simulink model "SIM_EXO_DAL_MN"  (R2021b)
(part 10 of 24)

t1657 = ct{497};
t1658 = ct{498};
t1659 = ct{499};
t166 = ct{500};
t1660 = ct{501};
t1661 = ct{502};
t1662 = ct{503};
t1663 = ct{504};
t1666 = ct{505};
t1669 = ct{506};
t1672 = ct{507};
t1676 = ct{508};
t1681 = ct{509};
t1682 = ct{510};
t1683 = ct{511};
t1687 = ct{512};
t1689 = ct{513};
t1692 = ct{514};
t1695 = ct{515};
t1696 = ct{516};
t1698 = ct{517};
t17 = ct{518};
t170 = ct{519};
t1702 = ct{520};
t1703 = ct{521};
t1704 = ct{522};
t1709 = ct{523};
t171 = ct{524};
t1711 = ct{525};
t1712 = ct{526};
t1713 = ct{527};
t1716 = ct{528};
t1720 = ct{529};
t1722 = ct{530};
t1726 = ct{531};
t1728 = ct{532};
t1729 = ct{533};
t173 = ct{534};
t1731 = ct{535};
t1733 = ct{536};
t1734 = ct{537};
t1735 = ct{538};
t1736 = ct{539};
t1737 = ct{540};
t1738 = ct{541};
t1740 = ct{542};
t1744 = ct{543};
t1745 = ct{544};
t1746 = ct{545};
t1749 = ct{546};
t175 = ct{547};
t1752 = ct{548};
t1755 = ct{549};
t1756 = ct{550};
t1757 = ct{551};
t1758 = ct{552};
t1760 = ct{553};
t1761 = ct{554};
t1764 = ct{555};
t1767 = ct{556};
t1769 = ct{557};
t177 = ct{558};
t1771 = ct{559};
t1772 = ct{560};
t1774 = ct{561};
t1776 = ct{562};
t1779 = ct{563};
t1784 = ct{564};
t1785 = ct{565};
t1786 = ct{566};
t1787 = ct{567};
t1788 = ct{568};
t1789 = ct{569};
t1793 = ct{570};
t1795 = ct{571};
t1797 = ct{572};
t1798 = ct{573};
t1799 = ct{574};
t18 = ct{575};
t1800 = ct{576};
t1801 = ct{577};
t1803 = ct{578};
t1804 = ct{579};
t1807 = ct{580};
t1808 = ct{581};
t1809 = ct{582};
t1810 = ct{583};
t1811 = ct{584};
t1812 = ct{585};
t1814 = ct{586};
t1816 = ct{587};
t1817 = ct{588};
t1820 = ct{589};
t1826 = ct{590};
t1827 = ct{591};
t1829 = ct{592};
t183 = ct{593};
t1830 = ct{594};
t1831 = ct{595};
t1832 = ct{596};
t1833 = ct{597};
t1834 = ct{598};
t1835 = ct{599};
t1836 = ct{600};
t1838 = ct{601};
t1847 = ct{602};
t1849 = ct{603};
t185 = ct{604};
t1850 = ct{605};
t1851 = ct{606};
t1855 = ct{607};
t1857 = ct{608};
t1858 = ct{609};
t1859 = ct{610};
t186 = ct{611};
t1866 = ct{612};
t1867 = ct{613};
t1871 = ct{614};
t1872 = ct{615};
t1873 = ct{616};
t1881 = ct{617};
t1882 = ct{618};
t1888 = ct{619};
t1889 = ct{620};
t1896 = ct{621};
t19 = ct{622};
t190 = ct{623};
t1903 = ct{624};
t1907 = ct{625};
t1908 = ct{626};
t191 = ct{627};
t1910 = ct{628};
t1911 = ct{629};
t1912 = ct{630};
t1913 = ct{631};
t1914 = ct{632};
t1915 = ct{633};
t1916 = ct{634};
t1920 = ct{635};
t1925 = ct{636};
t1926 = ct{637};
t193 = ct{638};
t1930 = ct{639};
t1935 = ct{640};
t1936 = ct{641};
t1937 = ct{642};
t1938 = ct{643};
t1939 = ct{644};
t194 = ct{645};
t1943 = ct{646};
t1944 = ct{647};
t1946 = ct{648};
t195 = ct{649};
t1950 = ct{650};
t1955 = ct{651};
t196 = ct{652};
t1961 = ct{653};
t1964 = ct{654};
t1965 = ct{655};
t1966 = ct{656};
t1967 = ct{657};
t1968 = ct{658};
t1969 = ct{659};
t197 = ct{660};
t1970 = ct{661};
t1972 = ct{662};
t1976 = ct{663};
t1977 = ct{664};
t1978 = ct{665};
t1979 = ct{666};
t1981 = ct{667};
t1984 = ct{668};
t1988 = ct{669};
t199 = ct{670};
t1992 = ct{671};
t1994 = ct{672};
t1995 = ct{673};
t1996 = ct{674};
t1997 = ct{675};
t1998 = ct{676};
t1999 = ct{677};
t2 = ct{678};
t20 = ct{679};
t200 = ct{680};
t2000 = ct{681};
t2001 = ct{682};
t2002 = ct{683};
t2003 = ct{684};
t2004 = ct{685};
t2005 = ct{686};
t2006 = ct{687};
t201 = ct{688};
t2014 = ct{689};
t2017 = ct{690};
t2019 = ct{691};
t202 = ct{692};
t2020 = ct{693};
t2023 = ct{694};
t2024 = ct{695};
t2028 = ct{696};
t2029 = ct{697};
t2033 = ct{698};
t2036 = ct{699};
t2037 = ct{700};
t2038 = ct{701};
t204 = ct{702};
t2042 = ct{703};
t205 = ct{704};
t2052 = ct{705};
t2053 = ct{706};
t2056 = ct{707};
t2058 = ct{708};
t2059 = ct{709};
t206 = ct{710};
t2060 = ct{711};
t2062 = ct{712};
t2065 = ct{713};
t2066 = ct{714};
t2067 = ct{715};
t2068 = ct{716};
t2069 = ct{717};
t207 = ct{718};
t2070 = ct{719};
t2072 = ct{720};
t2073 = ct{721};
t2074 = ct{722};
t2079 = ct{723};
t2081 = ct{724};
t2082 = ct{725};
t2083 = ct{726};
t2084 = ct{727};
t2085 = ct{728};
t2086 = ct{729};
t2087 = ct{730};
t2093 = ct{731};
t2094 = ct{732};
t2096 = ct{733};
t2097 = ct{734};
t2098 = ct{735};
t21 = ct{736};
t2100 = ct{737};
t2103 = ct{738};
t2104 = ct{739};
t2105 = ct{740};
t2106 = ct{741};
t2108 = ct{742};
t2109 = ct{743};
t2110 = ct{744};
t2111 = ct{745};
t2113 = ct{746};
t2114 = ct{747};
t2115 = ct{748};
t2116 = ct{749};
t2117 = ct{750};
t2118 = ct{751};
t2121 = ct{752};
t2122 = ct{753};
t2126 = ct{754};
t2128 = ct{755};
t2129 = ct{756};
t2130 = ct{757};
t2131 = ct{758};
t2132 = ct{759};
t2133 = ct{760};
t2136 = ct{761};
t2142 = ct{762};
t2144 = ct{763};
t2148 = ct{764};
t2149 = ct{765};
t215 = ct{766};
t2154 = ct{767};
t2156 = ct{768};
t2157 = ct{769};
t2158 = ct{770};
t2171 = ct{771};
t2172 = ct{772};
t2175 = ct{773};
t2176 = ct{774};
t2179 = ct{775};
t2180 = ct{776};
t2182 = ct{777};
t2189 = ct{778};
t2194 = ct{779};
t2196 = ct{780};
t22 = ct{781};
t2204 = ct{782};
t2208 = ct{783};
t2212 = ct{784};
t2214 = ct{785};
t2217 = ct{786};
t2218 = ct{787};
t2219 = ct{788};
t2220 = ct{789};
t2221 = ct{790};
t2223 = ct{791};
t2225 = ct{792};
t2227 = ct{793};
t2228 = ct{794};
t2229 = ct{795};
t2236 = ct{796};
t2239 = ct{797};
t224 = ct{798};
t2244 = ct{799};
t225 = ct{800};
t2251 = ct{801};
t2254 = ct{802};
t2256 = ct{803};
t2257 = ct{804};
t2264 = ct{805};
t2265 = ct{806};
t2266 = ct{807};
t2267 = ct{808};
t2269 = ct{809};
t227 = ct{810};
t2270 = ct{811};
t2274 = ct{812};
t2276 = ct{813};
t2277 = ct{814};
t2279 = ct{815};
t228 = ct{816};
t2280 = ct{817};
t2281 = ct{818};
t2282 = ct{819};
t2285 = ct{820};
t2291 = ct{821};
t2294 = ct{822};
t23 = ct{823};
t230 = ct{824};
t2302 = ct{825};
t2304 = ct{826};
t2305 = ct{827};
t2306 = ct{828};
t231 = ct{829};
t2316 = ct{830};
t2317 = ct{831};
t2318 = ct{832};
t2321 = ct{833};
t2322 = ct{834};
t2323 = ct{835};
t2324 = ct{836};
t233 = ct{837};
t2333 = ct{838};
t2336 = ct{839};
t2339 = ct{840};
t234 = ct{841};
t2340 = ct{842};
t2344 = ct{843};
t2348 = ct{844};
t235 = ct{845};
t2350 = ct{846};
t2357 = ct{847};
t2358 = ct{848};
t2359 = ct{849};
t236 = ct{850};
t2361 = ct{851};
t2362 = ct{852};
t2363 = ct{853};
t2364 = ct{854};
t2365 = ct{855};
t2366 = ct{856};
t2369 = ct{857};
t2371 = ct{858};
t2372 = ct{859};
t2373 = ct{860};
t2375 = ct{861};
t2376 = ct{862};
t2377 = ct{863};
t2378 = ct{864};
t2379 = ct{865};
t2384 = ct{866};
t2385 = ct{867};
t2387 = ct{868};
t2388 = ct{869};
t2389 = ct{870};
t239 = ct{871};
t2391 = ct{872};
t2394 = ct{873};
t24 = ct{874};
t240 = ct{875};
t2400 = ct{876};
t2401 = ct{877};
t2402 = ct{878};
t2403 = ct{879};
t2405 = ct{880};
t2406 = ct{881};
t2407 = ct{882};
t2410 = ct{883};
t2417 = ct{884};
t2418 = ct{885};
t2419 = ct{886};
t2421 = ct{887};
t2422 = ct{888};
t2428 = ct{889};
t2429 = ct{890};
t243 = ct{891};
t2430 = ct{892};
t2431 = ct{893};
t2434 = ct{894};
t2435 = ct{895};
t2437 = ct{896};
t2438 = ct{897};
t2439 = ct{898};
t244 = ct{899};
t2440 = ct{900};
t2441 = ct{901};
t2442 = ct{902};
t2443 = ct{903};
t2444 = ct{904};
t2447 = ct{905};
t2449 = ct{906};
t2450 = ct{907};
t2452 = ct{908};
t2453 = ct{909};
t2454 = ct{910};
t2455 = ct{911};
t2456 = ct{912};
t2457 = ct{913};
t2458 = ct{914};
t2460 = ct{915};
t2466 = ct{916};
t2467 = ct{917};
t2468 = ct{918};
t2470 = ct{919};
t2472 = ct{920};
t2474 = ct{921};
t2477 = ct{922};
t2481 = ct{923};
t2483 = ct{924};
t2484 = ct{925};
t2485 = ct{926};
t2486 = ct{927};
t2487 = ct{928};
t2489 = ct{929};
t249 = ct{930};
t2492 = ct{931};
t2495 = ct{932};
t2497 = ct{933};
t2498 = ct{934};
t2499 = ct{935};
t25 = ct{936};
t2500 = ct{937};
t2501 = ct{938};
t2502 = ct{939};
t2503 = ct{940};
t2504 = ct{941};
t2505 = ct{942};
t2506 = ct{943};
t2513 = ct{944};
t2518 = ct{945};
t2521 = ct{946};
t2527 = ct{947};
t2533 = ct{948};
t2535 = ct{949};
t2536 = ct{950};
t2537 = ct{951};
t2538 = ct{952};
t2540 = ct{953};
t2543 = ct{954};
t2544 = ct{955};
t2545 = ct{956};
t2546 = ct{957};
t2549 = ct{958};
t2551 = ct{959};
t2552 = ct{960};
t2553 = ct{961};
t2554 = ct{962};
t2555 = ct{963};
t2557 = ct{964};
t2558 = ct{965};
t2559 = ct{966};
t2560 = ct{967};
t2561 = ct{968};
t2562 = ct{969};
t2565 = ct{970};
t257 = ct{971};
t2572 = ct{972};
t2573 = ct{973};
t2574 = ct{974};
t2575 = ct{975};
t2576 = ct{976};
t2577 = ct{977};
t2578 = ct{978};
t2579 = ct{979};
t258 = ct{980};
t2583 = ct{981};
t2584 = ct{982};
t2590 = ct{983};
t2591 = ct{984};
t2592 = ct{985};
t2593 = ct{986};
t2595 = ct{987};
t2596 = ct{988};
t2597 = ct{989};
t26 = ct{990};
t2602 = ct{991};
t2603 = ct{992};
t2604 = ct{993};
t2605 = ct{994};
t2609 = ct{995};
t2610 = ct{996};
t2611 = ct{997};
t2615 = ct{998};
t2617 = ct{999};
t2627 = ct{1000};
t263 = ct{1001};
t2652 = ct{1002};
t2655 = ct{1003};
t2656 = ct{1004};
t266 = ct{1005};
t2673 = ct{1006};
t2675 = ct{1007};
t2676 = ct{1008};
t2685 = ct{1009};
t2687 = ct{1010};
t270 = ct{1011};
t2705 = ct{1012};
t2706 = ct{1013};
t2707 = ct{1014};
t2708 = ct{1015};
t2716 = ct{1016};
t2719 = ct{1017};
t273 = ct{1018};
t274 = ct{1019};
t2749 = ct{1020};
t275 = ct{1021};
t2751 = ct{1022};
t2752 = ct{1023};
t276 = ct{1024};
t2764 = ct{1025};
t277 = ct{1026};
t278 = ct{1027};
t280 = ct{1028};
t2804 = ct{1029};
t284 = ct{1030};
t2854 = ct{1031};
t287 = ct{1032};
t2886 = ct{1033};
t29 = ct{1034};
t290 = ct{1035};
t291 = ct{1036};
t292 = ct{1037};
t2939 = ct{1038};
t294 = ct{1039};
t297 = ct{1040};
t299 = ct{1041};
t2997 = ct{1042};
t3 = ct{1043};
t30 = ct{1044};
t300 = ct{1045};
t302 = ct{1046};
t303 = ct{1047};
t304 = ct{1048};
t305 = ct{1049};
t3058 = ct{1050};
t306 = ct{1051};
t309 = ct{1052};
t310 = ct{1053};
t311 = ct{1054};
t313 = ct{1055};
t314 = ct{1056};
t3142 = ct{1057};
t315 = ct{1058};
t3158 = ct{1059};
t316 = ct{1060};
t318 = ct{1061};
t319 = ct{1062};
t3191 = ct{1063};
t320 = ct{1064};
t3208 = ct{1065};
t3211 = ct{1066};
t3212 = ct{1067};
t3218 = ct{1068};
t3219 = ct{1069};
t322 = ct{1070};
t3225 = ct{1071};
t3228 = ct{1072};
t3230 = ct{1073};
t3231 = ct{1074};
t324 = ct{1075};
t3243 = ct{1076};
t3244 = ct{1077};
t325 = ct{1078};
t3251 = ct{1079};
t3252 = ct{1080};
t3255 = ct{1081};
t3257 = ct{1082};
t3258 = ct{1083};
t3259 = ct{1084};
t3261 = ct{1085};
t3273 = ct{1086};
t3274 = ct{1087};
t3275 = ct{1088};
t3279 = ct{1089};
t328 = ct{1090};
t3282 = ct{1091};
t3286 = ct{1092};
t3288 = ct{1093};
t3289 = ct{1094};
t3290 = ct{1095};
t3294 = ct{1096};
t3295 = ct{1097};
t3309 = ct{1098};
t3314 = ct{1099};
t3317 = ct{1100};
t3319 = ct{1101};
t3320 = ct{1102};
t3321 = ct{1103};
t3326 = ct{1104};
t3327 = ct{1105};
t3328 = ct{1106};
t3329 = ct{1107};
t333 = ct{1108};
t3330 = ct{1109};
t3331 = ct{1110};
t3333 = ct{1111};
t3334 = ct{1112};
t3335 = ct{1113};
t3343 = ct{1114};
t336 = ct{1115};
t3363 = ct{1116};
t3364 = ct{1117};
t3365 = ct{1118};
t3367 = ct{1119};
t3368 = ct{1120};
t3369 = ct{1121};
t337 = ct{1122};
t3370 = ct{1123};
t3371 = ct{1124};
t3372 = ct{1125};
t3373 = ct{1126};
t3374 = ct{1127};
t3375 = ct{1128};
t3376 = ct{1129};
t3378 = ct{1130};
t3379 = ct{1131};
t3380 = ct{1132};
t3381 = ct{1133};
t3382 = ct{1134};
t3389 = ct{1135};
t3390 = ct{1136};
t3391 = ct{1137};
t3392 = ct{1138};
t3393 = ct{1139};
t3394 = ct{1140};
t3395 = ct{1141};
t3397 = ct{1142};
t34 = ct{1143};
t340 = ct{1144};
t3400 = ct{1145};
t3401 = ct{1146};
t3402 = ct{1147};
t3403 = ct{1148};
t3409 = ct{1149};
t3416 = ct{1150};
t3417 = ct{1151};
t3418 = ct{1152};
t3419 = ct{1153};
t3420 = ct{1154};
t3426 = ct{1155};
t3430 = ct{1156};
t3432 = ct{1157};
t3434 = ct{1158};
t3435 = ct{1159};
t3437 = ct{1160};
t3438 = ct{1161};
t3439 = ct{1162};
t344 = ct{1163};
t3440 = ct{1164};
t3442 = ct{1165};
t3443 = ct{1166};
t3444 = ct{1167};
t3445 = ct{1168};
t3446 = ct{1169};
t3447 = ct{1170};
t3449 = ct{1171};
t3450 = ct{1172};
t3452 = ct{1173};
t3453 = ct{1174};
t3454 = ct{1175};
t3455 = ct{1176};
t3456 = ct{1177};
t3459 = ct{1178};
t346 = ct{1179};
t3462 = ct{1180};
t3463 = ct{1181};
t3466 = ct{1182};
t3468 = ct{1183};
t3469 = ct{1184};
t347 = ct{1185};
t3470 = ct{1186};
t3472 = ct{1187};
t3473 = ct{1188};
t3475 = ct{1189};
t3477 = ct{1190};
t3479 = ct{1191};
t348 = ct{1192};
t3481 = ct{1193};
t3483 = ct{1194};
t3486 = ct{1195};
t3489 = ct{1196};
t349 = ct{1197};
t3492 = ct{1198};
t350 = ct{1199};
t3500 = ct{1200};
t3501 = ct{1201};
t3506 = ct{1202};
t3507 = ct{1203};
t3509 = ct{1204};
t3514 = ct{1205};
t3515 = ct{1206};
t3516 = ct{1207};
t3517 = ct{1208};
t3519 = ct{1209};
t352 = ct{1210};
t3520 = ct{1211};
t3521 = ct{1212};
t3522 = ct{1213};
t3523 = ct{1214};
t3524 = ct{1215};
t353 = ct{1216};
t3530 = ct{1217};
t3532 = ct{1218};
t3533 = ct{1219};
t3534 = ct{1220};
t3535 = ct{1221};
t3538 = ct{1222};
t3539 = ct{1223};
t3541 = ct{1224};
t3544 = ct{1225};
t3546 = ct{1226};
t3548 = ct{1227};
t3549 = ct{1228};
t3553 = ct{1229};
t3556 = ct{1230};
t356 = ct{1231};
t3560 = ct{1232};
t3568 = ct{1233};
t3569 = ct{1234};
t357 = ct{1235};
t3572 = ct{1236};
t3573 = ct{1237};
t3574 = ct{1238};
t3575 = ct{1239};
t3576 = ct{1240};
t3578 = ct{1241};
t3579 = ct{1242};
t358 = ct{1243};
t3581 = ct{1244};
t3582 = ct{1245};
t3583 = ct{1246};
t3584 = ct{1247};
t3585 = ct{1248};
t359 = ct{1249};
t3590 = ct{1250};
t3596 = ct{1251};
t3597 = ct{1252};
t3601 = ct{1253};
t3602 = ct{1254};
t3604 = ct{1255};
t3607 = ct{1256};
t3609 = ct{1257};
t361 = ct{1258};
t3613 = ct{1259};
t3616 = ct{1260};
t3617 = ct{1261};
t3618 = ct{1262};
t362 = ct{1263};
t3622 = ct{1264};
t3629 = ct{1265};
t3630 = ct{1266};
t3637 = ct{1267};
t3638 = ct{1268};
t3639 = ct{1269};
t3641 = ct{1270};
t3643 = ct{1271};
t3646 = ct{1272};
t3647 = ct{1273};
t3649 = ct{1274};
t365 = ct{1275};
t3650 = ct{1276};
t3652 = ct{1277};
t3653 = ct{1278};
t3654 = ct{1279};
t3659 = ct{1280};
t3660 = ct{1281};
t3662 = ct{1282};
t3663 = ct{1283};
t3668 = ct{1284};
t3676 = ct{1285};
t368 = ct{1286};
t3680 = ct{1287};
t3682 = ct{1288};
t3686 = ct{1289};
t369 = ct{1290};
t3691 = ct{1291};
t3695 = ct{1292};
t3697 = ct{1293};
t3701 = ct{1294};
t3709 = ct{1295};
t371 = ct{1296};
t3714 = ct{1297};
t3716 = ct{1298};
t3717 = ct{1299};
t372 = ct{1300};
t3722 = ct{1301};
t3726 = ct{1302};
t3729 = ct{1303};
t373 = ct{1304};
t3730 = ct{1305};
t3736 = ct{1306};
t3737 = ct{1307};
t3738 = ct{1308};
t374 = ct{1309};
t3743 = ct{1310};
t3744 = ct{1311};
t3747 = ct{1312};
t3748 = ct{1313};
t3750 = ct{1314};
t3751 = ct{1315};
t3756 = ct{1316};
t377 = ct{1317};
t3774 = ct{1318};
t378 = ct{1319};
t3789 = ct{1320};
t379 = ct{1321};
t3798 = ct{1322};
t380 = ct{1323};
t3815 = ct{1324};
t382 = ct{1325};
t3822 = ct{1326};
t3824 = ct{1327};
t3825 = ct{1328};
t3834 = ct{1329};
t3835 = ct{1330};
t3839 = ct{1331};
t384 = ct{1332};
t3846 = ct{1333};
t3847 = ct{1334};
t3852 = ct{1335};
t386 = ct{1336};
t387 = ct{1337};
t388 = ct{1338};
t3889 = ct{1339};
t3892 = ct{1340};
t3898 = ct{1341};
t3899 = ct{1342};
t391 = ct{1343};
t3915 = ct{1344};
t392 = ct{1345};
t395 = ct{1346};
t3950 = ct{1347};
t3951 = ct{1348};
t3958 = ct{1349};
t3959 = ct{1350};
t396 = ct{1351};
t4 = ct{1352};
t400 = ct{1353};
t4001 = ct{1354};
t4002 = ct{1355};
t4004 = ct{1356};
t4007 = ct{1357};
t401 = ct{1358};
t402 = ct{1359};
t4028 = ct{1360};
t4029 = ct{1361};
t403 = ct{1362};
t4030 = ct{1363};
t4031 = ct{1364};
t4032 = ct{1365};
t4033 = ct{1366};
t4039 = ct{1367};
t4040 = ct{1368};
t4041 = ct{1369};
t4042 = ct{1370};
t4043 = ct{1371};
t4044 = ct{1372};
t4045 = ct{1373};
t4051 = ct{1374};
t4052 = ct{1375};
t4058 = ct{1376};
t406 = ct{1377};
t409 = ct{1378};
t410 = ct{1379};
t4105 = ct{1380};
t411 = ct{1381};
t4113 = ct{1382};
t4114 = ct{1383};
t4117 = ct{1384};
t4118 = ct{1385};
t412 = ct{1386};
t4123 = ct{1387};
t413 = ct{1388};
t414 = ct{1389};
t4143 = ct{1390};
t4144 = ct{1391};
t4145 = ct{1392};
t415 = ct{1393};
t4150 = ct{1394};
t4152 = ct{1395};
t4153 = ct{1396};
t4155 = ct{1397};
t416 = ct{1398};
t4160 = ct{1399};
t4164 = ct{1400};
t4165 = ct{1401};
t417 = ct{1402};
t4170 = ct{1403};
t4174 = ct{1404};
t4177 = ct{1405};
t4178 = ct{1406};
t4179 = ct{1407};
t418 = ct{1408};
t4180 = ct{1409};
t4181 = ct{1410};
t4182 = ct{1411};
t4183 = ct{1412};
t4184 = ct{1413};
t4185 = ct{1414};
t4186 = ct{1415};
t4187 = ct{1416};
t4188 = ct{1417};
t4189 = ct{1418};
t4190 = ct{1419};
t4191 = ct{1420};
t4192 = ct{1421};
t4193 = ct{1422};
t4194 = ct{1423};
t4196 = ct{1424};
t4197 = ct{1425};
t420 = ct{1426};
t4200 = ct{1427};
t4203 = ct{1428};
t4204 = ct{1429};
t4205 = ct{1430};
t4206 = ct{1431};
t4207 = ct{1432};
t4208 = ct{1433};
t4209 = ct{1434};
t4211 = ct{1435};
t4212 = ct{1436};
t4213 = ct{1437};
t4214 = ct{1438};
t4216 = ct{1439};
t422 = ct{1440};
t4221 = ct{1441};
t4228 = ct{1442};
t4229 = ct{1443};
t423 = ct{1444};
t4230 = ct{1445};
t4231 = ct{1446};
t4232 = ct{1447};
t4233 = ct{1448};
t4235 = ct{1449};
t4236 = ct{1450};
t4237 = ct{1451};
t4239 = ct{1452};
t424 = ct{1453};
t4240 = ct{1454};
t4242 = ct{1455};
t4243 = ct{1456};
t4246 = ct{1457};
t4249 = ct{1458};
t425 = ct{1459};
t4255 = ct{1460};
t4256 = ct{1461};
t4257 = ct{1462};
t4258 = ct{1463};
t4259 = ct{1464};
t4260 = ct{1465};
t4261 = ct{1466};
t4262 = ct{1467};
t4265 = ct{1468};
t4266 = ct{1469};
t4268 = ct{1470};
t427 = ct{1471};
t4271 = ct{1472};
t4272 = ct{1473};
t4275 = ct{1474};
t4277 = ct{1475};
t4278 = ct{1476};
t4279 = ct{1477};
t428 = ct{1478};
t4283 = ct{1479};
t4284 = ct{1480};
t4287 = ct{1481};
t4288 = ct{1482};
t4289 = ct{1483};
t429 = ct{1484};
t4290 = ct{1485};
t4292 = ct{1486};
t4293 = ct{1487};
t4294 = ct{1488};
t4295 = ct{1489};
t4296 = ct{1490};
t4297 = ct{1491};
t4298 = ct{1492};
t4299 = ct{1493};
t4300 = ct{1494};
t4301 = ct{1495};
t4304 = ct{1496};
t4308 = ct{1497};
t4309 = ct{1498};
t431 = ct{1499};
t4310 = ct{1500};
t4311 = ct{1501};
t4313 = ct{1502};
t4315 = ct{1503};
t4316 = ct{1504};
t4317 = ct{1505};
t4319 = ct{1506};
t432 = ct{1507};
t4320 = ct{1508};
t4321 = ct{1509};
t4323 = ct{1510};
t4325 = ct{1511};
t4326 = ct{1512};
t4328 = ct{1513};
t433 = ct{1514};
t4330 = ct{1515};
t4333 = ct{1516};
t4334 = ct{1517};
t4335 = ct{1518};
t4336 = ct{1519};
t4337 = ct{1520};
t4338 = ct{1521};
t4339 = ct{1522};
t434 = ct{1523};
t4341 = ct{1524};
t4342 = ct{1525};
t4343 = ct{1526};
t4344 = ct{1527};
t4345 = ct{1528};
t4346 = ct{1529};
t4347 = ct{1530};
t435 = ct{1531};
t4351 = ct{1532};
t4353 = ct{1533};
t4355 = ct{1534};
t436 = ct{1535};
t4361 = ct{1536};
t4365 = ct{1537};
t4367 = ct{1538};
t4369 = ct{1539};
t437 = ct{1540};
t4370 = ct{1541};
t4371 = ct{1542};
t4372 = ct{1543};
t4375 = ct{1544};
t4377 = ct{1545};
t4379 = ct{1546};
t438 = ct{1547};
t4382 = ct{1548};
t4385 = ct{1549};
t4387 = ct{1550};
t439 = ct{1551};
t4390 = ct{1552};
t4391 = ct{1553};
t4392 = ct{1554};
t4394 = ct{1555};
t4395 = ct{1556};
t4396 = ct{1557};
t4397 = ct{1558};
t44 = ct{1559};
t440 = ct{1560};
t4401 = ct{1561};
t4402 = ct{1562};
t4403 = ct{1563};
t4404 = ct{1564};
t4405 = ct{1565};
t4406 = ct{1566};
t4407 = ct{1567};
t4408 = ct{1568};
t441 = ct{1569};
t4410 = ct{1570};
t4411 = ct{1571};
t4412 = ct{1572};
t4413 = ct{1573};
t4417 = ct{1574};
t4419 = ct{1575};
t442 = ct{1576};
t4420 = ct{1577};
t4421 = ct{1578};
t4422 = ct{1579};
t4425 = ct{1580};
t4426 = ct{1581};
t4428 = ct{1582};
t4429 = ct{1583};
t4431 = ct{1584};
t4432 = ct{1585};
t4435 = ct{1586};
t4436 = ct{1587};
t444 = ct{1588};
t4440 = ct{1589};
t4442 = ct{1590};
t4443 = ct{1591};
t4444 = ct{1592};
t4445 = ct{1593};
t4446 = ct{1594};
t4448 = ct{1595};
t4449 = ct{1596};
t445 = ct{1597};
t4450 = ct{1598};
t4452 = ct{1599};
t4453 = ct{1600};
t4455 = ct{1601};
t4457 = ct{1602};
t4459 = ct{1603};
t4462 = ct{1604};
t4464 = ct{1605};
t4469 = ct{1606};
t4473 = ct{1607};
t4478 = ct{1608};
t4479 = ct{1609};
t448 = ct{1610};
t4480 = ct{1611};
t4481 = ct{1612};
t4483 = ct{1613};
t4484 = ct{1614};
t4485 = ct{1615};
t4486 = ct{1616};
t4488 = ct{1617};
t449 = ct{1618};
t4491 = ct{1619};
t4492 = ct{1620};
t4493 = ct{1621};
t4495 = ct{1622};
t4498 = ct{1623};
t45 = ct{1624};
t450 = ct{1625};
t4501 = ct{1626};
t4502 = ct{1627};
t4504 = ct{1628};
t4506 = ct{1629};
t4508 = ct{1630};
t4509 = ct{1631};
t4513 = ct{1632};
t4516 = ct{1633};
t4517 = ct{1634};
t4519 = ct{1635};
t452 = ct{1636};
t4520 = ct{1637};
t4522 = ct{1638};
t4524 = ct{1639};
t4525 = ct{1640};
t453 = ct{1641};
t4530 = ct{1642};
t4532 = ct{1643};
t4533 = ct{1644};
t454 = ct{1645};
t4540 = ct{1646};
t4542 = ct{1647};
t4543 = ct{1648};
t4547 = ct{1649};
t4548 = ct{1650};
t4549 = ct{1651};
t4551 = ct{1652};
t4554 = ct{1653};
t4555 = ct{1654};
t4557 = ct{1655};
t4558 = ct{1656};
t4559 = ct{1657};
t4561 = ct{1658};
t4562 = ct{1659};
t4563 = ct{1660};
t4566 = ct{1661};
t4567 = ct{1662};
t4568 = ct{1663};
t4569 = ct{1664};
t457 = ct{1665};
t4570 = ct{1666};
t4571 = ct{1667};
t4572 = ct{1668};
t4574 = ct{1669};
t4575 = ct{1670};
t4577 = ct{1671};
t4579 = ct{1672};
t458 = ct{1673};
t4581 = ct{1674};
t4582 = ct{1675};
t4583 = ct{1676};
t4584 = ct{1677};
t4588 = ct{1678};
t4589 = ct{1679};
t459 = ct{1680};
t4590 = ct{1681};
t4591 = ct{1682};
t4595 = ct{1683};
t4596 = ct{1684};
t46 = ct{1685};
t460 = ct{1686};
t4600 = ct{1687};
t4601 = ct{1688};
t4605 = ct{1689};
t4606 = ct{1690};
t4607 = ct{1691};
t461 = ct{1692};
t4611 = ct{1693};
t4614 = ct{1694};
t4616 = ct{1695};
t4617 = ct{1696};
t462 = ct{1697};
t4621 = ct{1698};
t4622 = ct{1699};
t4625 = ct{1700};
t4626 = ct{1701};
t4628 = ct{1702};
t4629 = ct{1703};
t463 = ct{1704};
t4630 = ct{1705};
t4632 = ct{1706};
t4633 = ct{1707};
t4634 = ct{1708};
t4636 = ct{1709};
t4637 = ct{1710};
t4638 = ct{1711};
t4639 = ct{1712};
t464 = ct{1713};
t4640 = ct{1714};
t4641 = ct{1715};
t4642 = ct{1716};
t4643 = ct{1717};
t4644 = ct{1718};
t4645 = ct{1719};
t4646 = ct{1720};
t4647 = ct{1721};
t4649 = ct{1722};
t465 = ct{1723};
t4650 = ct{1724};
t4651 = ct{1725};
t4652 = ct{1726};
t4653 = ct{1727};
t4656 = ct{1728};
t4657 = ct{1729};
t4658 = ct{1730};
t466 = ct{1731};
t4660 = ct{1732};
t4661 = ct{1733};
t4662 = ct{1734};
t4663 = ct{1735};
t4666 = ct{1736};
t4667 = ct{1737};
t4669 = ct{1738};
t4672 = ct{1739};
t4673 = ct{1740};
t4674 = ct{1741};
t4675 = ct{1742};
t468 = ct{1743};
t4688 = ct{1744};
t469 = ct{1745};
t4691 = ct{1746};
t4692 = ct{1747};
t4693 = ct{1748};
t4694 = ct{1749};
t4695 = ct{1750};
t4696 = ct{1751};
t4697 = ct{1752};
t47 = ct{1753};
t470 = ct{1754};
t4707 = ct{1755};
t4708 = ct{1756};
t4709 = ct{1757};
t471 = ct{1758};
t4711 = ct{1759};
t4713 = ct{1760};
t4716 = ct{1761};
t472 = ct{1762};
t4722 = ct{1763};
t4723 = ct{1764};
t4724 = ct{1765};
t4725 = ct{1766};
t4726 = ct{1767};
t4727 = ct{1768};
t4728 = ct{1769};
t4731 = ct{1770};
t4732 = ct{1771};
t4733 = ct{1772};
t4734 = ct{1773};
t4737 = ct{1774};
t4740 = ct{1775};
t4741 = ct{1776};
t4742 = ct{1777};
t4745 = ct{1778};
t4747 = ct{1779};
t4748 = ct{1780};
t4749 = ct{1781};
t475 = ct{1782};
t4752 = ct{1783};
t4753 = ct{1784};
t4754 = ct{1785};
t4755 = ct{1786};
t4756 = ct{1787};
t4758 = ct{1788};
t4759 = ct{1789};
t4760 = ct{1790};
t4761 = ct{1791};
t4763 = ct{1792};
t4766 = ct{1793};
t4769 = ct{1794};
t477 = ct{1795};
t4770 = ct{1796};
t4777 = ct{1797};
t4778 = ct{1798};
t4782 = ct{1799};
t4783 = ct{1800};
t4785 = ct{1801};
t4786 = ct{1802};
t4788 = ct{1803};
t4789 = ct{1804};
t479 = ct{1805};
t4790 = ct{1806};
t4794 = ct{1807};
t4795 = ct{1808};
t4796 = ct{1809};
t4797 = ct{1810};
t4798 = ct{1811};
t4799 = ct{1812};
t480 = ct{1813};
t4800 = ct{1814};
t4801 = ct{1815};
t4803 = ct{1816};
t4804 = ct{1817};
t4805 = ct{1818};
t4807 = ct{1819};
t4808 = ct{1820};
t481 = ct{1821};
t4811 = ct{1822};
t4813 = ct{1823};
t4814 = ct{1824};
t4815 = ct{1825};
t4818 = ct{1826};
t482 = ct{1827};
t4820 = ct{1828};
t4824 = ct{1829};
t4825 = ct{1830};
t4827 = ct{1831};
t4828 = ct{1832};
t483 = ct{1833};
t4830 = ct{1834};
t4832 = ct{1835};
t4833 = ct{1836};
t4834 = ct{1837};
t4835 = ct{1838};
t4837 = ct{1839};
t4839 = ct{1840};
t484 = ct{1841};
t4841 = ct{1842};
t4842 = ct{1843};
t4845 = ct{1844};
t4846 = ct{1845};
t4849 = ct{1846};
t485 = ct{1847};
t4852 = ct{1848};
t486 = ct{1849};
t4861 = ct{1850};
t4862 = ct{1851};
t4864 = ct{1852};
t4865 = ct{1853};
t4866 = ct{1854};
t4867 = ct{1855};
t4871 = ct{1856};
t4872 = ct{1857};
t4873 = ct{1858};
t4876 = ct{1859};
t4877 = ct{1860};
t4878 = ct{1861};
t4879 = ct{1862};
t488 = ct{1863};
t4882 = ct{1864};
t4883 = ct{1865};
t4884 = ct{1866};
t4886 = ct{1867};
t4887 = ct{1868};
t489 = ct{1869};
t4895 = ct{1870};
t4897 = ct{1871};
t4899 = ct{1872};
t4900 = ct{1873};
t4908 = ct{1874};
t4909 = ct{1875};
t491 = ct{1876};
t4910 = ct{1877};
t4911 = ct{1878};
t4913 = ct{1879};
t4915 = ct{1880};
t4916 = ct{1881};
t4919 = ct{1882};
t492 = ct{1883};
t4920 = ct{1884};
t4923 = ct{1885};
t4924 = ct{1886};
t4925 = ct{1887};
t4927 = ct{1888};
t4928 = ct{1889};
t493 = ct{1890};
t4930 = ct{1891};
t4933 = ct{1892};
t4934 = ct{1893};
t4937 = ct{1894};
t4938 = ct{1895};
t494 = ct{1896};
t4941 = ct{1897};
t4942 = ct{1898};
t4943 = ct{1899};
t4944 = ct{1900};
t4945 = ct{1901};
t4946 = ct{1902};
t4948 = ct{1903};
t4951 = ct{1904};
t4955 = ct{1905};
t4956 = ct{1906};
t4957 = ct{1907};
t496 = ct{1908};
t4962 = ct{1909};
t4964 = ct{1910};
t4969 = ct{1911};
t497 = ct{1912};
t4970 = ct{1913};
t4973 = ct{1914};
t4974 = ct{1915};
t4976 = ct{1916};
t498 = ct{1917};
t4980 = ct{1918};
t4981 = ct{1919};
t4982 = ct{1920};
t4983 = ct{1921};
t4986 = ct{1922};
t4987 = ct{1923};
t4988 = ct{1924};
t499 = ct{1925};
t4991 = ct{1926};
t4993 = ct{1927};
t4996 = ct{1928};
t4998 = ct{1929};
t4999 = ct{1930};
t5 = ct{1931};
t50 = ct{1932};
t500 = ct{1933};
t5000 = ct{1934};
t5001 = ct{1935};
t5004 = ct{1936};
t5006 = ct{1937};
t5008 = ct{1938};
t501 = ct{1939};
t5019 = ct{1940};
t502 = ct{1941};
t5021 = ct{1942};
t5022 = ct{1943};
t5023 = ct{1944};
t5026 = ct{1945};
t5027 = ct{1946};
t5029 = ct{1947};
t503 = ct{1948};
t5034 = ct{1949};
t5035 = ct{1950};
t5036 = ct{1951};
t5038 = ct{1952};
t504 = ct{1953};
t5045 = ct{1954};
t5046 = ct{1955};
t505 = ct{1956};
t5051 = ct{1957};
t5052 = ct{1958};
t5053 = ct{1959};
t506 = ct{1960};
t5060 = ct{1961};
t5062 = ct{1962};
t5063 = ct{1963};
t5064 = ct{1964};
t5065 = ct{1965};
t5066 = ct{1966};
t5069 = ct{1967};
t507 = ct{1968};
t5071 = ct{1969};
t5072 = ct{1970};
t5073 = ct{1971};
t5078 = ct{1972};
t508 = ct{1973};
t5080 = ct{1974};
t5082 = ct{1975};
t5083 = ct{1976};
t5084 = ct{1977};
t5085 = ct{1978};
t509 = ct{1979};
t5091 = ct{1980};
t5093 = ct{1981};
t5095 = ct{1982};
t5096 = ct{1983};
t5097 = ct{1984};
t5098 = ct{1985};
t5099 = ct{1986};
t510 = ct{1987};
t5100 = ct{1988};
t5102 = ct{1989};
t5107 = ct{1990};
t511 = ct{1991};
t5111 = ct{1992};
t5112 = ct{1993};
t5113 = ct{1994};
t5114 = ct{1995};
t5116 = ct{1996};
t5119 = ct{1997};
t512 = ct{1998};
t5120 = ct{1999};
t5122 = ct{2000};
t5127 = ct{2001};
t513 = ct{2002};
t5130 = ct{2003};
t5139 = ct{2004};
t514 = ct{2005};
t5142 = ct{2006};
t5147 = ct{2007};
t5149 = ct{2008};
t5150 = ct{2009};
t5151 = ct{2010};
t5154 = ct{2011};
t5158 = ct{2012};
t516 = ct{2013};
t5165 = ct{2014};
t517 = ct{2015};
t5171 = ct{2016};
t5172 = ct{2017};
t5176 = ct{2018};
t5179 = ct{2019};
t518 = ct{2020};
t5180 = ct{2021};
t5181 = ct{2022};
t5183 = ct{2023};
t5184 = ct{2024};
t5185 = ct{2025};
t5186 = ct{2026};
t5187 = ct{2027};
t5192 = ct{2028};
t5193 = ct{2029};
t5199 = ct{2030};
t520 = ct{2031};
t5200 = ct{2032};
t5203 = ct{2033};
t5204 = ct{2034};
t5205 = ct{2035};
t5208 = ct{2036};
t521 = ct{2037};
t5215 = ct{2038};
t5216 = ct{2039};
t5217 = ct{2040};
t522 = ct{2041};
t5222 = ct{2042};
t5223 = ct{2043};
t5224 = ct{2044};
t5227 = ct{2045};
t523 = ct{2046};
t5236 = ct{2047};
t5237 = ct{2048};
t5238 = ct{2049};
t5239 = ct{2050};
t524 = ct{2051};
t5240 = ct{2052};
t5244 = ct{2053};
t5245 = ct{2054};
t525 = ct{2055};
t5250 = ct{2056};
t5252 = ct{2057};
t5258 = ct{2058};
t526 = ct{2059};
t5267 = ct{2060};
t527 = ct{2061};
t5270 = ct{2062};
t5271 = ct{2063};
t5279 = ct{2064};
t528 = ct{2065};
t5280 = ct{2066};
t5281 = ct{2067};
t5285 = ct{2068};
t529 = ct{2069};
t5293 = ct{2070};
t5294 = ct{2071};
t53 = ct{2072};
t530 = ct{2073};
t5305 = ct{2074};
t531 = ct{2075};
t5318 = ct{2076};
t5319 = ct{2077};
t532 = ct{2078};
t5321 = ct{2079};
t5324 = ct{2080};
t5325 = ct{2081};
t5327 = ct{2082};
t5328 = ct{2083};
t533 = ct{2084};
t5331 = ct{2085};
t5332 = ct{2086};
t534 = ct{2087};
t535 = ct{2088};
t5353 = ct{2089};
t5355 = ct{2090};
t5356 = ct{2091};
t5358 = ct{2092};
t536 = ct{2093};
t5361 = ct{2094};
t5362 = ct{2095};
t5364 = ct{2096};
t5368 = ct{2097};
t537 = ct{2098};
t5372 = ct{2099};
t5373 = ct{2100};
t5376 = ct{2101};
t5378 = ct{2102};
t538 = ct{2103};
t5387 = ct{2104};
t5389 = ct{2105};
t539 = ct{2106};
t5390 = ct{2107};
t5391 = ct{2108};
t5392 = ct{2109};
t5393 = ct{2110};
t5394 = ct{2111};
t540 = ct{2112};
t5402 = ct{2113};
t5404 = ct{2114};
t5409 = ct{2115};
t5416 = ct{2116};
t5420 = ct{2117};
t5424 = ct{2118};
t5429 = ct{2119};
t543 = ct{2120};
t5430 = ct{2121};
t5434 = ct{2122};
t5435 = ct{2123};
t5436 = ct{2124};
t5439 = ct{2125};
t544 = ct{2126};
t5440 = ct{2127};
t5441 = ct{2128};
t5445 = ct{2129};
t5449 = ct{2130};
t545 = ct{2131};
t5450 = ct{2132};
t5451 = ct{2133};
t5452 = ct{2134};
t5453 = ct{2135};
t5455 = ct{2136};
t5456 = ct{2137};
t5457 = ct{2138};
t546 = ct{2139};
t5467 = ct{2140};
t5468 = ct{2141};
t5469 = ct{2142};
t547 = ct{2143};
t5470 = ct{2144};
t5471 = ct{2145};
t5472 = ct{2146};
t5473 = ct{2147};
t5474 = ct{2148};
t5475 = ct{2149};
t5476 = ct{2150};
t5477 = ct{2151};
t5478 = ct{2152};
t548 = ct{2153};
t5489 = ct{2154};
t549 = ct{2155};
t5490 = ct{2156};
t5493 = ct{2157};
t5494 = ct{2158};
t5497 = ct{2159};
t5499 = ct{2160};
t5501 = ct{2161};
t5508 = ct{2162};
t551 = ct{2163};
t5510 = ct{2164};
t5512 = ct{2165};
t5516 = ct{2166};
t5517 = ct{2167};
t552 = ct{2168};
t5521 = ct{2169};
t553 = ct{2170};
t5532 = ct{2171};
t5535 = ct{2172};
t554 = ct{2173};
t5540 = ct{2174};
t5547 = ct{2175};
t555 = ct{2176};
t5557 = ct{2177};
t5558 = ct{2178};
t556 = ct{2179};
t557 = ct{2180};
t5574 = ct{2181};
t5578 = ct{2182};
t5579 = ct{2183};
t558 = ct{2184};
t5582 = ct{2185};
t5586 = ct{2186};
t559 = ct{2187};
t5590 = ct{2188};
t5593 = ct{2189};
t5596 = ct{2190};
t560 = ct{2191};
t5604 = ct{2192};
t5607 = ct{2193};
t561 = ct{2194};
t5612 = ct{2195};
t562 = ct{2196};
t5629 = ct{2197};
t563 = ct{2198};
t5634 = ct{2199};
t5635 = ct{2200};
t564 = ct{2201};
t567 = ct{2202};
t568 = ct{2203};
t5688 = ct{2204};
t569 = ct{2205};
t57 = ct{2206};
t570 = ct{2207};
t571 = ct{2208};
t572 = ct{2209};
t573 = ct{2210};
t574 = ct{2211};
t5741 = ct{2212};
t5743 = ct{2213};
t576 = ct{2214};
t577 = ct{2215};
t5777 = ct{2216};
t5779 = ct{2217};
t578 = ct{2218};
t5780 = ct{2219};
t5782 = ct{2220};
t579 = ct{2221};
t58 = ct{2222};
t580 = ct{2223};
t581 = ct{2224};
t582 = ct{2225};
t5826 = ct{2226};
t583 = ct{2227};
t584 = ct{2228};
t586 = ct{2229};
t587 = ct{2230};
t5886 = ct{2231};
t5887 = ct{2232};
t589 = ct{2233};
t5894 = ct{2234};
t59 = ct{2235};
t590 = ct{2236};
t591 = ct{2237};
t592 = ct{2238};
t593 = ct{2239};
t594 = ct{2240};
t595 = ct{2241};
t596 = ct{2242};
t597 = ct{2243};
t6 = ct{2244};
t60 = ct{2245};
t600 = ct{2246};
t602 = ct{2247};
t603 = ct{2248};
t604 = ct{2249};
t605 = ct{2250};
t609 = ct{2251};
t610 = ct{2252};
t611 = ct{2253};
t612 = ct{2254};
t613 = ct{2255};
t614 = ct{2256};
t615 = ct{2257};
t616 = ct{2258};
t618 = ct{2259};
t619 = ct{2260};
t622 = ct{2261};
t623 = ct{2262};
t624 = ct{2263};
t625 = ct{2264};
t626 = ct{2265};
t627 = ct{2266};
t628 = ct{2267};
t629 = ct{2268};
t63 = ct{2269};
t630 = ct{2270};
t631 = ct{2271};
t633 = ct{2272};
t634 = ct{2273};
t635 = ct{2274};
t636 = ct{2275};
t637 = ct{2276};
t638 = ct{2277};
t639 = ct{2278};
t640 = ct{2279};
t641 = ct{2280};
t642 = ct{2281};
t643 = ct{2282};
t648 = ct{2283};
t649 = ct{2284};
t650 = ct{2285};
t653 = ct{2286};
t654 = ct{2287};
t655 = ct{2288};
t656 = ct{2289};
t657 = ct{2290};
t658 = ct{2291};
t660 = ct{2292};
t662 = ct{2293};
t663 = ct{2294};
t664 = ct{2295};
t665 = ct{2296};
t667 = ct{2297};
t668 = ct{2298};
t673 = ct{2299};
t674 = ct{2300};
t675 = ct{2301};
t676 = ct{2302};
t678 = ct{2303};
t679 = ct{2304};
t681 = ct{2305};
t682 = ct{2306};
t683 = ct{2307};
t684 = ct{2308};
t685 = ct{2309};
t686 = ct{2310};
t687 = ct{2311};
t688 = ct{2312};
t689 = ct{2313};
t693 = ct{2314};
t694 = ct{2315};
t695 = ct{2316};
t696 = ct{2317};
t697 = ct{2318};
t698 = ct{2319};
t7 = ct{2320};
t700 = ct{2321};
t702 = ct{2322};
t703 = ct{2323};
t704 = ct{2324};
t705 = ct{2325};
t706 = ct{2326};
t71 = ct{2327};
t710 = ct{2328};
t711 = ct{2329};
t712 = ct{2330};
t713 = ct{2331};
t715 = ct{2332};
t716 = ct{2333};
t72 = ct{2334};
t724 = ct{2335};
t728 = ct{2336};
t73 = ct{2337};
t731 = ct{2338};
t733 = ct{2339};
t734 = ct{2340};
t735 = ct{2341};
t736 = ct{2342};
t74 = ct{2343};
t741 = ct{2344};
t742 = ct{2345};
t743 = ct{2346};
t744 = ct{2347};
t746 = ct{2348};
t747 = ct{2349};
t748 = ct{2350};
t749 = ct{2351};
t75 = ct{2352};
t750 = ct{2353};
t751 = ct{2354};
t752 = ct{2355};
t754 = ct{2356};
t755 = ct{2357};
t756 = ct{2358};
t757 = ct{2359};
t758 = ct{2360};
t759 = ct{2361};
t76 = ct{2362};
t760 = ct{2363};
t762 = ct{2364};
t763 = ct{2365};
t764 = ct{2366};
t765 = ct{2367};
t766 = ct{2368};
t767 = ct{2369};
t768 = ct{2370};
t769 = ct{2371};
t77 = ct{2372};
t772 = ct{2373};
t773 = ct{2374};
t774 = ct{2375};
t775 = ct{2376};
t776 = ct{2377};
t777 = ct{2378};
t778 = ct{2379};
t779 = ct{2380};
t780 = ct{2381};
t781 = ct{2382};
t782 = ct{2383};
t784 = ct{2384};
t785 = ct{2385};
t786 = ct{2386};
t790 = ct{2387};
t792 = ct{2388};
t794 = ct{2389};
t795 = ct{2390};
t796 = ct{2391};
t798 = ct{2392};
t8 = ct{2393};
t80 = ct{2394};
t801 = ct{2395};
t804 = ct{2396};
t805 = ct{2397};
t806 = ct{2398};
t808 = ct{2399};
t81 = ct{2400};
t814 = ct{2401};
t815 = ct{2402};
t817 = ct{2403};
t82 = ct{2404};
t820 = ct{2405};
t822 = ct{2406};
t825 = ct{2407};
t827 = ct{2408};
t83 = ct{2409};
t831 = ct{2410};
t832 = ct{2411};
t833 = ct{2412};
t834 = ct{2413};
t835 = ct{2414};
t836 = ct{2415};
t837 = ct{2416};
t838 = ct{2417};
t84 = ct{2418};
t840 = ct{2419};
t841 = ct{2420};
t842 = ct{2421};
t843 = ct{2422};
t846 = ct{2423};
t86 = ct{2424};
t863 = ct{2425};
t868 = ct{2426};
t869 = ct{2427};
t870 = ct{2428};
t874 = ct{2429};
t878 = ct{2430};
t880 = ct{2431};
t881 = ct{2432};
t882 = ct{2433};
t884 = ct{2434};
t885 = ct{2435};
t888 = ct{2436};
t889 = ct{2437};
t891 = ct{2438};
t892 = ct{2439};
t895 = ct{2440};
t897 = ct{2441};
t899 = ct{2442};
t9 = ct{2443};
t90 = ct{2444};
t900 = ct{2445};
t903 = ct{2446};
t906 = ct{2447};
t91 = ct{2448};
t911 = ct{2449};
t921 = ct{2450};
t922 = ct{2451};
t923 = ct{2452};
t925 = ct{2453};
t926 = ct{2454};
t927 = ct{2455};
t929 = ct{2456};
t934 = ct{2457};
t935 = ct{2458};
t936 = ct{2459};
t937 = ct{2460};
t940 = ct{2461};
t941 = ct{2462};
t942 = ct{2463};
t946 = ct{2464};
t949 = ct{2465};
t95 = ct{2466};
t950 = ct{2467};
t954 = ct{2468};
t955 = ct{2469};
t956 = ct{2470};
t957 = ct{2471};
t958 = ct{2472};
t961 = ct{2473};
t962 = ct{2474};
t964 = ct{2475};
t965 = ct{2476};
t966 = ct{2477};
t968 = ct{2478};
t969 = ct{2479};
t97 = ct{2480};
t970 = ct{2481};
t971 = ct{2482};
t972 = ct{2483};
t973 = ct{2484};
t975 = ct{2485};
t977 = ct{2486};
t979 = ct{2487};
t982 = ct{2488};
t983 = ct{2489};
t984 = ct{2490};
t986 = ct{2491};
t987 = ct{2492};
t988 = ct{2493};
t989 = ct{2494};
t99 = ct{2495};
t993 = ct{2496};
t994 = ct{2497};
t995 = ct{2498};
t999 = ct{2499};
t1551 = t5.*t196.*(-4.097607815548108e-7);
t1553 = -t1528;
t1557 = t8.*t1514;
t1572 = t8.*t194.*t240;
t1573 = t8.*t195.*t240;
t1574 = -t1541;
t1575 = t4.*t195.*(-8.987911871652987e-9);
t1578 = -t1545;
t1581 = -t1548;
t1590 = t19.*t196.*4.188279553614573e-7;
t1592 = -t1555;
t1594 = -t1556;
t1607 = t18.*t196.*4.265809185498476e-7;
t1609 = t23.*t196.*4.265809185498476e-7;
t1613 = -t1569;
t1614 = t196.*6.684964735994217e-8;
t1615 = t22.*t1514;
t1617 = -t1570;
t1618 = t8.*t9.*t195.*(-4.097607815548108e-7);
t1624 = t8.*t1545;
t1627 = t9.*t196.*(-2.227142959217101e-7);
t1630 = t5.*t9.*t196.*6.371903244127231e-7;
t1642 = t7.*t9.*t196.*6.892170885479394e-7;
t1646 = t5.*t8.*t9.*t194.*8.376559107229145e-7;
t1649 = t5.*t8.*t9.*t195.*8.376559107229145e-7;
t1665 = t3.*t5.*t7.*t194.*8.195215631096216e-7;
t1670 = t3.*t4.*t640.*4.297799892626299e-1;
t1671 = t3.*t5.*t7.*t195.*8.195215631096216e-7;
t1673 = t17.*t1514;
t1674 = t18.*t1514;
t1697 = -t1621;
t1705 = -t1623;
t1706 = t7.*t196.*2.909656073620116e-9;
t1719 = t5.*t7.*t9.*t196.*2.817872251232979e-6;
t1724 = -t1650;
t1730 = t8.*t194.*t278;
t1739 = t8.*t195.*t278;
t1743 = t9.*t197.*1.608000198040319e-13;
t1748 = -t1672;
t1759 = t5.*t7.*t196.*3.746051489620971e-7;
t1763 = -t1687;
t1770 = t7.*t19.*t196.*2.143506553146841e-6;
t1773 = t8.*t9.*t17.*t194.*8.195215631096216e-7;
t1775 = t7.*t24.*t196.*2.143506553146841e-6;
t1780 = t8.*t9.*t17.*t195.*8.195215631096216e-7;
t1782 = t8.*t19.*t194.*1.274380648825446e-6;
t1783 = t7.*t18.*t196.*6.267441153167058e-7;
t1791 = t8.*t19.*t195.*1.274380648825446e-6;
t1792 = t7.*t23.*t196.*6.267441153167058e-7;
t1802 = t4.*t17.*t194.*1.797582374330597e-8;
t1806 = t17.*t1542;
t1813 = t4.*t17.*t195.*1.797582374330597e-8;
t1818 = t194.*t401;
t1822 = t17.*t1545;
t1823 = t18.*t1545;
t1824 = t195.*t401;
t1825 = t3.*t7.*t9.*t194.*4.454285918434201e-7;
t1828 = t22.*t1545;
t1837 = t3.*t7.*t9.*t195.*4.454285918434201e-7;
t1839 = t5.*t196.*8.040000990201593e-14;
t1844 = t5.*t8.*t194.*(-2.227142959217101e-7);
t1854 = t9.*t197.*8.040000990201593e-14;
t1862 = t3.*t7.*t19.*t194.*1.675311821445829e-6;
t1864 = t194.*t378;
t1865 = t3.*t7.*t19.*t195.*1.675311821445829e-6;
t1869 = t195.*t378;
t1875 = t194.*t409;
t1877 = t8.*t194.*6.359001115808088e-7;
t1879 = t195.*t409;
t1880 = t8.*t195.*6.359001115808088e-7;
t1884 = t17.*t1571;
t1887 = -t1776;
t1892 = -t1784;
t1893 = t17.*t194.*1.72988013006783e-9;
t1904 = t17.*t195.*1.72988013006783e-9;
t1906 = -t1803;
t1909 = -t1808;
t1919 = t7.*t8.*t194.*(-1.511765579126689e-8);
t1921 = -t1820;
t1971 = t4.*t7.*t9.*t195.*(-6.892170885479394e-7);
t1973 = t5.*t8.*t17.*t195.*4.454285918434201e-7;
t1980 = t194.*t437;
t1993 = -t1888;
t2008 = t8.*t1811;
t2009 = t194.*t450;
t2016 = t195.*t450;
t2021 = t4.*t7.*t19.*t194.*2.143506553146841e-6;
t2040 = t4.*t7.*t19.*t195.*2.143506553146841e-6;
t2041 = t3.*t4.*t5.*t8.*t194.*1.378434177095879e-6;
t2044 = t3.*t5.*t7.*t9.*t194.*2.548761297650892e-6;
t2047 = t196.*1.192135723313091e-6;
t2051 = t3.*t4.*t5.*t8.*t195.*1.378434177095879e-6;
t2054 = t3.*t5.*t7.*t9.*t195.*2.548761297650892e-6;
t2055 = t5.*t8.*t9.*t17.*t194.*1.675311821445829e-6;
t2057 = t18.*t19.*t196.*(-4.188279553614573e-7);
t2061 = t5.*t8.*t9.*t17.*t195.*1.675311821445829e-6;
t2071 = t4.*t5.*t7.*t9.*t194.*1.408936125616489e-6;
t2076 = -t1964;
t2077 = -t1965;
t2078 = t5.*t8.*t17.*t194.*4.454285918434201e-7;
t2080 = t4.*t5.*t7.*t9.*t195.*1.408936125616489e-6;
t2088 = t7.*t34.*t91.*t191;
t2089 = -t1972;
t2091 = t197.*t481;
t2092 = t9.*t18.*t197.*3.216000396080637e-13;
t2095 = t3.*t5.*t7.*t18.*t195.*(-8.195215631096216e-7);
t2099 = t194.*t472;
t2101 = -t2002;
t2102 = t195.*t472;
t2107 = t4.*t5.*t7.*t194.*(-3.746051489620971e-7);
t2119 = -t2014;
t2125 = -t2017;
t2135 = t5.*t9.*t18.*t196.*(-6.371903244127231e-7);
t2139 = t9.*t196.*1.054342951111095e-13;
t2140 = t5.*t197.*1.054342951111095e-13;
t2141 = t5.*t197.*2.10868590222219e-13;
t2147 = t4.*t9.*t1687;
t2150 = t5.*t18.*t196.*1.608000198040319e-13;
t2151 = t3.*t34.*t91.*t191;
t2155 = t8.*t195.*t436;
t2159 = t3.*t7.*t18.*t19.*t194.*8.376559107229145e-7;
t2162 = t3.*t7.*t18.*t19.*t195.*8.376559107229145e-7;
t2163 = t3.*t4.*t8.*t19.*t194.*1.408936125616489e-6;
t2166 = t3.*t4.*t8.*t19.*t195.*1.408936125616489e-6;
t2167 = t3.*t4.*t8.*t9.*t194.*7.492102979241942e-7;
t2168 = t8.*t17.*t194.*1.271800223161618e-6;
t2169 = t3.*t4.*t8.*t9.*t195.*7.492102979241942e-7;
t2170 = t3.*t9.*t195.*(-2.7046541903611e-13);
t2174 = t8.*t17.*t195.*1.271800223161618e-6;
t2177 = t7.*t18.*t19.*t196.*1.07175327657342e-6;
t2178 = t17.*t1772;
t2184 = t7.*t18.*t24.*t196.*1.07175327657342e-6;
t2185 = t22.*t1772;
t2186 = -t2122;
t2187 = t18.*t196.*1.508157382287566e-7;
t2190 = t8.*t17.*t19.*t194.*2.548761297650892e-6;
t2191 = -t2126;
t2192 = t23.*t196.*1.508157382287566e-7;
t2195 = t8.*t17.*t19.*t195.*2.548761297650892e-6;
t2200 = t17.*t1812;
t2201 = t4.*t7.*t194.*1.069583140309415e-6;
t2203 = t5.*t7.*t9.*t18.*t196.*1.408936125616489e-6;
t2209 = t22.*t1812;
t2210 = t4.*t7.*t195.*1.069583140309415e-6;
t2226 = t8.*t194.*t436;
t2231 = -t2154;
t2232 = t194.*t538;
t2235 = t195.*t538;
t2237 = t5.*t17.*t1687;
t2240 = t194.*t544;
t2243 = t5.*t7.*t18.*t196.*(-3.746051489620971e-7);
t2245 = t195.*t544;
t2246 = t4.*t5.*t17.*t194.*3.216000396080637e-13;
t2249 = t3.*t7.*t194.*2.026204524882102e-6;
t2250 = t4.*t5.*t17.*t195.*3.216000396080637e-13;
t2252 = t3.*t7.*t195.*2.026204524882102e-6;
t2255 = t4.*t5.*t1946;
t2271 = t3.*t7.*t9.*t18.*t195.*(-4.454285918434201e-7);
t2272 = t194.*t527;
t2273 = t3.*t4.*t5.*t8.*t9.*t194.*(-2.143506553146841e-6);
t2275 = t195.*t527;
t2278 = t4.*t9.*t195.*(-2.10868590222219e-13);
t2283 = t3.*t4.*t8.*t194.*5.073437414621283e-7;
t2284 = -t2244;
t2286 = t5.*t7.*t8.*t195.*(-2.7046541903611e-13);
t2287 = t3.*t4.*t8.*t195.*5.073437414621283e-7;
t2292 = t3.*t9.*t18.*t194.*5.4093083807222e-13;
t2295 = t3.*t9.*t18.*t195.*5.4093083807222e-13;
t2307 = t3.*t5.*t7.*t9.*t18.*t194.*1.274380648825446e-6;
t2308 = t5.*t18.*t197.*4.217371804444381e-13;
t2309 = t3.*t5.*t7.*t9.*t18.*t195.*1.274380648825446e-6;
t2310 = t3.*t5.*t195.*(-3.546806877605634e-13);
t2311 = t195.*t572;
t2312 = t7.*t9.*t18.*t196.*2.7046541903611e-13;
t2314 = t7.*t9.*t23.*t196.*2.7046541903611e-13;
t2331 = t17.*t2122;
t2334 = t22.*t2122;
t2335 = t3.*t4.*t7.*t8.*t9.*t194.*3.216000396080637e-13;
t2337 = t3.*t4.*t7.*t8.*t9.*t195.*3.216000396080637e-13;
t2338 = t9.*t17.*t1946;
t2341 = t9.*t18.*t196.*2.10868590222219e-13;
t2342 = t197.*t582;
t2343 = t194.*t572;
t2347 = t22.*t2214;
t2351 = t4.*t9.*t17.*t194.*4.217371804444381e-13;
t2355 = t4.*t9.*t17.*t195.*4.217371804444381e-13;
t2368 = t3.*t7.*t18.*t194.*3.016314764575132e-7;
t2370 = t3.*t7.*t18.*t195.*3.016314764575132e-7;
t2374 = t194.*t595;
t2381 = t3.*t5.*t18.*t194.*7.093613755211269e-13;
t2382 = t3.*t5.*t18.*t195.*7.093613755211269e-13;
t2390 = (t9.*t2096)./2.0;
t2392 = t5.*t7.*t18.*t196.*3.546806877605634e-13;
t2395 = (t5.*t2121)./2.0;
t2396 = t197.*1.863093161453879e-7;
t2397 = t5.*t7.*t23.*t196.*3.546806877605634e-13;
t2423 = t3.*t4.*t5.*t7.*t8.*t194.*4.217371804444381e-13;
t2425 = t3.*t4.*t5.*t7.*t8.*t195.*4.217371804444381e-13;
t2427 = t22.*t2291;
t2445 = -t2419;
t2446 = -t2421;
t2459 = t4.*t2418;
t2461 = t8.*t2418;
t2462 = t4.*t2419;
t2463 = t8.*t2419;
t2464 = -t2444;
t2469 = -t2447;
t2471 = t18.*t197.*7.452372645815517e-7;
t2478 = -t2468;
t2480 = t18.*t197.*3.726186322907759e-7;
t2482 = t18.*t197.*7.452373075881582e-7;
t2507 = -t2492;
t2508 = t3.*t18.*t194.*1.253488085959302e-6;
t2509 = t3.*t18.*t195.*1.253488085959302e-6;
t2510 = t4.*t5.*t2467;
t2511 = t4.*t9.*t2467;
t2512 = t4.*t5.*t2468;
t2514 = t4.*t9.*t2468;
t2515 = t5.*t8.*t2468;
t2517 = t8.*t9.*t2468;
t2519 = -t2498;
t2520 = -t2499;
t2522 = -t2501;
t2523 = -t2504;
t2524 = t7.*t18.*t196.*6.267440429796511e-7;
t2525 = t17.*t2466;
t2526 = t3.*t4.*t7.*t8.*t194.*7.452372645815517e-7;
t2530 = t7.*t23.*t196.*6.267440429796511e-7;
t2531 = t22.*t2466;
t2532 = t3.*t4.*t7.*t8.*t195.*7.452372645815517e-7;
t2539 = t5.*t2504;
t2541 = t91.*t197.*9.007199254740992e+15;
t2548 = -t2538;
t2550 = t197.*(t29-t30).*(-9.007199254740992e+15);
t2556 = t9.*t2538;
t2563 = -t2551;
t2564 = -t2554;
t2566 = -t2557;
t2567 = -t2558;
t2568 = -t2559;
t2569 = -t2560;
t2570 = -t2561;
t2571 = t8.*t2553;
t2580 = t2.*t196.*5.463144604697158e-2;
t2581 = t6.*t196.*5.463144604697158e-2;
t2582 = t6.*t197.*5.463144604697158e-2;
t2585 = t2.*t196.*1.324388487819695e-2;
t2586 = t2.*t197.*1.324388487819695e-2;
t2587 = t6.*t196.*1.324388487819695e-2;
t2588 = -t2572;
t2589 = -t2573;
t2598 = -t2583;
t2599 = -t2584;
t2600 = t196.*8.76226105503051e-2;
t2601 = t197.*8.76226105503051e-2;
t2606 = -t2591;
t2607 = -t2592;
t2608 = -t2593;
t2612 = t8.*t2577;
t2616 = -t2596;
t2618 = t8.*t2583;
t2619 = t8.*t2584;
t2633 = t5.*t2590;
t2634 = t9.*t2590;
t2635 = t5.*t2591;
t2636 = t5.*t2592;
t2637 = t9.*t2591;
t2638 = t9.*t2592;
t2639 = -t2605;
t2640 = -t2609;
t2641 = -t2610;
t2653 = t9.*t2596;
t2654 = t9.*t197.*4.081996247155408e-7;
t2659 = t2.*t5.*t196.*(-1.324388487819695e-2);
t2666 = -t2627;
t2667 = t5.*t2602;
t2668 = t9.*t2602;
t2669 = t5.*t2604;
t2671 = t9.*t2604;
t2672 = t5.*t2605;
t2674 = t9.*t2605;
t2677 = t2.*t5.*t196.*(-5.463144604697158e-2);
t2678 = t5.*t2595;
t2680 = t2.*t9.*t196.*(-5.463144604697158e-2);
t2681 = t5.*t6.*t196.*(-5.463144604697158e-2);
t2682 = t9.*t2595;
t2683 = t5.*t2596;
t2684 = -t2652;
t2686 = t8.*t2617;
t2688 = t9.*t194.*2.094020497221851e-7;
t2692 = t2.*t9.*t196.*1.73166333864202e-6;
t2693 = t2.*t9.*t196.*3.46332667728404e-6;
t2694 = t2.*t5.*t197.*1.73166333864202e-6;
t2695 = t2.*t5.*t197.*3.46332667728404e-6;
t2699 = t5.*t196.*(-8.76226105503051e-2);
t2702 = t6.*t9.*t197.*1.73166333864202e-6;
t2703 = t6.*t9.*t197.*3.46332667728404e-6;
t2717 = t8.*t2652;
t2720 = t2.*t9.*t197.*7.143166308571814e-6;
t2721 = t2.*t9.*t197.*1.428633261714363e-5;
t2722 = t6.*t9.*t196.*7.143166308571814e-6;
t2723 = t6.*t9.*t196.*1.428633261714363e-5;
t2724 = t5.*t6.*t197.*7.143166308571814e-6;
t2725 = t5.*t6.*t197.*1.428633261714363e-5;
t2726 = -t2687;
t2733 = t196.*5.714114815534374e-10;
t2734 = t5.*t197.*2.218657717048192e-7;
t2739 = t5.*t194.*1.138147723446811e-7;
t2741 = t9.*t196.*5.914772156006612e-6;
t2742 = t9.*t196.*1.182954431201322e-5;
t2743 = t5.*t197.*5.914772156006612e-6;
t2744 = t5.*t197.*1.182954431201322e-5;
t2748 = -t2716;
t2759 = t2.*t9.*t197.*9.41198373782161e-7;
t2760 = t2.*t9.*t197.*1.882396747564322e-6;
t2761 = t5.*t6.*t197.*9.41198373782161e-7;
t2762 = t5.*t6.*t197.*1.882396747564322e-6;
t2768 = t2.*t196.*9.136722376882659e-9;
t2769 = t2.*t197.*4.848080468348049e-9;
t2770 = t6.*t196.*4.848080468348049e-9;
t2771 = t6.*t197.*9.136722376882659e-9;
t2773 = t5.*t197.*6.433028743309294e-4;
t2774 = t7.*t9.*t194.*6.589841321991422e-6;
t2775 = t9.*t197.*6.433028743309294e-4;
t2776 = t7.*t9.*t195.*6.589841321991422e-6;
t2781 = t2.*t5.*t196.*9.41198373782161e-7;
t2782 = t2.*t5.*t196.*1.882396747564322e-6;
t2783 = -t2751;
t2784 = t24.*t194.*1.57248917878546e-6;
t2786 = t2.*t5.*t197.*3.882473205534071e-6;
t2787 = t2.*t5.*t197.*7.764946411068142e-6;
t2788 = t5.*t6.*t196.*3.882473205534071e-6;
t2789 = t5.*t6.*t196.*7.764946411068142e-6;
t2791 = t6.*t9.*t197.*3.882473205534071e-6;
t2792 = t6.*t9.*t197.*7.764946411068142e-6;
t2806 = t7.*t196.*1.486935727452378e-9;
t2808 = t5.*t196.*6.429626140715183e-6;
t2815 = t9.*t197.*6.429626140715183e-6;
t2820 = t5.*t9.*t194.*2.067207872893371e-6;
t2821 = t19.*t194.*1.57248917878546e-6;
t2829 = t5.*t7.*t195.*3.581728501918121e-6;
t2830 = t194.*t900;
t2831 = t6.*t197.*1.999848601628674e-8;
t2840 = t3.*t5.*t8.*t194.*6.589841321991422e-6;
t2842 = t3.*t5.*t8.*t195.*6.589841321991422e-6;
t2844 = -t2804;
t2845 = t194.*t882;
t2847 = t5.*t196.*3.214813070357591e-6;
t2848 = t2.*t197.*3.768927019296007e-8;
t2849 = t6.*t196.*3.768927019296007e-8;
t2853 = t197.*5.180461824884207e-7;
t2855 = t194.*t885;
t2856 = t194.*t891;
t2861 = t9.*t197.*3.214813070357591e-6;
t2862 = t2.*t196.*1.999848601628674e-8;
t2863 = t194.*t895;
t2864 = t194.*t897;
t2866 = t5.*t7.*t194.*3.581728501918121e-6;
t2868 = t196.*3.120793164930537e-8;
t2869 = t4.*t5.*t8.*t194.*(-7.660427522186475e-7);
t2879 = t2.*t196.*4.395308215012666e-6;
t2884 = t6.*t197.*4.395308215012666e-6;
t2888 = t194.*t956;
t2892 = t3.*t4.*t194.*(-7.725649335384969e-9);
t2898 = t3.*t5.*t7.*t194.*2.022455050551758e-6;
t2899 = t196.*1.169554785545351e-5;
t2900 = t3.*t4.*t5.*t194.*(-3.522139685937468e-7);
t2901 = t2.*t197.*1.813078608102233e-5;
t2902 = t6.*t196.*1.813078608102233e-5;
t2903 = t7.*t8.*t194.*(-7.725649335384969e-9);
t2908 = t3.*t8.*t9.*t194.*(-3.522139685937468e-7);
t2920 = t194.*t988;
t2923 = t194.*t993;
t2924 = t194.*t994;
t2925 = t194.*t995;
t2926 = t9.*t17.*t194.*1.011227525275879e-6;
t2927 = t194.*t999;
t2928 = t194.*t1003;
t2929 = t194.*t1013;
t2930 = t194.*t1015;
t2935 = t194.*t1026;
t2936 = t194.*t961;
t2937 = t194.*t962;
t2938 = t194.*t964;
t2940 = t194.*t966;
t2943 = t7.*t194.*2.783427048984746e-6;
t2945 = t194.*t969;
t2948 = t3.*t8.*t9.*t194.*3.581728501918121e-6;
t2949 = t7.*t195.*2.783427048984746e-6;
t2950 = t3.*t8.*t9.*t195.*3.581728501918121e-6;
t2951 = t194.*t977;
t2952 = t194.*t979;
t2960 = t3.*t7.*t19.*t194.*4.134415745786742e-6;
t2961 = t5.*t9.*t17.*t194.*4.134415745786742e-6;
t2962 = t17.*t19.*t194.*3.144978357570919e-6;
t2963 = t3.*t5.*t7.*t9.*t194.*6.289956715141839e-6;
t2964 = t17.*t24.*t194.*3.144978357570919e-6;
t2966 = t5.*t7.*t18.*t194.*(-7.044279371874937e-7);
t2967 = t3.*t8.*t19.*t194.*(-1.095406603137407e-6);
t2968 = t4.*t7.*t19.*t194.*(-1.095406603137407e-6);
t2969 = t5.*t7.*t23.*t194.*(-7.044279371874937e-7);
t2970 = t194.*t1059;
t2971 = t17.*t194.*2.134541031861069e-9;
t2975 = t3.*t4.*t19.*t194.*(-7.200154966325453e-7);
t2976 = t22.*t194.*2.134541031861069e-9;
t2979 = t194.*t1066;
t2980 = t194.*t1068;
t2981 = t194.*t1070;
t2982 = t3.*t8.*t194.*5.200343311959535e-6;
t2983 = t194.*t1078;
t2984 = t194.*t1080;
t2985 = t4.*t8.*t19.*t194.*(-7.829937223708732e-7);
t2986 = t3.*t8.*t195.*5.200343311959535e-6;
t2988 = t3.*t4.*t5.*t8.*t194.*(-7.044279371874937e-7);
t2989 = t18.*t19.*t194.*(-5.956097457010092e-7);
t2990 = t194.*t1028;
t2991 = t4.*t5.*t8.*t9.*t194.*(-1.191219491402018e-6);
t2992 = t3.*t4.*t5.*t9.*t194.*(-2.190813206274814e-6);
t2993 = -t2939;
t2996 = t3.*t5.*t8.*t9.*t194.*(-7.200154966325453e-7);
t3003 = t3.*t7.*t8.*t194.*2.218080472436232e-8;
t3004 = t3.*t7.*t9.*t194.*1.099250276973348e-6;
t3006 = t194.*t1125;
t3007 = t194.*t1126;
t3010 = t194.*t1129;
t3011 = t194.*t1130;
t3012 = t194.*t1131;
t3013 = t8.*t9.*t22.*t194.*1.011227525275879e-6;
t3014 = t4.*t8.*t9.*t194.*(-4.163616429052617e-7);
t3016 = t194.*t1139;
t3017 = t194.*t1141;
t3019 = t3.*t4.*t9.*t194.*(-1.914362954197335e-7);
t3020 = t3.*t5.*t8.*t194.*(-1.914362954197335e-7);
t3021 = t4.*t5.*t7.*t194.*(-1.914362954197335e-7);
t3023 = t4.*t17.*t194.*2.218080472436232e-8;
t3024 = t5.*t17.*t194.*5.496251384866741e-7;
t3025 = t4.*t22.*t194.*2.218080472436232e-8;
t3026 = t194.*t1169;
t3027 = t3.*t4.*t7.*t9.*t194.*1.011227525275879e-6;
t3028 = t3.*t5.*t7.*t8.*t194.*1.011227525275879e-6;
t3029 = t5.*t18.*t194.*(-2.081808214526309e-7);
t3030 = t194.*t1098;
t3031 = t194.*t1100;
t3032 = t194.*t1102;
t3033 = t194.*t1105;
t3034 = t194.*t1109;
t3035 = t194.*t1111;
t3036 = t194.*t1116;
t3038 = t4.*t5.*t8.*t17.*t194.*2.022455050551758e-6;
t3039 = t3.*t7.*t8.*t19.*t194.*2.067207872893371e-6;
t3043 = t3.*t7.*t8.*t24.*t194.*2.067207872893371e-6;
t3045 = t8.*t19.*t22.*t194.*3.144978357570919e-6;
t3046 = t197.*3.87668616986977e-7;
t3047 = t197.*3.876686384902802e-7;
t3051 = t5.*t7.*t9.*t18.*t194.*(-1.095406603137407e-6);
t3052 = t8.*t9.*t17.*t194.*(-1.011227525275879e-6);
t3053 = t5.*t7.*t9.*t23.*t194.*(-1.095406603137407e-6);
t3055 = t194.*t1204;
t3056 = t3.*t4.*t8.*t9.*t194.*(-3.828725908394669e-7);
t3057 = t4.*t5.*t7.*t8.*t194.*(-3.828725908394669e-7);
t3060 = t194.*t1214;
t3061 = t194.*t1216;
t3062 = t3.*t4.*t7.*t19.*t194.*3.144978357570919e-6;
t3063 = t2.*t5.*t197.*3.634948345122482e-13;
t3065 = t2.*t9.*t197.*3.634948345122482e-13;
t3066 = t3.*t4.*t5.*t8.*t9.*t194.*(-1.095406603137407e-6);
t3069 = t7.*t18.*t19.*t194.*(-7.200154966325453e-7);
t3070 = t7.*t19.*t23.*t194.*(-7.200154966325453e-7);
t3071 = t7.*t9.*t18.*t194.*(-3.828725908394669e-7);
t3072 = t3.*t8.*t194.*(-5.465942862546103e-7);
t3073 = t7.*t9.*t23.*t194.*(-3.828725908394669e-7);
t3075 = t5.*t197.*1.241574547458694e-12;
t3077 = t5.*t8.*t9.*t17.*t194.*(-2.067207872893371e-6);
t3078 = t3.*t7.*t8.*t9.*t194.*5.496251384866741e-7;
t3079 = t3.*t5.*t7.*t8.*t9.*t194.*(-6.289956715141839e-6);
t3080 = t9.*t197.*1.241574547458694e-12;
t3082 = t3.*t4.*t5.*t194.*(-1.38217261569615e-13);
t3083 = -t3058;
t3085 = t3.*t4.*t5.*t7.*t9.*t194.*(-2.067207872893371e-6);
t3087 = t5.*t8.*t22.*t194.*5.496251384866741e-7;
t3090 = t194.*t1272;
t3091 = t3.*t194.*6.334299027523179e-7;
t3092 = t3.*t195.*6.334299027523179e-7;
t3093 = t5.*t6.*t197.*1.499427745155113e-12;
t3094 = t3.*t4.*t5.*t7.*t194.*5.496251384866741e-7;
t3095 = t6.*t9.*t197.*1.499427745155113e-12;
t3098 = t3.*t7.*t18.*t19.*t194.*2.067207872893371e-6;
t3099 = t4.*t8.*t17.*t19.*t194.*2.067207872893371e-6;
t3103 = t194.*t1302;
t3104 = t3.*t5.*t7.*t9.*t18.*t194.*3.144978357570919e-6;
t3105 = t4.*t5.*t8.*t9.*t17.*t194.*3.144978357570919e-6;
t3108 = t194.*t1304;
t3109 = t194.*t1309;
t3111 = t194.*t1313;
t3112 = t194.*t1315;
t3113 = t4.*t8.*t194.*(-2.81948171692439e-7);
t3115 = t194.*t1278;
t3116 = t194.*t1280;
t3119 = t194.*t1284;
t3120 = t8.*t22.*t194.*1.569305128998788e-6;
C_dq = ft_7({dq1,dq2,dq3,dq4,dq5,dq6,t1004,t1006,t1008,t1009,t101,t1010,t1012,t1013,t1016,t102,t1023,t1024,t1025,t1026,t1027,t1028,t1030,t1032,t1033,t1034,t1038,t1039,t1040,t1041,t1042,t1043,t1044,t1045,t1046,t1047,t1048,t1049,t1050,t1051,t1054,t1055,t1056,t1057,t1059,t1061,t1064,t1065,t1066,t1068,t1069,t1070,t1071,t1073,t1076,t1081,t1083,t1084,t1085,t1091,t1092,t1093,t1094,t1095,t1097,t1098,t1099,t110,t1101,t1102,t1105,t1106,t1107,t1108,t1109,t111,t1113,t1115,t1116,t1119,t112,t1120,t1122,t1123,t1125,t1126,t1127,t1128,t113,t1130,t1131,t1132,t1133,t1134,t1138,t1139,t114,t1140,t1141,t1144,t1146,t1148,t115,t1150,t1151,t1152,t1153,t1155,t1158,t1159,t116,t1161,t1162,t1163,t1166,t1167,t1169,t1170,t1171,t1173,t1174,t1175,t1176,t1177,t1178,t1179,t1180,t1181,t1182,t1183,t1184,t1185,t1186,t1187,t1188,t1189,t1190,t1191,t1192,t1193,t1195,t1196,t1197,t1198,t1199,t120,t1203,t1204,t1205,t1206,t1207,t1208,t121,t1210,t1215,t1219,t1221,t1222,t1223,t1224,t1225,t1226,t1227,t1228,t1229,t1230,t1232,t1233,t1236,t124,t1240,t1242,t1244,t1245,t125,t1250,t1251,t1253,t1254,t1256,t1257,t1258,t1259,t126,t1260,t1261,t1262,t1263,t1264,t1265,t1266,t1267,t1268,t1269,t1271,t1272,t1273,t1274,t1276,t1277,t1278,t1279,t128,t1280,t1282,t1285,t1286,t1287,t1288,t129,t1290,t1293,t1294,t1295,t1296,t1297,t1298,t130,t1300,t1301,t1302,t1306,t1307,t1308,t1309,t131,t1312,t1313,t1315,t1316,t1319,t132,t1320,t1321,t1322,t1323,t1324,t1325,t1326,t1328,t1329,t133,t1330,t1331,t1332,t1333,t1334,t1335,t1337,t1338,t1339,t134,t1340,t1341,t1342,t1343,t1344,t1345,t1346,t1347,t1348,t1351,t1352,t1353,t1354,t1355,t1356,t1358,t136,t1360,t1362,t1364,t1365,t1366,t1367,t1368,t1369,t1370,t1371,t1372,t1373,t1374,t1375,t1377,t1378,t1379,t1380,t1382,t1383,t1384,t1385,t1386,t1387,t1388,t1389,t139,t1391,t1392,t1393,t1394,t1397,t1398,t140,t1401,t1402,t1403,t1404,t1405,t1406,t1407,t1408,t1409,t141,t1410,t1411,t1413,t1414,t1415,t1416,t1417,t1418,t1419,t142,t1421,t1422,t1423,t1424,t1426,t1427,t1428,t1429,t143,t1430,t1431,t1432,t1433,t1434,t1436,t1439,t144,t1440,t1442,t1443,t1444,t1445,t1447,t1448,t1449,t145,t1451,t1452,t1453,t1454,t1455,t1456,t1457,t1458,t1459,t1460,t1461,t1463,t1464,t1467,t1468,t1469,t147,t1470,t1471,t1472,t1473,t1474,t1475,t1476,t1478,t1479,t148,t1480,t1481,t1482,t1483,t1485,t1486,t1487,t1488,t1489,t1492,t1494,t1496,t1498,t1499,t15,t150,t1501,t1503,t1505,t1506,t1508,t151,t1511,t1513,t1515,t1517,t1520,t1521,t1522,t1523,t1524,t1527,t1529,t153,t1530,t1531,t1532,t1533,t1534,t1535,t1536,t1537,t1538,t1539,t154,t1541,t1542,t1548,t1549,t1550,t1551,t1553,t1557,t1558,t156,t1560,t1561,t1562,t1566,t1567,t1568,t157,t1570,t1571,t1572,t1574,t1575,t1578,t158,t1580,t1581,t1587,t1589,t1590,t1591,t1592,t1593,t1594,t1595,t1596,t1597,t1598,t1599,t16,t1605,t1606,t1607,t1609,t161,t1610,t1611,t1612,t1613,t1614,t1615,t1617,t1618,t1619,t1620,t1621,t1622,t1624,t1625,t1627,t163,t1630,t1631,t1632,t1633,t1635,t1636,t1637,t1638,t1639,t1641,t1642,t1643,t1644,t1645,t1646,t1649,t165,t1651,t1652,t1653,t1657,t1658,t1659,t166,t1660,t1661,t1662,t1663,t1665,t1666,t1669,t1670,t1671,t1672,t1673,t1674,t1676,t1681,t1682,t1683,t1687,t1689,t1692,t1695,t1696,t1697,t1698,t17,t170,t1702,t1703,t1704,t1705,t1706,t1709,t171,t1711,t1712,t1713,t1716,t1719,t1720,t1722,t1724,t1726,t1728,t1729,t173,t1731,t1733,t1734,t1735,t1736,t1737,t1738,t1739,t1740,t1743,t1744,t1745,t1746,t1748,t1749,t175,t1752,t1755,t1756,t1757,t1758,t1759,t1760,t1761,t1763,t1764,t1767,t1769,t177,t1770,t1771,t1772,t1773,t1774,t1775,t1776,t1779,t1780,t1782,t1783,t1784,t1785,t1786,t1787,t1788,t1789,t1791,t1792,t1793,t1795,t1797,t1798,t1799,t18,t1800,t1801,t1802,t1804,t1806,t1807,t1808,t1809,t1810,t1811,t1812,t1813,t1814,t1816,t1817,t1820,t1822,t1823,t1824,t1825,t1826,t1827,t1828,t1829,t183,t1830,t1831,t1832,t1833,t1834,t1835,t1836,t1837,t1838,t1839,t1844,t1847,t1849,t185,t1850,t1851,t1854,t1855,t1857,t1858,t1859,t186,t1862,t1864,t1865,t1866,t1867,t1871,t1872,t1873,t1877,t1879,t1880,t1881,t1882,t1884,t1887,t1889,t1892,t1893,t1896,t19,t190,t1903,t1904,t1906,t1907,t1908,t1909,t191,t1910,t1911,t1912,t1913,t1914,t1915,t1916,t1919,t1920,t1921,t1925,t1926,t193,t1930,t1935,t1936,t1937,t1938,t1939,t194,t1943,t1944,t1946,t195,t1950,t1955,t196,t1961,t1966,t1967,t1968,t1969,t197,t1970,t1971,t1973,t1976,t1977,t1978,t1979,t1980,t1981,t1984,t1988,t199,t1992,t1993,t1994,t1995,t1996,t1997,t1998,t1999,t2,t20,t200,t2000,t2001,t2002,t2003,t2004,t2005,t2006,t2008,t201,t2014,t2016,t2017,t2019,t202,t2020,t2021,t2023,t2024,t2028,t2029,t2033,t2036,t2037,t2038,t204,t2040,t2041,t2042,t2044,t2047,t205,t2051,t2052,t2053,t2054,t2055,t2056,t2057,t2058,t2059,t206,t2060,t2061,t2062,t2065,t2066,t2067,t2068,t2069,t207,t2070,t2071,t2072,t2073,t2074,t2076,t2077,t2078,t2079,t2080,t2081,t2082,t2083,t2084,t2085,t2086,t2087,t2088,t2089,t2091,t2092,t2093,t2094,t2095,t2096,t2097,t2098,t2099,t21,t2100,t2101,t2103,t2104,t2105,t2106,t2107,t2108,t2109,t2110,t2111,t2113,t2114,t2115,t2116,t2117,t2118,t2119,t2121,t2125,t2128,t2129,t2130,t2131,t2132,t2133,t2135,t2136,t2139,t2140,t2141,t2142,t2144,t2147,t2148,t2149,t215,t2150,t2151,t2154,t2155,t2156,t2157,t2158,t2159,t2162,t2163,t2166,t2167,t2168,t2169,t2170,t2171,t2172,t2174,t2175,t2176,t2177,t2178,t2179,t2180,t2182,t2184,t2185,t2186,t2187,t2189,t2190,t2191,t2192,t2194,t2195,t2196,t22,t2200,t2201,t2203,t2204,t2208,t2209,t2210,t2212,t2214,t2217,t2218,t2219,t2220,t2221,t2223,t2225,t2227,t2228,t2229,t2231,t2232,t2236,t2237,t2239,t224,t2240,t2243,t2246,t2249,t225,t2250,t2251,t2252,t2254,t2255,t2256,t2257,t2264,t2265,t2266,t2267,t2269,t227,t2270,t2271,t2272,t2273,t2274,t2276,t2277,t2278,t2279,t228,t2280,t2281,t2282,t2283,t2284,t2285,t2286,t2287,t2291,t2292,t2294,t2295,t23,t230,t2302,t2304,t2305,t2306,t2307,t2308,t2309,t231,t2310,t2311,t2312,t2314,t2316,t2317,t2318,t2321,t2322,t2323,t2324,t233,t2331,t2333,t2334,t2335,t2336,t2337,t2338,t2339,t234,t2340,t2341,t2342,t2344,t2347,t2348,t235,t2350,t2351,t2355,t2357,t2358,t2359,t236,t2361,t2362,t2363,t2364,t2365,t2366,t2368,t2369,t2370,t2371,t2372,t2373,t2374,t2375,t2376,t2377,t2378,t2379,t2381,t2382,t2384,t2385,t2387,t2388,t2389,t239,t2390,t2391,t2392,t2394,t2395,t2396,t2397,t24,t240,t2400,t2401,t2402,t2403,t2405,t2406,t2407,t2410,t2417,t2418,t2421,t2422,t2423,t2425,t2427,t2428,t2429,t243,t2430,t2431,t2434,t2435,t2437,t2438,t2439,t244,t2440,t2441,t2442,t2443,t2444,t2445,t2446,t2449,t2450,t2452,t2453,t2454,t2455,t2456,t2457,t2458,t2459,t2460,t2461,t2463,t2464,t2466,t2467,t2469,t2470,t2471,t2472,t2474,t2477,t2478,t2480,t2481,t2482,t2483,t2484,t2485,t2486,t2487,t2489,t249,t2495,t2497,t25,t2500,t2502,t2503,t2505,t2506,t2507,t2508,t2509,t2510,t2511,t2512,t2513,t2517,t2518,t2519,t2520,t2521,t2522,t2523,t2524,t2525,t2526,t2527,t2530,t2531,t2532,t2533,t2535,t2536,t2537,t2539,t2540,t2541,t2543,t2544,t2545,t2546,t2548,t2549,t2550,t2552,t2553,t2554,t2555,t2556,t2560,t2562,t2563,t2564,t2565,t2566,t2567,t2568,t2569,t257,t2570,t2571,t2574,t2575,t2576,t2577,t2578,t2579,t258,t2580,t2581,t2582,t2585,t2586,t2587,t2588,t2589,t2590,t2595,t2597,t2598,t2599,t26,t2600,t2601,t2602,t2603,t2604,t2606,t2607,t2608,t2611,t2612,t2615,t2616,t2617,t2627,t263,t2633,t2634,t2636,t2639,t2640,t2641,t2654,t2655,t2656,t2659,t266,t2666,t2668,t2669,t2671,t2673,t2675,t2676,t2677,t2678,t2680,t2681,t2682,t2684,t2685,t2686,t2688,t2692,t2693,t2694,t2695,t2699,t270,t2702,t2703,t2705,t2706,t2707,t2708,t2719,t2720,t2721,t2722,t2723,t2724,t2725,t2726,t273,t2733,t2734,t2739,t274,t2741,t2742,t2743,t2744,t2748,t2749,t275,t2752,t2759,t276,t2760,t2761,t2762,t2764,t2768,t2769,t277,t2770,t2771,t2773,t2774,t2775,t2776,t278,t2781,t2782,t2783,t2784,t2786,t2787,t2788,t2789,t2791,t2792,t280,t2806,t2808,t2815,t2820,t2821,t2829,t2830,t2831,t284,t2840,t2842,t2844,t2845,t2847,t2848,t2849,t2853,t2854,t2861,t2862,t2863,t2864,t2866,t2868,t2869,t287,t2879,t2884,t2886,t2888,t2892,t2898,t2899,t29,t290,t2900,t2901,t2902,t2903,t2908,t291,t292,t2920,t2923,t2925,t2926,t2928,t2929,t2930,t2937,t294,t2940,t2943,t2945,t2948,t2949,t2950,t2951,t2952,t2960,t2961,t2962,t2963,t2964,t2966,t2967,t2968,t2969,t297,t2970,t2971,t2975,t2976,t2980,t2982,t2983,t2984,t2985,t2986,t2988,t2989,t299,t2991,t2992,t2993,t2996,t2997,t3,t30,t300,t3003,t3004,t3007,t3010,t3011,t3013,t3014,t3019,t302,t3020,t3021,t3023,t3024,t3025,t3027,t3028,t3029,t303,t3030,t3031,t3032,t3033,t3034,t3035,t3036,t3038,t3039,t304,t3043,t3045,t3046,t3047,t305,t3051,t3052,t3053,t3055,t3056,t3057,t306,t3060,t3061,t3062,t3063,t3065,t3066,t3069,t3070,t3071,t3072,t3073,t3075,t3077,t3078,t3079,t3080,t3082,t3083,t3085,t3087,t309,t3090,t3091,t3092,t3093,t3094,t3095,t3098,t3099,t310,t3103,t3104,t3105,t3108,t3109,t311,t3112,t3113,t3119,t3120,t313,t314,t3142,t315,t3158,t316,t318,t319,t3191,t320,t3208,t3211,t3212,t3218,t3219,t322,t3225,t3228,t3230,t3231,t324,t3243,t3244,t325,t3251,t3252,t3255,t3257,t3258,t3259,t3261,t3273,t3274,t3275,t3279,t328,t3282,t3286,t3288,t3289,t3290,t3294,t3295,t3309,t3314,t3317,t3319,t3320,t3321,t3326,t3327,t3328,t3329,t333,t3330,t3331,t3333,t3334,t3335,t3343,t336,t3363,t3364,t3365,t3367,t3368,t3369,t337,t3370,t3371,t3372,t3373,t3374,t3375,t3376,t3378,t3379,t3380,t3381,t3382,t3389,t3390,t3391,t3392,t3393,t3394,t3395,t3397,t34,t340,t3400,t3401,t3402,t3403,t3409,t3416,t3417,t3418,t3419,t3420,t3426,t3430,t3432,t3434,t3435,t3437,t3438,t3439,t344,t3440,t3442,t3443,t3444,t3445,t3446,t3447,t3449,t3450,t3452,t3453,t3454,t3455,t3456,t3459,t346,t3462,t3463,t3466,t3468,t3469,t347,t3470,t3472,t3473,t3475,t3477,t3479,t348,t3481,t3483,t3486,t3489,t349,t3492,t350,t3500,t3501,t3506,t3507,t3509,t3514,t3515,t3516,t3517,t3519,t352,t3520,t3521,t3522,t3523,t3524,t353,t3530,t3532,t3533,t3534,t3535,t3538,t3539,t3541,t3544,t3546,t3548,t3549,t3553,t3556,t356,t3560,t3568,t3569,t357,t3572,t3573,t3574,t3575,t3576,t3578,t3579,t358,t3581,t3582,t3583,t3584,t3585,t359,t3590,t3596,t3597,t3601,t3602,t3604,t3607,t3609,t361,t3613,t3616,t3617,t3618,t362,t3622,t3629,t3630,t3637,t3638,t3639,t3641,t3643,t3646,t3647,t3649,t365,t3650,t3652,t3653,t3654,t3659,t3660,t3662,t3663,t3668,t3676,t368,t3680,t3682,t3686,t369,t3691,t3695,t3697,t3701,t3709,t371,t3714,t3716,t3717,t372,t3722,t3726,t3729,t373,t3730,t3736,t3737,t3738,t374,t3743,t3744,t3747,t3748,t3750,t3751,t3756,t377,t3774,t378,t3789,t379,t3798,t380,t3815,t382,t3822,t3824,t3825,t3834,t3835,t3839,t384,t3846,t3847,t3852,t386,t387,t388,t3889,t3892,t3898,t3899,t391,t3915,t392,t395,t3950,t3951,t3958,t3959,t396,t4,t400,t4001,t4002,t4004,t4007,t401,t402,t4028,t4029,t403,t4030,t4031,t4032,t4033,t4039,t4040,t4041,t4042,t4043,t4044,t4045,t4051,t4052,t4058,t406,t410,t4105,t411,t4113,t4114,t4117,t4118,t412,t4123,t413,t414,t4143,t4144,t4145,t415,t4150,t4152,t4153,t4155,t416,t4160,t4164,t4165,t417,t4170,t4174,t4177,t4178,t4179,t418,t4180,t4181,t4182,t4183,t4184,t4185,t4186,t4187,t4188,t4189,t4190,t4191,t4192,t4193,t4194,t4196,t4197,t420,t4200,t4203,t4204,t4205,t4206,t4207,t4208,t4209,t4211,t4212,t4213,t4214,t4216,t422,t4221,t4228,t4229,t423,t4230,t4231,t4232,t4233,t4235,t4236,t4237,t4239,t424,t4240,t4242,t4243,t4246,t4249,t425,t4255,t4256,t4257,t4258,t4259,t4260,t4261,t4262,t4265,t4266,t4268,t427,t4271,t4272,t4275,t4277,t4278,t4279,t428,t4283,t4284,t4287,t4288,t4289,t429,t4290,t4292,t4293,t4294,t4295,t4296,t4297,t4298,t4299,t4300,t4301,t4304,t4308,t4309,t431,t4310,t4311,t4313,t4315,t4316,t4317,t4319,t432,t4320,t4321,t4323,t4325,t4326,t4328,t433,t4330,t4333,t4334,t4335,t4336,t4337,t4338,t4339,t434,t4341,t4342,t4343,t4344,t4345,t4346,t4347,t435,t4351,t4353,t4355,t436,t4361,t4365,t4367,t4369,t437,t4370,t4371,t4372,t4375,t4377,t4379,t438,t4382,t4385,t4387,t439,t4390,t4391,t4392,t4394,t4395,t4396,t4397,t44,t440,t4401,t4402,t4403,t4404,t4405,t4406,t4407,t4408,t441,t4410,t4411,t4412,t4413,t4417,t4419,t442,t4420,t4421,t4422,t4425,t4426,t4428,t4429,t4431,t4432,t4435,t4436,t444,t4440,t4442,t4443,t4444,t4445,t4446,t4448,t4449,t445,t4450,t4452,t4453,t4455,t4457,t4459,t4462,t4464,t4469,t4473,t4478,t4479,t448,t4480,t4481,t4483,t4484,t4485,t4486,t4488,t449,t4491,t4492,t4493,t4495,t4498,t45,t450,t4501,t4502,t4504,t4506,t4508,t4509,t4513,t4516,t4517,t4519,t452,t4520,t4522,t4524,t4525,t453,t4530,t4532,t4533,t454,t4540,t4542,t4543,t4547,t4548,t4549,t4551,t4554,t4555,t4557,t4558,t4559,t4561,t4562,t4563,t4566,t4567,t4568,t4569,t457,t4570,t4571,t4572,t4574,t4575,t4577,t4579,t458,t4581,t4582,t4583,t4584,t4588,t4589,t459,t4590,t4591,t4595,t4596,t46,t460,t4600,t4601,t4605,t4606,t4607,t461,t4611,t4614,t4616,t4617,t462,t4621,t4622,t4625,t4626,t4628,t4629,t463,t4630,t4632,t4633,t4634,t4636,t4637,t4638,t4639,t464,t4640,t4641,t4642,t4643,t4644,t4645,t4646,t4647,t4649,t465,t4650,t4651,t4652,t4653,t4656,t4657,t4658,t466,t4660,t4661,t4662,t4663,t4666,t4667,t4669,t4672,t4673,t4674,t4675,t468,t4688,t469,t4691,t4692,t4693,t4694,t4695,t4696,t4697,t47,t470,t4707,t4708,t4709,t471,t4711,t4713,t4716,t472,t4722,t4723,t4724,t4725,t4726,t4727,t4728,t4731,t4732,t4733,t4734,t4737,t4740,t4741,t4742,t4745,t4747,t4748,t4749,t475,t4752,t4753,t4754,t4755,t4756,t4758,t4759,t4760,t4761,t4763,t4766,t4769,t477,t4770,t4777,t4778,t4782,t4783,t4785,t4786,t4788,t4789,t479,t4790,t4794,t4795,t4796,t4797,t4798,t4799,t480,t4800,t4801,t4803,t4804,t4805,t4807,t4808,t481,t4811,t4813,t4814,t4815,t4818,t482,t4820,t4824,t4825,t4827,t4828,t483,t4830,t4832,t4833,t4834,t4835,t4837,t4839,t484,t4841,t4842,t4845,t4846,t4849,t485,t4852,t486,t4861,t4862,t4864,t4865,t4866,t4867,t4871,t4872,t4873,t4876,t4877,t4878,t4879,t488,t4882,t4883,t4884,t4886,t4887,t489,t4895,t4897,t4899,t4900,t4908,t4909,t491,t4910,t4911,t4913,t4915,t4916,t4919,t492,t4920,t4923,t4924,t4925,t4927,t4928,t493,t4930,t4933,t4934,t4937,t4938,t494,t4941,t4942,t4943,t4944,t4945,t4946,t4948,t4951,t4955,t4956,t4957,t496,t4962,t4964,t4969,t497,t4970,t4973,t4974,t4976,t498,t4980,t4981,t4982,t4983,t4986,t4987,t4988,t499,t4991,t4993,t4996,t4998,t4999,t5,t50,t500,t5000,t5001,t5004,t5006,t5008,t501,t5019,t502,t5021,t5022,t5023,t5026,t5027,t5029,t503,t5034,t5035,t5036,t5038,t504,t5045,t5046,t505,t5051,t5052,t5053,t506,t5060,t5062,t5063,t5064,t5065,t5066,t5069,t507,t5071,t5072,t5073,t5078,t508,t5080,t5082,t5083,t5084,t5085,t509,t5091,t5093,t5095,t5096,t5097,t5098,t5099,t510,t5100,t5102,t5107,t511,t5111,t5112,t5113,t5114,t5116,t5119,t512,t5120,t5122,t5127,t513,t5130,t5139,t514,t5142,t5147,t5149,t5150,t5151,t5154,t5158,t516,t5165,t517,t5171,t5172,t5176,t5179,t518,t5180,t5181,t5183,t5184,t5185,t5186,t5187,t5192,t5193,t5199,t520,t5200,t5203,t5204,t5205,t5208,t521,t5215,t5216,t5217,t522,t5222,t5223,t5224,t5227,t523,t5236,t5237,t5238,t5239,t524,t5240,t5244,t5245,t525,t5250,t5252,t5258,t526,t5267,t527,t5270,t5271,t5279,t528,t5280,t5281,t5285,t529,t5293,t5294,t53,t530,t5305,t531,t5318,t5319,t532,t5321,t5324,t5325,t5327,t5328,t533,t5331,t5332,t534,t535,t5353,t5355,t5356,t5358,t536,t5361,t5362,t5364,t5368,t537,t5372,t5373,t5376,t5378,t538,t5387,t5389,t539,t5390,t5391,t5392,t5393,t5394,t540,t5402,t5404,t5409,t5416,t5420,t5424,t5429,t543,t5430,t5434,t5435,t5436,t5439,t544,t5440,t5441,t5445,t5449,t545,t5450,t5451,t5452,t5453,t5455,t5456,t5457,t546,t5467,t5468,t5469,t547,t5470,t5471,t5472,t5473,t5474,t5475,t5476,t5477,t5478,t548,t5489,t549,t5490,t5493,t5494,t5497,t5499,t5501,t5508,t551,t5510,t5512,t5516,t5517,t552,t5521,t553,t5532,t5535,t554,t5540,t5547,t555,t5557,t5558,t556,t557,t5574,t5578,t5579,t558,t5582,t5586,t559,t5590,t5593,t5596,t560,t5604,t5607,t561,t5612,t562,t5629,t563,t5634,t5635,t564,t567,t568,t5688,t569,t57,t570,t571,t572,t573,t574,t5741,t5743,t576,t577,t5777,t5779,t578,t5780,t5782,t579,t58,t580,t581,t582,t5826,t583,t584,t586,t587,t5886,t5887,t589,t5894,t59,t590,t591,t592,t593,t594,t595,t596,t597,t6,t60,t600,t602,t603,t604,t605,t609,t610,t611,t612,t613,t614,t615,t616,t618,t619,t622,t623,t624,t625,t626,t627,t628,t629,t63,t630,t631,t633,t634,t635,t636,t637,t638,t639,t640,t641,t642,t643,t648,t649,t650,t653,t654,t655,t656,t657,t658,t660,t662,t663,t664,t665,t667,t668,t673,t674,t675,t676,t678,t679,t681,t682,t683,t684,t685,t686,t687,t688,t689,t693,t694,t695,t696,t697,t698,t7,t700,t702,t703,t704,t705,t706,t71,t710,t711,t712,t713,t715,t716,t72,t724,t728,t73,t731,t733,t734,t735,t736,t74,t741,t742,t743,t744,t746,t747,t748,t749,t75,t750,t751,t752,t754,t755,t756,t757,t758,t759,t76,t760,t762,t763,t764,t765,t766,t767,t768,t769,t77,t772,t773,t774,t775,t776,t777,t778,t779,t780,t781,t782,t784,t785,t786,t790,t792,t794,t795,t796,t798,t8,t80,t801,t804,t805,t806,t808,t81,t814,t815,t817,t82,t820,t822,t825,t827,t83,t831,t832,t833,t834,t835,t836,t837,t838,t84,t840,t841,t842,t843,t846,t86,t863,t868,t869,t870,t874,t878,t880,t881,t882,t884,t885,t888,t889,t891,t892,t895,t899,t9,t90,t900,t903,t906,t91,t911,t921,t922,t923,t925,t926,t927,t929,t934,t935,t936,t937,t940,t941,t942,t946,t949,t95,t950,t954,t955,t957,t958,t961,t962,t964,t965,t968,t97,t970,t971,t972,t973,t975,t977,t982,t983,t984,t986,t987,t988,t989,t99,t993,t994,t995,t999});
end
function C_dq = ft_7(ct)
dq1 = ct{1};
dq2 = ct{2};
dq3 = ct{3};
dq4 = ct{4};
dq5 = ct{5};
dq6 = ct{6};
t1004 = ct{7};
t1006 = ct{8};
t1008 = ct{9};
t1009 = ct{10};
t101 = ct{11};
t1010 = ct{12};
t1012 = ct{13};
t1013 = ct{14};
t1016 = ct{15};
t102 = ct{16};
t1023 = ct{17};
t1024 = ct{18};
t1025 = ct{19};
t1026 = ct{20};
t1027 = ct{21};
t1028 = ct{22};
t1030 = ct{23};
t1032 = ct{24};
t1033 = ct{25};
t1034 = ct{26};
t1038 = ct{27};
t1039 = ct{28};
t1040 = ct{29};
t1041 = ct{30};
t1042 = ct{31};
t1043 = ct{32};
t1044 = ct{33};
t1045 = ct{34};
t1046 = ct{35};
t1047 = ct{36};
t1048 = ct{37};
t1049 = ct{38};
t1050 = ct{39};
t1051 = ct{40};
t1054 = ct{41};
t1055 = ct{42};
t1056 = ct{43};
t1057 = ct{44};
t1059 = ct{45};
t1061 = ct{46};
t1064 = ct{47};
t1065 = ct{48};
t1066 = ct{49};
t1068 = ct{50};
t1069 = ct{51};
t1070 = ct{52};
t1071 = ct{53};
t1073 = ct{54};
t1076 = ct{55};
t1081 = ct{56};
t1083 = ct{57};
t1084 = ct{58};
t1085 = ct{59};
t1091 = ct{60};
t1092 = ct{61};
t1093 = ct{62};
t1094 = ct{63};
t1095 = ct{64};
t1097 = ct{65};
t1098 = ct{66};
t1099 = ct{67};
t110 = ct{68};
t1101 = ct{69};
t1102 = ct{70};
t1105 = ct{71};
t1106 = ct{72};
t1107 = ct{73};
t1108 = ct{74};
t1109 = ct{75};
t111 = ct{76};
t1113 = ct{77};
t1115 = ct{78};
t1116 = ct{79};
t1119 = ct{80};
t112 = ct{81};
t1120 = ct{82};
t1122 = ct{83};
t1123 = ct{84};
t1125 = ct{85};
t1126 = ct{86};
t1127 = ct{87};
t1128 = ct{88};
t113 = ct{89};
t1130 = ct{90};
t1131 = ct{91};
t1132 = ct{92};
t1133 = ct{93};
t1134 = ct{94};
t1138 = ct{95};
t1139 = ct{96};
t114 = ct{97};
t1140 = ct{98};
t1141 = ct{99};
t1144 = ct{100};
t1146 = ct{101};
t1148 = ct{102};
t115 = ct{103};
t1150 = ct{104};
t1151 = ct{105};
t1152 = ct{106};
t1153 = ct{107};
t1155 = ct{108};
t1158 = ct{109};
t1159 = ct{110};
t116 = ct{111};
t1161 = ct{112};
t1162 = ct{113};
t1163 = ct{114};
t1166 = ct{115};
t1167 = ct{116};
t1169 = ct{117};
t1170 = ct{118};
t1171 = ct{119};
t1173 = ct{120};
t1174 = ct{121};
t1175 = ct{122};
t1176 = ct{123};
t1177 = ct{124};
t1178 = ct{125};
t1179 = ct{126};
t1180 = ct{127};
t1181 = ct{128};
t1182 = ct{129};
t1183 = ct{130};
t1184 = ct{131};
t1185 = ct{132};
t1186 = ct{133};
t1187 = ct{134};
t1188 = ct{135};
t1189 = ct{136};
t1190 = ct{137};
t1191 = ct{138};
t1192 = ct{139};
t1193 = ct{140};
t1195 = ct{141};
t1196 = ct{142};
t1197 = ct{143};
t1198 = ct{144};
t1199 = ct{145};
t120 = ct{146};
t1203 = ct{147};
t1204 = ct{148};
t1205 = ct{149};
t1206 = ct{150};
t1207 = ct{151};
t1208 = ct{152};
t121 = ct{153};
t1210 = ct{154};
t1215 = ct{155};
t1219 = ct{156};
t1221 = ct{157};
t1222 = ct{158};
t1223 = ct{159};
t1224 = ct{160};
t1225 = ct{161};
t1226 = ct{162};
t1227 = ct{163};
t1228 = ct{164};
t1229 = ct{165};
t1230 = ct{166};
t1232 = ct{167};
t1233 = ct{168};
t1236 = ct{169};
t124 = ct{170};
t1240 = ct{171};
t1242 = ct{172};
t1244 = ct{173};
t1245 = ct{174};
t125 = ct{175};
t1250 = ct{176};
t1251 = ct{177};
t1253 = ct{178};
t1254 = ct{179};
t1256 = ct{180};
t1257 = ct{181};
t1258 = ct{182};
t1259 = ct{183};
t126 = ct{184};
t1260 = ct{185};
t1261 = ct{186};
t1262 = ct{187};
t1263 = ct{188};
t1264 = ct{189};
t1265 = ct{190};
t1266 = ct{191};
t1267 = ct{192};
t1268 = ct{193};
t1269 = ct{194};
t1271 = ct{195};
t1272 = ct{196};
t1273 = ct{197};
t1274 = ct{198};
t1276 = ct{199};
t1277 = ct{200};
t1278 = ct{201};
t1279 = ct{202};
t128 = ct{203};
t1280 = ct{204};
t1282 = ct{205};
t1285 = ct{206};
t1286 = ct{207};
t1287 = ct{208};
t1288 = ct{209};
t129 = ct{210};
t1290 = ct{211};
t1293 = ct{212};
t1294 = ct{213};
t1295 = ct{214};
t1296 = ct{215};
t1297 = ct{216};
t1298 = ct{217};
t130 = ct{218};
t1300 = ct{219};
t1301 = ct{220};
t1302 = ct{221};
t1306 = ct{222};
t1307 = ct{223};
t1308 = ct{224};
t1309 = ct{225};
t131 = ct{226};
t1312 = ct{227};
t1313 = ct{228};
t1315 = ct{229};
t1316 = ct{230};
t1319 = ct{231};
t132 = ct{232};
t1320 = ct{233};
t1321 = ct{234};
t1322 = ct{235};
t1323 = ct{236};
t1324 = ct{237};
t1325 = ct{238};
t1326 = ct{239};
t1328 = ct{240};
t1329 = ct{241};
t133 = ct{242};
t1330 = ct{243};
t1331 = ct{244};
t1332 = ct{245};
t1333 = ct{246};
t1334 = ct{247};
t1335 = ct{248};
t1337 = ct{249};
t1338 = ct{250};
t1339 = ct{251};
t134 = ct{252};
t1340 = ct{253};
t1341 = ct{254};
t1342 = ct{255};
t1343 = ct{256};
t1344 = ct{257};
t1345 = ct{258};
t1346 = ct{259};
t1347 = ct{260};
t1348 = ct{261};
t1351 = ct{262};
t1352 = ct{263};
t1353 = ct{264};
t1354 = ct{265};
t1355 = ct{266};
t1356 = ct{267};
t1358 = ct{268};
t136 = ct{269};
t1360 = ct{270};
t1362 = ct{271};
t1364 = ct{272};
t1365 = ct{273};
t1366 = ct{274};
t1367 = ct{275};
t1368 = ct{276};
t1369 = ct{277};
t1370 = ct{278};
t1371 = ct{279};
t1372 = ct{280};
t1373 = ct{281};
t1374 = ct{282};
t1375 = ct{283};
t1377 = ct{284};
t1378 = ct{285};
t1379 = ct{286};
t1380 = ct{287};
t1382 = ct{288};
t1383 = ct{289};
t1384 = ct{290};
t1385 = ct{291};
t1386 = ct{292};
t1387 = ct{293};
t1388 = ct{294};
t1389 = ct{295};
t139 = ct{296};
t1391 = ct{297};
t1392 = ct{298};
t1393 = ct{299};
t1394 = ct{300};
t1397 = ct{301};
t1398 = ct{302};
t140 = ct{303};
t1401 = ct{304};
t1402 = ct{305};
t1403 = ct{306};
t1404 = ct{307};
t1405 = ct{308};
t1406 = ct{309};
t1407 = ct{310};
t1408 = ct{311};
t1409 = ct{312};
t141 = ct{313};
t1410 = ct{314};
t1411 = ct{315};
t1413 = ct{316};
t1414 = ct{317};
t1415 = ct{318};
t1416 = ct{319};
t1417 = ct{320};
t1418 = ct{321};
t1419 = ct{322};
t142 = ct{323};
t1421 = ct{324};
t1422 = ct{325};
t1423 = ct{326};
t1424 = ct{327};
t1426 = ct{328};
t1427 = ct{329};
t1428 = ct{330};
t1429 = ct{331};
t143 = ct{332};
t1430 = ct{333};
t1431 = ct{334};
t1432 = ct{335};
t1433 = ct{336};
t1434 = ct{337};
t1436 = ct{338};
t1439 = ct{339};
t144 = ct{340};
t1440 = ct{341};
t1442 = ct{342};
t1443 = ct{343};
t1444 = ct{344};
t1445 = ct{345};
t1447 = ct{346};
t1448 = ct{347};
t1449 = ct{348};
t145 = ct{349};
t1451 = ct{350};
t1452 = ct{351};
t1453 = ct{352};
t1454 = ct{353};
t1455 = ct{354};
t1456 = ct{355};
t1457 = ct{356};
t1458 = ct{357};
t1459 = ct{358};
t1460 = ct{359};
t1461 = ct{360};
t1463 = ct{361};
t1464 = ct{362};
t1467 = ct{363};
t1468 = ct{364};
t1469 = ct{365};
t147 = ct{366};
t1470 = ct{367};
t1471 = ct{368};
t1472 = ct{369};
t1473 = ct{370};
t1474 = ct{371};
t1475 = ct{372};
t1476 = ct{373};
t1478 = ct{374};
t1479 = ct{375};
t148 = ct{376};
t1480 = ct{377};
t1481 = ct{378};
t1482 = ct{379};
t1483 = ct{380};
t1485 = ct{381};
t1486 = ct{382};
t1487 = ct{383};
t1488 = ct{384};
t1489 = ct{385};
t1492 = ct{386};
t1494 = ct{387};
t1496 = ct{388};
t1498 = ct{389};
t1499 = ct{390};
t15 = ct{391};
t150 = ct{392};
t1501 = ct{393};
t1503 = ct{394};
t1505 = ct{395};
t1506 = ct{396};
t1508 = ct{397};
t151 = ct{398};
t1511 = ct{399};
t1513 = ct{400};
t1515 = ct{401};
t1517 = ct{402};
t1520 = ct{403};
t1521 = ct{404};
t1522 = ct{405};
t1523 = ct{406};
t1524 = ct{407};
t1527 = ct{408};
t1529 = ct{409};
t153 = ct{410};
t1530 = ct{411};
t1531 = ct{412};
t1532 = ct{413};
t1533 = ct{414};
t1534 = ct{415};
t1535 = ct{416};
t1536 = ct{417};
t1537 = ct{418};
t1538 = ct{419};
t1539 = ct{420};
t154 = ct{421};
t1541 = ct{422};
t1542 = ct{423};
t1548 = ct{424};
t1549 = ct{425};
t1550 = ct{426};
t1551 = ct{427};
t1553 = ct{428};
t1557 = ct{429};
t1558 = ct{430};
t156 = ct{431};
t1560 = ct{432};
t1561 = ct{433};
t1562 = ct{434};
t1566 = ct{435};
t1567 = ct{436};
t1568 = ct{437};
t157 = ct{438};
t1570 = ct{439};
t1571 = ct{440};
t1572 = ct{441};
t1574 = ct{442};
t1575 = ct{443};
t1578 = ct{444};
t158 = ct{445};
t1580 = ct{446};
t1581 = ct{447};
t1587 = ct{448};
t1589 = ct{449};
t1590 = ct{450};
t1591 = ct{451};
t1592 = ct{452};
t1593 = ct{453};
t1594 = ct{454};
t1595 = ct{455};
t1596 = ct{456};
t1597 = ct{457};
t1598 = ct{458};
t1599 = ct{459};
t16 = ct{460};
t1605 = ct{461};
t1606 = ct{462};
t1607 = ct{463};
t1609 = ct{464};
t161 = ct{465};
t1610 = ct{466};
t1611 = ct{467};
t1612 = ct{468};
t1613 = ct{469};
t1614 = ct{470};
t1615 = ct{471};
t1617 = ct{472};
t1618 = ct{473};
t1619 = ct{474};
t1620 = ct{475};
t1621 = ct{476};
t1622 = ct{477};
t1624 = ct{478};
t1625 = ct{479};
t1627 = ct{480};
t163 = ct{481};
t1630 = ct{482};
t1631 = ct{483};
t1632 = ct{484};
t1633 = ct{485};
t1635 = ct{486};
t1636 = ct{487};
t1637 = ct{488};
t1638 = ct{489};
t1639 = ct{490};
t1641 = ct{491};
t1642 = ct{492};
t1643 = ct{493};
t1644 = ct{494};
t1645 = ct{495};
t1646 = ct{496};
t1649 = ct{497};
t165 = ct{498};
t1651 = ct{499};
t1652 = ct{500};
t1653 = ct{501};
t1657 = ct{502};
t1658 = ct{503};
t1659 = ct{504};
t166 = ct{505};
t1660 = ct{506};
t1661 = ct{507};
t1662 = ct{508};
t1663 = ct{509};
t1665 = ct{510};
t1666 = ct{511};
t1669 = ct{512};
t1670 = ct{513};
t1671 = ct{514};
t1672 = ct{515};
t1673 = ct{516};
t1674 = ct{517};
t1676 = ct{518};
t1681 = ct{519};
t1682 = ct{520};
t1683 = ct{521};
t1687 = ct{522};
t1689 = ct{523};
t1692 = ct{524};
t1695 = ct{525};
t1696 = ct{526};
t1697 = ct{527};
t1698 = ct{528};
t17 = ct{529};
t170 = ct{530};
t1702 = ct{531};
t1703 = ct{532};
t1704 = ct{533};
t1705 = ct{534};
t1706 = ct{535};
t1709 = ct{536};
t171 = ct{537};
t1711 = ct{538};
t1712 = ct{539};
t1713 = ct{540};
t1716 = ct{541};
t1719 = ct{542};
t1720 = ct{543};
t1722 = ct{544};
t1724 = ct{545};
t1726 = ct{546};
t1728 = ct{547};
t1729 = ct{548};
t173 = ct{549};
t1731 = ct{550};
t1733 = ct{551};
t1734 = ct{552};
t1735 = ct{553};
t1736 = ct{554};
t1737 = ct{555};
t1738 = ct{556};
t1739 = ct{557};
t1740 = ct{558};
t1743 = ct{559};
t1744 = ct{560};
t1745 = ct{561};
t1746 = ct{562};
t1748 = ct{563};
t1749 = ct{564};
t175 = ct{565};
t1752 = ct{566};
t1755 = ct{567};
t1756 = ct{568};
t1757 = ct{569};
t1758 = ct{570};
t1759 = ct{571};
t1760 = ct{572};
t1761 = ct{573};
t1763 = ct{574};
t1764 = ct{575};
t1767 = ct{576};
t1769 = ct{577};
t177 = ct{578};
t1770 = ct{579};
t1771 = ct{580};
t1772 = ct{581};
t1773 = ct{582};
t1774 = ct{583};
t1775 = ct{584};
t1776 = ct{585};
t1779 = ct{586};
t1780 = ct{587};
t1782 = ct{588};
t1783 = ct{589};
t1784 = ct{590};
t1785 = ct{591};
t1786 = ct{592};
t1787 = ct{593};
t1788 = ct{594};
t1789 = ct{595};
t1791 = ct{596};
t1792 = ct{597};
t1793 = ct{598};
t1795 = ct{599};
t1797 = ct{600};
t1798 = ct{601};
t1799 = ct{602};
t18 = ct{603};
t1800 = ct{604};
t1801 = ct{605};
t1802 = ct{606};
t1804 = ct{607};
t1806 = ct{608};
t1807 = ct{609};
t1808 = ct{610};
t1809 = ct{611};
t1810 = ct{612};
t1811 = ct{613};
t1812 = ct{614};
t1813 = ct{615};
t1814 = ct{616};
t1816 = ct{617};
t1817 = ct{618};
t1820 = ct{619};
t1822 = ct{620};
t1823 = ct{621};
t1824 = ct{622};
t1825 = ct{623};
t1826 = ct{624};
t1827 = ct{625};
t1828 = ct{626};
t1829 = ct{627};
t183 = ct{628};
t1830 = ct{629};
t1831 = ct{630};
t1832 = ct{631};
t1833 = ct{632};
t1834 = ct{633};
t1835 = ct{634};
t1836 = ct{635};
t1837 = ct{636};
t1838 = ct{637};
t1839 = ct{638};
t1844 = ct{639};
t1847 = ct{640};
t1849 = ct{641};
t185 = ct{642};
t1850 = ct{643};
t1851 = ct{644};
t1854 = ct{645};
t1855 = ct{646};
t1857 = ct{647};
t1858 = ct{648};
t1859 = ct{649};
t186 = ct{650};
t1862 = ct{651};
t1864 = ct{652};
t1865 = ct{653};
t1866 = ct{654};
t1867 = ct{655};
t1871 = ct{656};
t1872 = ct{657};
t1873 = ct{658};
t1877 = ct{659};
t1879 = ct{660};
t1880 = ct{661};
t1881 = ct{662};
t1882 = ct{663};
t1884 = ct{664};
t1887 = ct{665};
t1889 = ct{666};
t1892 = ct{667};
t1893 = ct{668};
t1896 = ct{669};
t19 = ct{670};
t190 = ct{671};
t1903 = ct{672};
t1904 = ct{673};
t1906 = ct{674};
t1907 = ct{675};
t1908 = ct{676};
t1909 = ct{677};
t191 = ct{678};
t1910 = ct{679};
t1911 = ct{680};
t1912 = ct{681};
t1913 = ct{682};
t1914 = ct{683};
t1915 = ct{684};
t1916 = ct{685};
t1919 = ct{686};
t1920 = ct{687};
t1921 = ct{688};
t1925 = ct{689};
t1926 = ct{690};
t193 = ct{691};
t1930 = ct{692};
t1935 = ct{693};
t1936 = ct{694};
t1937 = ct{695};
t1938 = ct{696};
t1939 = ct{697};
t194 = ct{698};
t1943 = ct{699};
t1944 = ct{700};
t1946 = ct{701};
t195 = ct{702};
t1950 = ct{703};
t1955 = ct{704};
t196 = ct{705};
t1961 = ct{706};
t1966 = ct{707};
t1967 = ct{708};
t1968 = ct{709};
t1969 = ct{710};
t197 = ct{711};
t1970 = ct{712};
t1971 = ct{713};
t1973 = ct{714};
t1976 = ct{715};
t1977 = ct{716};
t1978 = ct{717};
t1979 = ct{718};
t1980 = ct{719};
t1981 = ct{720};
t1984 = ct{721};
t1988 = ct{722};
t199 = ct{723};
t1992 = ct{724};
t1993 = ct{725};
t1994 = ct{726};
t1995 = ct{727};
t1996 = ct{728};
t1997 = ct{729};
t1998 = ct{730};
t1999 = ct{731};
t2 = ct{732};
t20 = ct{733};
t200 = ct{734};
t2000 = ct{735};
t2001 = ct{736};
t2002 = ct{737};
t2003 = ct{738};
t2004 = ct{739};
t2005 = ct{740};
t2006 = ct{741};
t2008 = ct{742};
t201 = ct{743};
t2014 = ct{744};
t2016 = ct{745};
t2017 = ct{746};
t2019 = ct{747};
t202 = ct{748};
t2020 = ct{749};
t2021 = ct{750};
t2023 = ct{751};
t2024 = ct{752};
t2028 = ct{753};
t2029 = ct{754};
t2033 = ct{755};
t2036 = ct{756};
t2037 = ct{757};
t2038 = ct{758};
t204 = ct{759};
t2040 = ct{760};
t2041 = ct{761};
t2042 = ct{762};
t2044 = ct{763};
t2047 = ct{764};
t205 = ct{765};
t2051 = ct{766};
t2052 = ct{767};
t2053 = ct{768};
t2054 = ct{769};
t2055 = ct{770};
t2056 = ct{771};
t2057 = ct{772};
t2058 = ct{773};
t2059 = ct{774};
t206 = ct{775};
t2060 = ct{776};
t2061 = ct{777};
t2062 = ct{778};
t2065 = ct{779};
t2066 = ct{780};
t2067 = ct{781};
t2068 = ct{782};
t2069 = ct{783};
t207 = ct{784};
t2070 = ct{785};
t2071 = ct{786};
t2072 = ct{787};
t2073 = ct{788};
t2074 = ct{789};
t2076 = ct{790};
t2077 = ct{791};
t2078 = ct{792};
t2079 = ct{793};
t2080 = ct{794};
t2081 = ct{795};
t2082 = ct{796};
t2083 = ct{797};
t2084 = ct{798};
t2085 = ct{799};
t2086 = ct{800};
t2087 = ct{801};
t2088 = ct{802};
t2089 = ct{803};
t2091 = ct{804};
t2092 = ct{805};
t2093 = ct{806};
t2094 = ct{807};
t2095 = ct{808};
t2096 = ct{809};
t2097 = ct{810};
t2098 = ct{811};
t2099 = ct{812};
t21 = ct{813};
t2100 = ct{814};
t2101 = ct{815};
t2103 = ct{816};
t2104 = ct{817};
t2105 = ct{818};
t2106 = ct{819};
t2107 = ct{820};
t2108 = ct{821};
t2109 = ct{822};
t2110 = ct{823};
t2111 = ct{824};
t2113 = ct{825};
t2114 = ct{826};
t2115 = ct{827};
t2116 = ct{828};
t2117 = ct{829};
t2118 = ct{830};
t2119 = ct{831};
t2121 = ct{832};
t2125 = ct{833};
t2128 = ct{834};
t2129 = ct{835};
t2130 = ct{836};
t2131 = ct{837};
t2132 = ct{838};
t2133 = ct{839};
t2135 = ct{840};
t2136 = ct{841};
t2139 = ct{842};
t2140 = ct{843};
t2141 = ct{844};
t2142 = ct{845};
t2144 = ct{846};
t2147 = ct{847};
t2148 = ct{848};
t2149 = ct{849};
t215 = ct{850};
t2150 = ct{851};
t2151 = ct{852};
t2154 = ct{853};
t2155 = ct{854};
t2156 = ct{855};
t2157 = ct{856};
t2158 = ct{857};
t2159 = ct{858};
t2162 = ct{859};
t2163 = ct{860};
t2166 = ct{861};
t2167 = ct{862};
t2168 = ct{863};
t2169 = ct{864};
t2170 = ct{865};
t2171 = ct{866};
t2172 = ct{867};
t2174 = ct{868};
t2175 = ct{869};
t2176 = ct{870};
t2177 = ct{871};
t2178 = ct{872};
t2179 = ct{873};
t2180 = ct{874};
t2182 = ct{875};
t2184 = ct{876};
t2185 = ct{877};
t2186 = ct{878};
t2187 = ct{879};
t2189 = ct{880};
t2190 = ct{881};
t2191 = ct{882};
t2192 = ct{883};
t2194 = ct{884};
t2195 = ct{885};
t2196 = ct{886};
t22 = ct{887};
t2200 = ct{888};
t2201 = ct{889};
t2203 = ct{890};
t2204 = ct{891};
t2208 = ct{892};
t2209 = ct{893};
t2210 = ct{894};
t2212 = ct{895};
t2214 = ct{896};
t2217 = ct{897};
t2218 = ct{898};
t2219 = ct{899};
t2220 = ct{900};
t2221 = ct{901};
t2223 = ct{902};
t2225 = ct{903};
t2227 = ct{904};
t2228 = ct{905};
t2229 = ct{906};
t2231 = ct{907};
t2232 = ct{908};
t2236 = ct{909};
t2237 = ct{910};
t2239 = ct{911};
t224 = ct{912};
t2240 = ct{913};
t2243 = ct{914};
t2246 = ct{915};
t2249 = ct{916};
t225 = ct{917};
t2250 = ct{918};
t2251 = ct{919};
t2252 = ct{920};
t2254 = ct{921};
t2255 = ct{922};
t2256 = ct{923};
t2257 = ct{924};
t2264 = ct{925};
t2265 = ct{926};
t2266 = ct{927};
t2267 = ct{928};
t2269 = ct{929};
t227 = ct{930};
t2270 = ct{931};
t2271 = ct{932};
t2272 = ct{933};
t2273 = ct{934};
t2274 = ct{935};
t2276 = ct{936};
t2277 = ct{937};
t2278 = ct{938};
t2279 = ct{939};
t228 = ct{940};
t2280 = ct{941};
t2281 = ct{942};
t2282 = ct{943};
t2283 = ct{944};
t2284 = ct{945};
t2285 = ct{946};
t2286 = ct{947};
t2287 = ct{948};
t2291 = ct{949};
t2292 = ct{950};
t2294 = ct{951};
t2295 = ct{952};
t23 = ct{953};
t230 = ct{954};
t2302 = ct{955};
t2304 = ct{956};
t2305 = ct{957};
t2306 = ct{958};
t2307 = ct{959};
t2308 = ct{960};
t2309 = ct{961};
t231 = ct{962};
t2310 = ct{963};
t2311 = ct{964};
t2312 = ct{965};
t2314 = ct{966};
t2316 = ct{967};
t2317 = ct{968};
t2318 = ct{969};
t2321 = ct{970};
t2322 = ct{971};
t2323 = ct{972};
t2324 = ct{973};
t233 = ct{974};
t2331 = ct{975};
t2333 = ct{976};
t2334 = ct{977};
t2335 = ct{978};
t2336 = ct{979};
t2337 = ct{980};
t2338 = ct{981};
t2339 = ct{982};
t234 = ct{983};
t2340 = ct{984};
t2341 = ct{985};
t2342 = ct{986};
t2344 = ct{987};
t2347 = ct{988};
t2348 = ct{989};
t235 = ct{990};
t2350 = ct{991};
t2351 = ct{992};
t2355 = ct{993};
t2357 = ct{994};
t2358 = ct{995};
t2359 = ct{996};
t236 = ct{997};
t2361 = ct{998};
t2362 = ct{999};
t2363 = ct{1000};
t2364 = ct{1001};
t2365 = ct{1002};
t2366 = ct{1003};
t2368 = ct{1004};
t2369 = ct{1005};
t2370 = ct{1006};
t2371 = ct{1007};
t2372 = ct{1008};
t2373 = ct{1009};
t2374 = ct{1010};
t2375 = ct{1011};
t2376 = ct{1012};
t2377 = ct{1013};
t2378 = ct{1014};
t2379 = ct{1015};
t2381 = ct{1016};
t2382 = ct{1017};
t2384 = ct{1018};
t2385 = ct{1019};
t2387 = ct{1020};
t2388 = ct{1021};
t2389 = ct{1022};
t239 = ct{1023};
t2390 = ct{1024};
t2391 = ct{1025};
t2392 = ct{1026};
t2394 = ct{1027};
t2395 = ct{1028};
t2396 = ct{1029};
t2397 = ct{1030};
t24 = ct{1031};
t240 = ct{1032};
t2400 = ct{1033};
t2401 = ct{1034};
t2402 = ct{1035};
t2403 = ct{1036};
t2405 = ct{1037};
t2406 = ct{1038};
t2407 = ct{1039};
t2410 = ct{1040};
t2417 = ct{1041};
t2418 = ct{1042};
t2421 = ct{1043};
t2422 = ct{1044};
t2423 = ct{1045};
t2425 = ct{1046};
t2427 = ct{1047};
t2428 = ct{1048};
t2429 = ct{1049};
t243 = ct{1050};
t2430 = ct{1051};
t2431 = ct{1052};
t2434 = ct{1053};
t2435 = ct{1054};
t2437 = ct{1055};
t2438 = ct{1056};
t2439 = ct{1057};
t244 = ct{1058};
t2440 = ct{1059};
t2441 = ct{1060};
t2442 = ct{1061};
t2443 = ct{1062};
t2444 = ct{1063};
t2445 = ct{1064};
t2446 = ct{1065};
t2449 = ct{1066};
t2450 = ct{1067};
t2452 = ct{1068};
t2453 = ct{1069};
t2454 = ct{1070};
t2455 = ct{1071};
t2456 = ct{1072};
t2457 = ct{1073};
t2458 = ct{1074};
t2459 = ct{1075};
t2460 = ct{1076};
t2461 = ct{1077};
t2463 = ct{1078};
t2464 = ct{1079};
t2466 = ct{1080};
t2467 = ct{1081};
t2469 = ct{1082};
t2470 = ct{1083};
t2471 = ct{1084};
t2472 = ct{1085};
t2474 = ct{1086};
t2477 = ct{1087};
t2478 = ct{1088};
t2480 = ct{1089};
t2481 = ct{1090};
t2482 = ct{1091};
t2483 = ct{1092};
t2484 = ct{1093};
t2485 = ct{1094};
t2486 = ct{1095};
t2487 = ct{1096};
t2489 = ct{1097};
t249 = ct{1098};
t2495 = ct{1099};
t2497 = ct{1100};
t25 = ct{1101};
t2500 = ct{1102};
t2502 = ct{1103};
t2503 = ct{1104};
t2505 = ct{1105};
t2506 = ct{1106};
t2507 = ct{1107};
t2508 = ct{1108};
t2509 = ct{1109};
t2510 = ct{1110};
t2511 = ct{1111};
t2512 = ct{1112};
t2513 = ct{1113};
t2517 = ct{1114};
t2518 = ct{1115};
t2519 = ct{1116};
t2520 = ct{1117};
t2521 = ct{1118};
t2522 = ct{1119};
t2523 = ct{1120};
t2524 = ct{1121};
t2525 = ct{1122};
t2526 = ct{1123};
t2527 = ct{1124};
t2530 = ct{1125};
t2531 = ct{1126};
t2532 = ct{1127};
t2533 = ct{1128};
t2535 = ct{1129};
t2536 = ct{1130};
t2537 = ct{1131};
t2539 = ct{1132};
t2540 = ct{1133};
t2541 = ct{1134};
t2543 = ct{1135};
t2544 = ct{1136};
t2545 = ct{1137};
t2546 = ct{1138};
t2548 = ct{1139};
t2549 = ct{1140};
t2550 = ct{1141};
t2552 = ct{1142};
t2553 = ct{1143};
t2554 = ct{1144};
t2555 = ct{1145};
t2556 = ct{1146};
t2560 = ct{1147};
t2562 = ct{1148};
t2563 = ct{1149};
t2564 = ct{1150};
t2565 = ct{1151};
t2566 = ct{1152};
t2567 = ct{1153};
t2568 = ct{1154};
t2569 = ct{1155};
t257 = ct{1156};
t2570 = ct{1157};
t2571 = ct{1158};
t2574 = ct{1159};
t2575 = ct{1160};
t2576 = ct{1161};
t2577 = ct{1162};
t2578 = ct{1163};
t2579 = ct{1164};
t258 = ct{1165};
t2580 = ct{1166};
t2581 = ct{1167};
t2582 = ct{1168};
t2585 = ct{1169};
t2586 = ct{1170};
t2587 = ct{1171};
t2588 = ct{1172};
t2589 = ct{1173};
t2590 = ct{1174};
t2595 = ct{1175};
t2597 = ct{1176};
t2598 = ct{1177};
t2599 = ct{1178};
t26 = ct{1179};
t2600 = ct{1180};
t2601 = ct{1181};
t2602 = ct{1182};
t2603 = ct{1183};
t2604 = ct{1184};
t2606 = ct{1185};
t2607 = ct{1186};
t2608 = ct{1187};
t2611 = ct{1188};
t2612 = ct{1189};
t2615 = ct{1190};
t2616 = ct{1191};
t2617 = ct{1192};
t2627 = ct{1193};
t263 = ct{1194};
t2633 = ct{1195};
t2634 = ct{1196};
t2636 = ct{1197};
t2639 = ct{1198};
t2640 = ct{1199};
t2641 = ct{1200};
t2654 = ct{1201};
t2655 = ct{1202};
t2656 = ct{1203};
t2659 = ct{1204};
t266 = ct{1205};
t2666 = ct{1206};
t2668 = ct{1207};
t2669 = ct{1208};
t2671 = ct{1209};
t2673 = ct{1210};
t2675 = ct{1211};
t2676 = ct{1212};
t2677 = ct{1213};
t2678 = ct{1214};
t2680 = ct{1215};
t2681 = ct{1216};
t2682 = ct{1217};
t2684 = ct{1218};
t2685 = ct{1219};
t2686 = ct{1220};
t2688 = ct{1221};
t2692 = ct{1222};
t2693 = ct{1223};
t2694 = ct{1224};
t2695 = ct{1225};
t2699 = ct{1226};
t270 = ct{1227};
t2702 = ct{1228};
t2703 = ct{1229};
t2705 = ct{1230};
t2706 = ct{1231};
t2707 = ct{1232};
t2708 = ct{1233};
t2719 = ct{1234};
t2720 = ct{1235};
t2721 = ct{1236};
t2722 = ct{1237};
t2723 = ct{1238};
t2724 = ct{1239};
t2725 = ct{1240};
t2726 = ct{1241};
t273 = ct{1242};
t2733 = ct{1243};
t2734 = ct{1244};
t2739 = ct{1245};
t274 = ct{1246};
t2741 = ct{1247};
t2742 = ct{1248};
t2743 = ct{1249};
t2744 = ct{1250};
t2748 = ct{1251};
t2749 = ct{1252};
t275 = ct{1253};
t2752 = ct{1254};
t2759 = ct{1255};
t276 = ct{1256};
t2760 = ct{1257};
t2761 = ct{1258};
t2762 = ct{1259};
t2764 = ct{1260};
t2768 = ct{1261};
t2769 = ct{1262};
t277 = ct{1263};
t2770 = ct{1264};
t2771 = ct{1265};
t2773 = ct{1266};
t2774 = ct{1267};
t2775 = ct{1268};
t2776 = ct{1269};
t278 = ct{1270};
t2781 = ct{1271};
t2782 = ct{1272};
t2783 = ct{1273};
t2784 = ct{1274};
t2786 = ct{1275};
t2787 = ct{1276};
t2788 = ct{1277};
t2789 = ct{1278};
t2791 = ct{1279};
t2792 = ct{1280};
t280 = ct{1281};
t2806 = ct{1282};
t2808 = ct{1283};
t2815 = ct{1284};
t2820 = ct{1285};
t2821 = ct{1286};
t2829 = ct{1287};
t2830 = ct{1288};
t2831 = ct{1289};
t284 = ct{1290};
t2840 = ct{1291};
t2842 = ct{1292};
t2844 = ct{1293};
t2845 = ct{1294};
t2847 = ct{1295};
t2848 = ct{1296};
t2849 = ct{1297};
t2853 = ct{1298};
t2854 = ct{1299};
t2861 = ct{1300};
t2862 = ct{1301};
t2863 = ct{1302};
t2864 = ct{1303};
t2866 = ct{1304};
t2868 = ct{1305};
t2869 = ct{1306};
t287 = ct{1307};
t2879 = ct{1308};
t2884 = ct{1309};
t2886 = ct{1310};
t2888 = ct{1311};
t2892 = ct{1312};
t2898 = ct{1313};
t2899 = ct{1314};
t29 = ct{1315};
t290 = ct{1316};
t2900 = ct{1317};
t2901 = ct{1318};
t2902 = ct{1319};
t2903 = ct{1320};
t2908 = ct{1321};
t291 = ct{1322};
t292 = ct{1323};
t2920 = ct{1324};
t2923 = ct{1325};
t2925 = ct{1326};
t2926 = ct{1327};
t2928 = ct{1328};
t2929 = ct{1329};
t2930 = ct{1330};
t2937 = ct{1331};
t294 = ct{1332};
t2940 = ct{1333};
t2943 = ct{1334};
t2945 = ct{1335};
t2948 = ct{1336};
t2949 = ct{1337};
t2950 = ct{1338};
t2951 = ct{1339};
t2952 = ct{1340};
t2960 = ct{1341};
t2961 = ct{1342};
t2962 = ct{1343};
t2963 = ct{1344};
t2964 = ct{1345};
t2966 = ct{1346};
t2967 = ct{1347};
t2968 = ct{1348};
t2969 = ct{1349};
t297 = ct{1350};
t2970 = ct{1351};
t2971 = ct{1352};
t2975 = ct{1353};
t2976 = ct{1354};
t2980 = ct{1355};
t2982 = ct{1356};
t2983 = ct{1357};
t2984 = ct{1358};
t2985 = ct{1359};
t2986 = ct{1360};
t2988 = ct{1361};
t2989 = ct{1362};
t299 = ct{1363};
t2991 = ct{1364};
t2992 = ct{1365};
t2993 = ct{1366};
t2996 = ct{1367};
t2997 = ct{1368};
t3 = ct{1369};
t30 = ct{1370};
t300 = ct{1371};
t3003 = ct{1372};
t3004 = ct{1373};
t3007 = ct{1374};
t3010 = ct{1375};
t3011 = ct{1376};
t3013 = ct{1377};
t3014 = ct{1378};
t3019 = ct{1379};
t302 = ct{1380};
t3020 = ct{1381};
t3021 = ct{1382};
t3023 = ct{1383};
t3024 = ct{1384};
t3025 = ct{1385};
t3027 = ct{1386};
t3028 = ct{1387};
t3029 = ct{1388};
t303 = ct{1389};
t3030 = ct{1390};
t3031 = ct{1391};
t3032 = ct{1392};
t3033 = ct{1393};
t3034 = ct{1394};
t3035 = ct{1395};
t3036 = ct{1396};
t3038 = ct{1397};
t3039 = ct{1398};
t304 = ct{1399};
t3043 = ct{1400};
t3045 = ct{1401};
t3046 = ct{1402};
t3047 = ct{1403};
t305 = ct{1404};
t3051 = ct{1405};
t3052 = ct{1406};
t3053 = ct{1407};
t3055 = ct{1408};
t3056 = ct{1409};
t3057 = ct{1410};
t306 = ct{1411};
t3060 = ct{1412};
t3061 = ct{1413};
t3062 = ct{1414};
t3063 = ct{1415};
t3065 = ct{1416};
t3066 = ct{1417};
t3069 = ct{1418};
t3070 = ct{1419};
t3071 = ct{1420};
t3072 = ct{1421};
t3073 = ct{1422};
t3075 = ct{1423};
t3077 = ct{1424};
t3078 = ct{1425};
t3079 = ct{1426};
t3080 = ct{1427};
t3082 = ct{1428};
t3083 = ct{1429};
t3085 = ct{1430};
t3087 = ct{1431};
t309 = ct{1432};
t3090 = ct{1433};
t3091 = ct{1434};
t3092 = ct{1435};
t3093 = ct{1436};
t3094 = ct{1437};
t3095 = ct{1438};
t3098 = ct{1439};
t3099 = ct{1440};
t310 = ct{1441};
t3103 = ct{1442};
t3104 = ct{1443};
t3105 = ct{1444};
t3108 = ct{1445};
t3109 = ct{1446};
t311 = ct{1447};
t3112 = ct{1448};
t3113 = ct{1449};
t3119 = ct{1450};
t3120 = ct{1451};
t313 = ct{1452};
t314 = ct{1453};
t3142 = ct{1454};
t315 = ct{1455};
t3158 = ct{1456};
t316 = ct{1457};
t318 = ct{1458};
t319 = ct{1459};
t3191 = ct{1460};
t320 = ct{1461};
t3208 = ct{1462};
t3211 = ct{1463};
t3212 = ct{1464};
t3218 = ct{1465};
t3219 = ct{1466};
t322 = ct{1467};
t3225 = ct{1468};
t3228 = ct{1469};
t3230 = ct{1470};
t3231 = ct{1471};
t324 = ct{1472};
t3243 = ct{1473};
t3244 = ct{1474};
t325 = ct{1475};
t3251 = ct{1476};
t3252 = ct{1477};
t3255 = ct{1478};
t3257 = ct{1479};
t3258 = ct{1480};
t3259 = ct{1481};
t3261 = ct{1482};
t3273 = ct{1483};
t3274 = ct{1484};
t3275 = ct{1485};
t3279 = ct{1486};
t328 = ct{1487};
t3282 = ct{1488};
t3286 = ct{1489};
t3288 = ct{1490};
t3289 = ct{1491};
t3290 = ct{1492};
t3294 = ct{1493};
t3295 = ct{1494};
t3309 = ct{1495};
t3314 = ct{1496};
t3317 = ct{1497};
t3319 = ct{1498};
t3320 = ct{1499};
t3321 = ct{1500};
t3326 = ct{1501};
t3327 = ct{1502};
t3328 = ct{1503};
t3329 = ct{1504};
t333 = ct{1505};
t3330 = ct{1506};
t3331 = ct{1507};
t3333 = ct{1508};
t3334 = ct{1509};
t3335 = ct{1510};
t3343 = ct{1511};
t336 = ct{1512};
t3363 = ct{1513};
t3364 = ct{1514};
t3365 = ct{1515};
t3367 = ct{1516};
t3368 = ct{1517};
t3369 = ct{1518};
t337 = ct{1519};
t3370 = ct{1520};
t3371 = ct{1521};
t3372 = ct{1522};
t3373 = ct{1523};
t3374 = ct{1524};
t3375 = ct{1525};
t3376 = ct{1526};
t3378 = ct{1527};
t3379 = ct{1528};
t3380 = ct{1529};
t3381 = ct{1530};
t3382 = ct{1531};
t3389 = ct{1532};
t3390 = ct{1533};
t3391 = ct{1534};
t3392 = ct{1535};
t3393 = ct{1536};
t3394 = ct{1537};
t3395 = ct{1538};
t3397 = ct{1539};
t34 = ct{1540};
t340 = ct{1541};
t3400 = ct{1542};
t3401 = ct{1543};
t3402 = ct{1544};
t3403 = ct{1545};
t3409 = ct{1546};
t3416 = ct{1547};
t3417 = ct{1548};
t3418 = ct{1549};
t3419 = ct{1550};
t3420 = ct{1551};
t3426 = ct{1552};
t3430 = ct{1553};
t3432 = ct{1554};
t3434 = ct{1555};
t3435 = ct{1556};
t3437 = ct{1557};
t3438 = ct{1558};
t3439 = ct{1559};
t344 = ct{1560};
t3440 = ct{1561};
t3442 = ct{1562};
t3443 = ct{1563};
t3444 = ct{1564};
t3445 = ct{1565};
t3446 = ct{1566};
t3447 = ct{1567};
t3449 = ct{1568};
t3450 = ct{1569};
t3452 = ct{1570};
t3453 = ct{1571};
t3454 = ct{1572};
t3455 = ct{1573};
t3456 = ct{1574};
t3459 = ct{1575};
t346 = ct{1576};
t3462 = ct{1577};
t3463 = ct{1578};
t3466 = ct{1579};
t3468 = ct{1580};
t3469 = ct{1581};
t347 = ct{1582};
t3470 = ct{1583};
t3472 = ct{1584};
t3473 = ct{1585};
t3475 = ct{1586};
t3477 = ct{1587};
t3479 = ct{1588};
t348 = ct{1589};
t3481 = ct{1590};
t3483 = ct{1591};
t3486 = ct{1592};
t3489 = ct{1593};
t349 = ct{1594};
t3492 = ct{1595};
t350 = ct{1596};
t3500 = ct{1597};
t3501 = ct{1598};
t3506 = ct{1599};
t3507 = ct{1600};
t3509 = ct{1601};
t3514 = ct{1602};
t3515 = ct{1603};
t3516 = ct{1604};
t3517 = ct{1605};
t3519 = ct{1606};
t352 = ct{1607};
t3520 = ct{1608};
t3521 = ct{1609};
t3522 = ct{1610};
t3523 = ct{1611};
t3524 = ct{1612};
t353 = ct{1613};
t3530 = ct{1614};
t3532 = ct{1615};
t3533 = ct{1616};
t3534 = ct{1617};
t3535 = ct{1618};
t3538 = ct{1619};
t3539 = ct{1620};
t3541 = ct{1621};
t3544 = ct{1622};
t3546 = ct{1623};
t3548 = ct{1624};
t3549 = ct{1625};
t3553 = ct{1626};
t3556 = ct{1627};
t356 = ct{1628};
t3560 = ct{1629};
t3568 = ct{1630};
t3569 = ct{1631};
t357 = ct{1632};
t3572 = ct{1633};
t3573 = ct{1634};
t3574 = ct{1635};
t3575 = ct{1636};
t3576 = ct{1637};
t3578 = ct{1638};
t3579 = ct{1639};
t358 = ct{1640};
t3581 = ct{1641};
t3582 = ct{1642};
t3583 = ct{1643};
t3584 = ct{1644};
t3585 = ct{1645};
t359 = ct{1646};
t3590 = ct{1647};
t3596 = ct{1648};
t3597 = ct{1649};
t3601 = ct{1650};
t3602 = ct{1651};
t3604 = ct{1652};
t3607 = ct{1653};
t3609 = ct{1654};
t361 = ct{1655};
t3613 = ct{1656};
t3616 = ct{1657};
t3617 = ct{1658};
t3618 = ct{1659};
t362 = ct{1660};
t3622 = ct{1661};
t3629 = ct{1662};
t3630 = ct{1663};
t3637 = ct{1664};
t3638 = ct{1665};
t3639 = ct{1666};
t3641 = ct{1667};
t3643 = ct{1668};
t3646 = ct{1669};
t3647 = ct{1670};
t3649 = ct{1671};
t365 = ct{1672};
t3650 = ct{1673};
t3652 = ct{1674};
t3653 = ct{1675};
t3654 = ct{1676};
t3659 = ct{1677};
t3660 = ct{1678};
t3662 = ct{1679};
t3663 = ct{1680};
t3668 = ct{1681};
t3676 = ct{1682};
t368 = ct{1683};
t3680 = ct{1684};
t3682 = ct{1685};
t3686 = ct{1686};
t369 = ct{1687};
t3691 = ct{1688};
t3695 = ct{1689};
t3697 = ct{1690};
t3701 = ct{1691};
t3709 = ct{1692};
t371 = ct{1693};
t3714 = ct{1694};
t3716 = ct{1695};
t3717 = ct{1696};
t372 = ct{1697};
t3722 = ct{1698};
t3726 = ct{1699};
t3729 = ct{1700};
t373 = ct{1701};
t3730 = ct{1702};
t3736 = ct{1703};
t3737 = ct{1704};
t3738 = ct{1705};
t374 = ct{1706};
t3743 = ct{1707};
t3744 = ct{1708};
t3747 = ct{1709};
t3748 = ct{1710};
t3750 = ct{1711};
t3751 = ct{1712};
t3756 = ct{1713};
t377 = ct{1714};
t3774 = ct{1715};
t378 = ct{1716};
t3789 = ct{1717};
t379 = ct{1718};
t3798 = ct{1719};
t380 = ct{1720};
t3815 = ct{1721};
t382 = ct{1722};
t3822 = ct{1723};
t3824 = ct{1724};
t3825 = ct{1725};
t3834 = ct{1726};
t3835 = ct{1727};
t3839 = ct{1728};
t384 = ct{1729};
t3846 = ct{1730};
t3847 = ct{1731};
t3852 = ct{1732};
t386 = ct{1733};
t387 = ct{1734};
t388 = ct{1735};
t3889 = ct{1736};
t3892 = ct{1737};
t3898 = ct{1738};
t3899 = ct{1739};
t391 = ct{1740};
t3915 = ct{1741};
t392 = ct{1742};
t395 = ct{1743};
t3950 = ct{1744};
t3951 = ct{1745};
t3958 = ct{1746};
t3959 = ct{1747};
t396 = ct{1748};
t4 = ct{1749};
t400 = ct{1750};
t4001 = ct{1751};
t4002 = ct{1752};
t4004 = ct{1753};
t4007 = ct{1754};
t401 = ct{1755};
t402 = ct{1756};
t4028 = ct{1757};
t4029 = ct{1758};
t403 = ct{1759};
t4030 = ct{1760};
t4031 = ct{1761};
t4032 = ct{1762};
t4033 = ct{1763};
t4039 = ct{1764};
t4040 = ct{1765};
t4041 = ct{1766};
t4042 = ct{1767};
t4043 = ct{1768};
t4044 = ct{1769};
t4045 = ct{1770};
t4051 = ct{1771};
t4052 = ct{1772};
t4058 = ct{1773};
t406 = ct{1774};
t410 = ct{1775};
t4105 = ct{1776};
t411 = ct{1777};
t4113 = ct{1778};
t4114 = ct{1779};
t4117 = ct{1780};
t4118 = ct{1781};
t412 = ct{1782};
t4123 = ct{1783};
t413 = ct{1784};
t414 = ct{1785};
t4143 = ct{1786};
t4144 = ct{1787};
t4145 = ct{1788};
t415 = ct{1789};
t4150 = ct{1790};
t4152 = ct{1791};
t4153 = ct{1792};
t4155 = ct{1793};
t416 = ct{1794};
t4160 = ct{1795};
t4164 = ct{1796};
t4165 = ct{1797};
t417 = ct{1798};
t4170 = ct{1799};
t4174 = ct{1800};
t4177 = ct{1801};
t4178 = ct{1802};
t4179 = ct{1803};
t418 = ct{1804};
t4180 = ct{1805};
t4181 = ct{1806};
t4182 = ct{1807};
t4183 = ct{1808};
t4184 = ct{1809};
t4185 = ct{1810};
t4186 = ct{1811};
t4187 = ct{1812};
t4188 = ct{1813};
t4189 = ct{1814};
t4190 = ct{1815};
t4191 = ct{1816};
t4192 = ct{1817};
t4193 = ct{1818};
t4194 = ct{1819};
t4196 = ct{1820};
t4197 = ct{1821};
t420 = ct{1822};
t4200 = ct{1823};
t4203 = ct{1824};
t4204 = ct{1825};
t4205 = ct{1826};
t4206 = ct{1827};
t4207 = ct{1828};
t4208 = ct{1829};
t4209 = ct{1830};
t4211 = ct{1831};
t4212 = ct{1832};
t4213 = ct{1833};
t4214 = ct{1834};
t4216 = ct{1835};
t422 = ct{1836};
t4221 = ct{1837};
t4228 = ct{1838};
t4229 = ct{1839};
t423 = ct{1840};
t4230 = ct{1841};
t4231 = ct{1842};
t4232 = ct{1843};
t4233 = ct{1844};
t4235 = ct{1845};
t4236 = ct{1846};
t4237 = ct{1847};
t4239 = ct{1848};
t424 = ct{1849};
t4240 = ct{1850};
t4242 = ct{1851};
t4243 = ct{1852};
t4246 = ct{1853};
t4249 = ct{1854};
t425 = ct{1855};
t4255 = ct{1856};
t4256 = ct{1857};
t4257 = ct{1858};
t4258 = ct{1859};
t4259 = ct{1860};
t4260 = ct{1861};
t4261 = ct{1862};
t4262 = ct{1863};
t4265 = ct{1864};
t4266 = ct{1865};
t4268 = ct{1866};
t427 = ct{1867};
t4271 = ct{1868};
t4272 = ct{1869};
t4275 = ct{1870};
t4277 = ct{1871};
t4278 = ct{1872};
t4279 = ct{1873};
t428 = ct{1874};
t4283 = ct{1875};
t4284 = ct{1876};
t4287 = ct{1877};
t4288 = ct{1878};
t4289 = ct{1879};
t429 = ct{1880};
t4290 = ct{1881};
t4292 = ct{1882};
t4293 = ct{1883};
t4294 = ct{1884};
t4295 = ct{1885};
t4296 = ct{1886};
t4297 = ct{1887};
t4298 = ct{1888};
t4299 = ct{1889};
t4300 = ct{1890};
t4301 = ct{1891};
t4304 = ct{1892};
t4308 = ct{1893};
t4309 = ct{1894};
t431 = ct{1895};
t4310 = ct{1896};
t4311 = ct{1897};
t4313 = ct{1898};
t4315 = ct{1899};
t4316 = ct{1900};
t4317 = ct{1901};
t4319 = ct{1902};
t432 = ct{1903};
t4320 = ct{1904};
t4321 = ct{1905};
t4323 = ct{1906};
t4325 = ct{1907};
t4326 = ct{1908};
t4328 = ct{1909};
t433 = ct{1910};
t4330 = ct{1911};
t4333 = ct{1912};
t4334 = ct{1913};
t4335 = ct{1914};
t4336 = ct{1915};
t4337 = ct{1916};
t4338 = ct{1917};
t4339 = ct{1918};
t434 = ct{1919};
t4341 = ct{1920};
t4342 = ct{1921};
t4343 = ct{1922};
t4344 = ct{1923};
t4345 = ct{1924};
t4346 = ct{1925};
t4347 = ct{1926};
t435 = ct{1927};
t4351 = ct{1928};
t4353 = ct{1929};
t4355 = ct{1930};
t436 = ct{1931};
t4361 = ct{1932};
t4365 = ct{1933};
t4367 = ct{1934};
t4369 = ct{1935};
t437 = ct{1936};
t4370 = ct{1937};
t4371 = ct{1938};
t4372 = ct{1939};
t4375 = ct{1940};
t4377 = ct{1941};
t4379 = ct{1942};
t438 = ct{1943};
t4382 = ct{1944};
t4385 = ct{1945};
t4387 = ct{1946};
t439 = ct{1947};
t4390 = ct{1948};
t4391 = ct{1949};
t4392 = ct{1950};
t4394 = ct{1951};
t4395 = ct{1952};
t4396 = ct{1953};
t4397 = ct{1954};
t44 = ct{1955};
t440 = ct{1956};
t4401 = ct{1957};
t4402 = ct{1958};
t4403 = ct{1959};
t4404 = ct{1960};
t4405 = ct{1961};
t4406 = ct{1962};
t4407 = ct{1963};
t4408 = ct{1964};
t441 = ct{1965};
t4410 = ct{1966};
t4411 = ct{1967};
t4412 = ct{1968};
t4413 = ct{1969};
t4417 = ct{1970};
t4419 = ct{1971};
t442 = ct{1972};
t4420 = ct{1973};
t4421 = ct{1974};
t4422 = ct{1975};
t4425 = ct{1976};
t4426 = ct{1977};
t4428 = ct{1978};
t4429 = ct{1979};
t4431 = ct{1980};
t4432 = ct{1981};
t4435 = ct{1982};
t4436 = ct{1983};
t444 = ct{1984};
t4440 = ct{1985};
t4442 = ct{1986};
t4443 = ct{1987};
t4444 = ct{1988};
t4445 = ct{1989};
t4446 = ct{1990};
t4448 = ct{1991};
t4449 = ct{1992};
t445 = ct{1993};
t4450 = ct{1994};
t4452 = ct{1995};
t4453 = ct{1996};
t4455 = ct{1997};
t4457 = ct{1998};
t4459 = ct{1999};
t4462 = ct{2000};
t4464 = ct{2001};
t4469 = ct{2002};
t4473 = ct{2003};
t4478 = ct{2004};
t4479 = ct{2005};
t448 = ct{2006};
t4480 = ct{2007};
t4481 = ct{2008};
t4483 = ct{2009};
t4484 = ct{2010};
t4485 = ct{2011};
t4486 = ct{2012};
t4488 = ct{2013};
t449 = ct{2014};
t4491 = ct{2015};
t4492 = ct{2016};
t4493 = ct{2017};
t4495 = ct{2018};
t4498 = ct{2019};
t45 = ct{2020};
t450 = ct{2021};
t4501 = ct{2022};
t4502 = ct{2023};
t4504 = ct{2024};
t4506 = ct{2025};
t4508 = ct{2026};
t4509 = ct{2027};
t4513 = ct{2028};
t4516 = ct{2029};
t4517 = ct{2030};
t4519 = ct{2031};
t452 = ct{2032};
t4520 = ct{2033};
t4522 = ct{2034};
t4524 = ct{2035};
t4525 = ct{2036};
t453 = ct{2037};
t4530 = ct{2038};
t4532 = ct{2039};
t4533 = ct{2040};
t454 = ct{2041};
t4540 = ct{2042};
t4542 = ct{2043};
t4543 = ct{2044};
t4547 = ct{2045};
t4548 = ct{2046};
t4549 = ct{2047};
t4551 = ct{2048};
t4554 = ct{2049};
t4555 = ct{2050};
t4557 = ct{2051};
t4558 = ct{2052};
t4559 = ct{2053};
t4561 = ct{2054};
t4562 = ct{2055};
t4563 = ct{2056};
t4566 = ct{2057};
t4567 = ct{2058};
t4568 = ct{2059};
t4569 = ct{2060};
t457 = ct{2061};
t4570 = ct{2062};
t4571 = ct{2063};
t4572 = ct{2064};
t4574 = ct{2065};
t4575 = ct{2066};
t4577 = ct{2067};
t4579 = ct{2068};
t458 = ct{2069};
t4581 = ct{2070};
t4582 = ct{2071};
t4583 = ct{2072};
t4584 = ct{2073};
t4588 = ct{2074};
t4589 = ct{2075};
t459 = ct{2076};
t4590 = ct{2077};
t4591 = ct{2078};
t4595 = ct{2079};
t4596 = ct{2080};
t46 = ct{2081};
t460 = ct{2082};
t4600 = ct{2083};
t4601 = ct{2084};
t4605 = ct{2085};
t4606 = ct{2086};
t4607 = ct{2087};
t461 = ct{2088};
t4611 = ct{2089};
t4614 = ct{2090};
t4616 = ct{2091};
t4617 = ct{2092};
t462 = ct{2093};
t4621 = ct{2094};
t4622 = ct{2095};
t4625 = ct{2096};
t4626 = ct{2097};
t4628 = ct{2098};
t4629 = ct{2099};
t463 = ct{2100};
t4630 = ct{2101};
t4632 = ct{2102};
t4633 = ct{2103};
t4634 = ct{2104};
t4636 = ct{2105};
t4637 = ct{2106};
t4638 = ct{2107};
t4639 = ct{2108};
t464 = ct{2109};
t4640 = ct{2110};
t4641 = ct{2111};
t4642 = ct{2112};
t4643 = ct{2113};
t4644 = ct{2114};
t4645 = ct{2115};
t4646 = ct{2116};
t4647 = ct{2117};
t4649 = ct{2118};
t465 = ct{2119};
t4650 = ct{2120};
t4651 = ct{2121};
t4652 = ct{2122};
t4653 = ct{2123};
t4656 = ct{2124};
t4657 = ct{2125};
t4658 = ct{2126};
t466 = ct{2127};
t4660 = ct{2128};
t4661 = ct{2129};
t4662 = ct{2130};
t4663 = ct{2131};
t4666 = ct{2132};
t4667 = ct{2133};
t4669 = ct{2134};
t4672 = ct{2135};
t4673 = ct{2136};
t4674 = ct{2137};
t4675 = ct{2138};
t468 = ct{2139};
t4688 = ct{2140};
t469 = ct{2141};
t4691 = ct{2142};
t4692 = ct{2143};
t4693 = ct{2144};
t4694 = ct{2145};
t4695 = ct{2146};
t4696 = ct{2147};
t4697 = ct{2148};
t47 = ct{2149};
t470 = ct{2150};
t4707 = ct{2151};
t4708 = ct{2152};
t4709 = ct{2153};
t471 = ct{2154};
t4711 = ct{2155};
t4713 = ct{2156};
t4716 = ct{2157};
t472 = ct{2158};
t4722 = ct{2159};
t4723 = ct{2160};
t4724 = ct{2161};
t4725 = ct{2162};
t4726 = ct{2163};
t4727 = ct{2164};
t4728 = ct{2165};
t4731 = ct{2166};
t4732 = ct{2167};
t4733 = ct{2168};
t4734 = ct{2169};
t4737 = ct{2170};
t4740 = ct{2171};
t4741 = ct{2172};
t4742 = ct{2173};
t4745 = ct{2174};
t4747 = ct{2175};
t4748 = ct{2176};
t4749 = ct{2177};
t475 = ct{2178};
t4752 = ct{2179};
t4753 = ct{2180};
t4754 = ct{2181};
t4755 = ct{2182};
t4756 = ct{2183};
t4758 = ct{2184};
t4759 = ct{2185};
t4760 = ct{2186};
t4761 = ct{2187};
t4763 = ct{2188};
t4766 = ct{2189};
t4769 = ct{2190};
t477 = ct{2191};
t4770 = ct{2192};
t4777 = ct{2193};
t4778 = ct{2194};
t4782 = ct{2195};
t4783 = ct{2196};
t4785 = ct{2197};
t4786 = ct{2198};
t4788 = ct{2199};
t4789 = ct{2200};
t479 = ct{2201};
t4790 = ct{2202};
t4794 = ct{2203};
t4795 = ct{2204};
t4796 = ct{2205};
t4797 = ct{2206};
t4798 = ct{2207};
t4799 = ct{2208};
t480 = ct{2209};
t4800 = ct{2210};
t4801 = ct{2211};
t4803 = ct{2212};
t4804 = ct{2213};
t4805 = ct{2214};
t4807 = ct{2215};
t4808 = ct{2216};
t481 = ct{2217};
t4811 = ct{2218};
t4813 = ct{2219};
t4814 = ct{2220};
t4815 = ct{2221};
t4818 = ct{2222};
t482 = ct{2223};
t4820 = ct{2224};
t4824 = ct{2225};
t4825 = ct{2226};
t4827 = ct{2227};
t4828 = ct{2228};
t483 = ct{2229};
t4830 = ct{2230};
t4832 = ct{2231};
t4833 = ct{2232};
t4834 = ct{2233};
t4835 = ct{2234};
t4837 = ct{2235};
t4839 = ct{2236};
t484 = ct{2237};
t4841 = ct{2238};
t4842 = ct{2239};
t4845 = ct{2240};
t4846 = ct{2241};
t4849 = ct{2242};
t485 = ct{2243};
t4852 = ct{2244};
t486 = ct{2245};
t4861 = ct{2246};
t4862 = ct{2247};
t4864 = ct{2248};
t4865 = ct{2249};
t4866 = ct{2250};
t4867 = ct{2251};
t4871 = ct{2252};
t4872 = ct{2253};
t4873 = ct{2254};
t4876 = ct{2255};
t4877 = ct{2256};
t4878 = ct{2257};
t4879 = ct{2258};
t488 = ct{2259};
t4882 = ct{2260};
t4883 = ct{2261};
t4884 = ct{2262};
t4886 = ct{2263};
t4887 = ct{2264};
t489 = ct{2265};
t4895 = ct{2266};
t4897 = ct{2267};
t4899 = ct{2268};
t4900 = ct{2269};
t4908 = ct{2270};
t4909 = ct{2271};
t491 = ct{2272};
t4910 = ct{2273};
t4911 = ct{2274};
t4913 = ct{2275};
t4915 = ct{2276};
t4916 = ct{2277};
t4919 = ct{2278};
t492 = ct{2279};
t4920 = ct{2280};
t4923 = ct{2281};
t4924 = ct{2282};
t4925 = ct{2283};
t4927 = ct{2284};
t4928 = ct{2285};
t493 = ct{2286};
t4930 = ct{2287};
t4933 = ct{2288};
t4934 = ct{2289};
t4937 = ct{2290};
t4938 = ct{2291};
t494 = ct{2292};
t4941 = ct{2293};
t4942 = ct{2294};
t4943 = ct{2295};
t4944 = ct{2296};
t4945 = ct{2297};
t4946 = ct{2298};
t4948 = ct{2299};
t4951 = ct{2300};
t4955 = ct{2301};
t4956 = ct{2302};
t4957 = ct{2303};
t496 = ct{2304};
t4962 = ct{2305};
t4964 = ct{2306};
t4969 = ct{2307};
t497 = ct{2308};
t4970 = ct{2309};
t4973 = ct{2310};
t4974 = ct{2311};
t4976 = ct{2312};
t498 = ct{2313};
t4980 = ct{2314};
t4981 = ct{2315};
t4982 = ct{2316};
t4983 = ct{2317};
t4986 = ct{2318};
t4987 = ct{2319};
t4988 = ct{2320};
t499 = ct{2321};
t4991 = ct{2322};
t4993 = ct{2323};
t4996 = ct{2324};
t4998 = ct{2325};
t4999 = ct{2326};
t5 = ct{2327};
t50 = ct{2328};
t500 = ct{2329};
t5000 = ct{2330};
t5001 = ct{2331};
t5004 = ct{2332};
t5006 = ct{2333};
t5008 = ct{2334};
t501 = ct{2335};
t5019 = ct{2336};
t502 = ct{2337};
t5021 = ct{2338};
t5022 = ct{2339};
t5023 = ct{2340};
t5026 = ct{2341};
t5027 = ct{2342};
t5029 = ct{2343};
t503 = ct{2344};
t5034 = ct{2345};
t5035 = ct{2346};
t5036 = ct{2347};
t5038 = ct{2348};
t504 = ct{2349};
t5045 = ct{2350};
t5046 = ct{2351};
t505 = ct{2352};
t5051 = ct{2353};
t5052 = ct{2354};
t5053 = ct{2355};
t506 = ct{2356};
t5060 = ct{2357};
t5062 = ct{2358};
t5063 = ct{2359};
t5064 = ct{2360};
t5065 = ct{2361};
t5066 = ct{2362};
t5069 = ct{2363};
t507 = ct{2364};
t5071 = ct{2365};
t5072 = ct{2366};
t5073 = ct{2367};
t5078 = ct{2368};
t508 = ct{2369};
t5080 = ct{2370};
t5082 = ct{2371};
t5083 = ct{2372};
t5084 = ct{2373};
t5085 = ct{2374};
t509 = ct{2375};
t5091 = ct{2376};
t5093 = ct{2377};
t5095 = ct{2378};
t5096 = ct{2379};
t5097 = ct{2380};
t5098 = ct{2381};
t5099 = ct{2382};
t510 = ct{2383};
t5100 = ct{2384};
t5102 = ct{2385};
t5107 = ct{2386};
t511 = ct{2387};
t5111 = ct{2388};
t5112 = ct{2389};
t5113 = ct{2390};
t5114 = ct{2391};
t5116 = ct{2392};
t5119 = ct{2393};
t512 = ct{2394};
t5120 = ct{2395};
t5122 = ct{2396};
t5127 = ct{2397};
t513 = ct{2398};
t5130 = ct{2399};
t5139 = ct{2400};
t514 = ct{2401};
t5142 = ct{2402};
t5147 = ct{2403};
t5149 = ct{2404};
t5150 = ct{2405};
t5151 = ct{2406};
t5154 = ct{2407};
t5158 = ct{2408};
t516 = ct{2409};
t5165 = ct{2410};
t517 = ct{2411};
t5171 = ct{2412};
t5172 = ct{2413};
t5176 = ct{2414};
t5179 = ct{2415};
t518 = ct{2416};
t5180 = ct{2417};
t5181 = ct{2418};
t5183 = ct{2419};
t5184 = ct{2420};
t5185 = ct{2421};
t5186 = ct{2422};
t5187 = ct{2423};
t5192 = ct{2424};
t5193 = ct{2425};
t5199 = ct{2426};
t520 = ct{2427};
t5200 = ct{2428};
t5203 = ct{2429};
t5204 = ct{2430};
t5205 = ct{2431};
t5208 = ct{2432};
t521 = ct{2433};
t5215 = ct{2434};
t5216 = ct{2435};
t5217 = ct{2436};
t522 = ct{2437};
t5222 = ct{2438};
t5223 = ct{2439};
t5224 = ct{2440};
t5227 = ct{2441};
t523 = ct{2442};
t5236 = ct{2443};
t5237 = ct{2444};
t5238 = ct{2445};
t5239 = ct{2446};
t524 = ct{2447};
t5240 = ct{2448};
t5244 = ct{2449};
t5245 = ct{2450};
t525 = ct{2451};
t5250 = ct{2452};
t5252 = ct{2453};
t5258 = ct{2454};
t526 = ct{2455};
t5267 = ct{2456};
t527 = ct{2457};
t5270 = ct{2458};
t5271 = ct{2459};
t5279 = ct{2460};
t528 = ct{2461};
t5280 = ct{2462};
t5281 = ct{2463};
t5285 = ct{2464};
t529 = ct{2465};
t5293 = ct{2466};
t5294 = ct{2467};
t53 = ct{2468};
t530 = ct{2469};
t5305 = ct{2470};
t531 = ct{2471};
t5318 = ct{2472};
t5319 = ct{2473};
t532 = ct{2474};
t5321 = ct{2475};
t5324 = ct{2476};
t5325 = ct{2477};
t5327 = ct{2478};
t5328 = ct{2479};
t533 = ct{2480};
t5331 = ct{2481};
t5332 = ct{2482};
t534 = ct{2483};
t535 = ct{2484};
t5353 = ct{2485};
t5355 = ct{2486};
t5356 = ct{2487};
t5358 = ct{2488};
t536 = ct{2489};
t5361 = ct{2490};
t5362 = ct{2491};
t5364 = ct{2492};
t5368 = ct{2493};
t537 = ct{2494};
t5372 = ct{2495};
t5373 = ct{2496};
t5376 = ct{2497};
t5378 = ct{2498};
t538 = ct{2499};
t5387 = ct{2500};
t5389 = ct{2501};
t539 = ct{2502};
t5390 = ct{2503};
t5391 = ct{2504};
t5392 = ct{2505};
t5393 = ct{2506};
t5394 = ct{2507};
t540 = ct{2508};
t5402 = ct{2509};
t5404 = ct{2510};
t5409 = ct{2511};
t5416 = ct{2512};
t5420 = ct{2513};
t5424 = ct{2514};
t5429 = ct{2515};
t543 = ct{2516};
t5430 = ct{2517};
t5434 = ct{2518};
t5435 = ct{2519};
t5436 = ct{2520};
t5439 = ct{2521};
t544 = ct{2522};
t5440 = ct{2523};
t5441 = ct{2524};
t5445 = ct{2525};
t5449 = ct{2526};
t545 = ct{2527};
t5450 = ct{2528};
t5451 = ct{2529};
t5452 = ct{2530};
t5453 = ct{2531};
t5455 = ct{2532};
t5456 = ct{2533};
t5457 = ct{2534};
t546 = ct{2535};
t5467 = ct{2536};
t5468 = ct{2537};
t5469 = ct{2538};
t547 = ct{2539};
t5470 = ct{2540};
t5471 = ct{2541};
t5472 = ct{2542};
t5473 = ct{2543};
t5474 = ct{2544};
t5475 = ct{2545};
t5476 = ct{2546};
t5477 = ct{2547};
t5478 = ct{2548};
t548 = ct{2549};
t5489 = ct{2550};
t549 = ct{2551};
t5490 = ct{2552};
t5493 = ct{2553};
t5494 = ct{2554};
t5497 = ct{2555};
t5499 = ct{2556};
t5501 = ct{2557};
t5508 = ct{2558};
t551 = ct{2559};
t5510 = ct{2560};
t5512 = ct{2561};
t5516 = ct{2562};
t5517 = ct{2563};
t552 = ct{2564};
t5521 = ct{2565};
t553 = ct{2566};
t5532 = ct{2567};
t5535 = ct{2568};
t554 = ct{2569};
t5540 = ct{2570};
t5547 = ct{2571};
t555 = ct{2572};
t5557 = ct{2573};
t5558 = ct{2574};
t556 = ct{2575};
t557 = ct{2576};
t5574 = ct{2577};
t5578 = ct{2578};
t5579 = ct{2579};
t558 = ct{2580};
t5582 = ct{2581};
t5586 = ct{2582};
t559 = ct{2583};
t5590 = ct{2584};
t5593 = ct{2585};
t5596 = ct{2586};
t560 = ct{2587};
t5604 = ct{2588};
t5607 = ct{2589};
t561 = ct{2590};
t5612 = ct{2591};
t562 = ct{2592};
t5629 = ct{2593};
t563 = ct{2594};
t5634 = ct{2595};
t5635 = ct{2596};
t564 = ct{2597};
t567 = ct{2598};
t568 = ct{2599};
t5688 = ct{2600};
t569 = ct{2601};
t57 = ct{2602};
t570 = ct{2603};
t571 = ct{2604};
t572 = ct{2605};
t573 = ct{2606};
t574 = ct{2607};
t5741 = ct{2608};
t5743 = ct{2609};
t576 = ct{2610};
t577 = ct{2611};
t5777 = ct{2612};
t5779 = ct{2613};
t578 = ct{2614};
t5780 = ct{2615};
t5782 = ct{2616};
t579 = ct{2617};
t58 = ct{2618};
t580 = ct{2619};
t581 = ct{2620};
t582 = ct{2621};
t5826 = ct{2622};
t583 = ct{2623};
t584 = ct{2624};
t586 = ct{2625};
t587 = ct{2626};
t5886 = ct{2627};
t5887 = ct{2628};
t589 = ct{2629};
t5894 = ct{2630};
t59 = ct{2631};
t590 = ct{2632};
t591 = ct{2633};
t592 = ct{2634};
t593 = ct{2635};
t594 = ct{2636};
t595 = ct{2637};
t596 = ct{2638};
t597 = ct{2639};
t6 = ct{2640};
t60 = ct{2641};
t600 = ct{2642};
t602 = ct{2643};
t603 = ct{2644};
t604 = ct{2645};
t605 = ct{2646};
t609 = ct{2647};
t610 = ct{2648};
t611 = ct{2649};
t612 = ct{2650};
t613 = ct{2651};
t614 = ct{2652};
t615 = ct{2653};
t616 = ct{2654};
t618 = ct{2655};
t619 = ct{2656};
t622 = ct{2657};
t623 = ct{2658};
t624 = ct{2659};
t625 = ct{2660};
t626 = ct{2661};
t627 = ct{2662};
t628 = ct{2663};
t629 = ct{2664};
t63 = ct{2665};
t630 = ct{2666};
t631 = ct{2667};
t633 = ct{2668};
t634 = ct{2669};
t635 = ct{2670};
t636 = ct{2671};
t637 = ct{2672};
t638 = ct{2673};
t639 = ct{2674};
t640 = ct{2675};
t641 = ct{2676};
t642 = ct{2677};
t643 = ct{2678};
t648 = ct{2679};
t649 = ct{2680};
t650 = ct{2681};
t653 = ct{2682};
t654 = ct{2683};
t655 = ct{2684};
t656 = ct{2685};
t657 = ct{2686};
t658 = ct{2687};
t660 = ct{2688};
t662 = ct{2689};
t663 = ct{2690};
t664 = ct{2691};
t665 = ct{2692};
t667 = ct{2693};
t668 = ct{2694};
t673 = ct{2695};
t674 = ct{2696};
t675 = ct{2697};
t676 = ct{2698};
t678 = ct{2699};
t679 = ct{2700};
t681 = ct{2701};
t682 = ct{2702};
t683 = ct{2703};
t684 = ct{2704};
t685 = ct{2705};
t686 = ct{2706};
t687 = ct{2707};
t688 = ct{2708};
t689 = ct{2709};
t693 = ct{2710};
t694 = ct{2711};
t695 = ct{2712};
t696 = ct{2713};
t697 = ct{2714};
t698 = ct{2715};
t7 = ct{2716};
t700 = ct{2717};
t702 = ct{2718};
t703 = ct{2719};
t704 = ct{2720};
t705 = ct{2721};
t706 = ct{2722};
t71 = ct{2723};
t710 = ct{2724};
t711 = ct{2725};
t712 = ct{2726};
t713 = ct{2727};
t715 = ct{2728};
t716 = ct{2729};
t72 = ct{2730};
t724 = ct{2731};
t728 = ct{2732};
t73 = ct{2733};
t731 = ct{2734};
t733 = ct{2735};
t734 = ct{2736};
t735 = ct{2737};
t736 = ct{2738};
t74 = ct{2739};
t741 = ct{2740};
t742 = ct{2741};
t743 = ct{2742};
t744 = ct{2743};
t746 = ct{2744};
t747 = ct{2745};
t748 = ct{2746};
t749 = ct{2747};
t75 = ct{2748};
t750 = ct{2749};
t751 = ct{2750};
t752 = ct{2751};
t754 = ct{2752};
t755 = ct{2753};
t756 = ct{2754};
t757 = ct{2755};
t758 = ct{2756};
t759 = ct{2757};
t76 = ct{2758};
t760 = ct{2759};
t762 = ct{2760};
t763 = ct{2761};
t764 = ct{2762};
t765 = ct{2763};
t766 = ct{2764};
t767 = ct{2765};
t768 = ct{2766};
t769 = ct{2767};
t77 = ct{2768};
t772 = ct{2769};
t773 = ct{2770};
t774 = ct{2771};
t775 = ct{2772};
t776 = ct{2773};
t777 = ct{2774};
t778 = ct{2775};
t779 = ct{2776};
t780 = ct{2777};
t781 = ct{2778};
t782 = ct{2779};
t784 = ct{2780};
t785 = ct{2781};
t786 = ct{2782};
t790 = ct{2783};
t792 = ct{2784};
t794 = ct{2785};
t795 = ct{2786};
t796 = ct{2787};
t798 = ct{2788};
t8 = ct{2789};
t80 = ct{2790};
t801 = ct{2791};
t804 = ct{2792};
t805 = ct{2793};
t806 = ct{2794};
t808 = ct{2795};
t81 = ct{2796};
t814 = ct{2797};
t815 = ct{2798};
t817 = ct{2799};
t82 = ct{2800};
t820 = ct{2801};
t822 = ct{2802};
t825 = ct{2803};
t827 = ct{2804};
t83 = ct{2805};
t831 = ct{2806};
t832 = ct{2807};
t833 = ct{2808};
t834 = ct{2809};
t835 = ct{2810};
t836 = ct{2811};
t837 = ct{2812};
t838 = ct{2813};
t84 = ct{2814};
t840 = ct{2815};
t841 = ct{2816};
t842 = ct{2817};
t843 = ct{2818};
t846 = ct{2819};
t86 = ct{2820};
t863 = ct{2821};
t868 = ct{2822};
t869 = ct{2823};
t870 = ct{2824};
t874 = ct{2825};
t878 = ct{2826};
t880 = ct{2827};
t881 = ct{2828};
t882 = ct{2829};
t884 = ct{2830};
t885 = ct{2831};
t888 = ct{2832};
t889 = ct{2833};
t891 = ct{2834};
t892 = ct{2835};
t895 = ct{2836};
t899 = ct{2837};
t9 = ct{2838};
t90 = ct{2839};
t900 = ct{2840};
t903 = ct{2841};
t906 = ct{2842};
t91 = ct{2843};
t911 = ct{2844};
t921 = ct{2845};
t922 = ct{2846};
t923 = ct{2847};
t925 = ct{2848};
t926 = ct{2849};
t927 = ct{2850};
t929 = ct{2851};
t934 = ct{2852};
t935 = ct{2853};
t936 = ct{2854};
t937 = ct{2855};
t940 = ct{2856};
t941 = ct{2857};
t942 = ct{2858};
t946 = ct{2859};
t949 = ct{2860};
t95 = ct{2861};
t950 = ct{2862};
t954 = ct{2863};
t955 = ct{2864};
t957 = ct{2865};
t958 = ct{2866};
t961 = ct{2867};
t962 = ct{2868};
t964 = ct{2869};
t965 = ct{2870};
t968 = ct{2871};
t97 = ct{2872};
t970 = ct{2873};
t971 = ct{2874};
t972 = ct{2875};
t973 = ct{2876};
t975 = ct{2877};
t977 = ct{2878};
t982 = ct{2879};
t983 = ct{2880};
t984 = ct{2881};
t986 = ct{2882};
t987 = ct{2883};
t988 = ct{2884};
t989 = ct{2885};
t99 = ct{2886};
t993 = ct{2887};
t994 = ct{2888};
t995 = ct{2889};
t999 = ct{2890};
t3123 = t4.*t8.*t9.*t17.*t194.*1.099250276973348e-6;
t3124 = t17.*t18.*t19.*t194.*(-1.57248917878546e-6);
t3126 = t194.*t1335;
t3127 = t4.*t7.*t8.*t9.*t194.*(-5.528690462784599e-13);
t3130 = t3.*t4.*t7.*t194.*1.569305128998788e-6;
t3131 = t9.*t18.*t194.*(-1.503068317813338e-13);
t3132 = t7.*t9.*t194.*(-1.812542008830624e-13);
t3133 = t9.*t23.*t194.*(-1.503068317813338e-13);
t3139 = t3.*t9.*t18.*t194.*(-2.764345231392299e-13);
t3140 = t5.*t7.*t18.*t194.*(-2.764345231392299e-13);
t3143 = t194.*t1326;
t3145 = t8.*t17.*t194.*1.569305128998788e-6;
t3146 = t194.*t1329;
t3147 = t194.*t1360;
t3148 = t3.*t7.*t194.*5.00036577347567e-6;
t3149 = t194.*t1362;
t3150 = t194.*t1364;
t3151 = t3.*t4.*t7.*t9.*t194.*3.968300857728448e-13;
t3152 = t3.*t5.*t7.*t8.*t194.*3.968300857728448e-13;
t3155 = t194.*t1372;
t3156 = t194.*t1375;
t3157 = t194.*t1378;
t3160 = t4.*t5.*t17.*t194.*3.968300857728448e-13;
t3162 = t2276.*(-1.232595164407831e-32);
t3163 = t5.*t17.*t18.*t194.*(-5.496251384866741e-7);
t3165 = t4.*t5.*t22.*t194.*3.968300857728448e-13;
t3167 = t7.*t18.*t194.*(-2.592703454263624e-7);
t3170 = t7.*t23.*t194.*(-2.592703454263624e-7);
t3171 = t4.*t8.*t9.*t194.*(-1.97108120739817e-13);
t3172 = t194.*t1389;
t3173 = t3.*t4.*t7.*t8.*t9.*t194.*7.936601715456896e-13;
t3174 = t3.*t4.*t9.*t194.*(-1.812542008830624e-13);
t3177 = t3.*t7.*t18.*t194.*7.443807831634578e-7;
t3178 = t4.*t8.*t17.*t194.*7.443807831634578e-7;
t3180 = t5.*t18.*t194.*(-1.97108120739817e-13);
t3181 = t194.*t1404;
t3182 = t5.*t23.*t194.*(-1.97108120739817e-13);
t3183 = t194.*t1382;
t3184 = t2276./8.112963841460668e+31;
t3186 = t9.*t17.*t18.*t194.*3.968300857728448e-13;
t3187 = t4.*t5.*t7.*t8.*t194.*(-7.250168035322496e-13);
t3190 = t9.*t17.*t23.*t194.*3.968300857728448e-13;
t3194 = t3.*t5.*t18.*t194.*(-3.625084017661248e-13);
t3197 = t4.*t9.*t17.*t194.*5.203917315847488e-13;
t3199 = t4.*t9.*t22.*t194.*5.203917315847488e-13;
t3206 = t3.*t4.*t5.*t7.*t194.*5.203917315847488e-13;
t3207 = t3.*t7.*t8.*t9.*t194.*5.203917315847488e-13;
t3234 = -t3211;
t3236 = -t3212;
t3240 = t3.*t4.*t194.*6.689200410011394e-6;
t3241 = t3.*t4.*t195.*6.689200410011394e-6;
t3242 = -t3219;
t3245 = -t3225;
t3250 = t5.*t17.*t18.*t194.*5.203917315847488e-13;
t3253 = t3.*t4.*t5.*t7.*t8.*t194.*1.040783463169498e-12;
t3254 = t5.*t17.*t23.*t194.*5.203917315847488e-13;
t3256 = -t3231;
t3260 = t8.*t3211;
t3262 = t9.*t3211;
t3263 = t5.*t3212;
t3264 = t9.*t3212;
t3265 = t4.*t8.*t9.*t17.*t194.*(-5.203917315847488e-13);
t3272 = -t3255;
t3276 = -t3258;
t3277 = t4.*t3208;
t3278 = t5.*t3208;
t3280 = t8.*t3208;
t3281 = t4.*t3211;
t3283 = t9.*t3208;
t3284 = t5.*t3211;
t3285 = -t3259;
t3287 = -t3261;
t3291 = t18.*t194.*3.483029800032151e-7;
t3292 = t23.*t194.*3.483029800032151e-7;
t3293 = t194.*t1456;
t3296 = t4.*t3252;
t3297 = t5.*t3251;
t3298 = t5.*t3252;
t3299 = t8.*t3252;
t3300 = t4.*t3255;
t3301 = t9.*t3251;
t3302 = t9.*t3252;
t3303 = t5.*t3255;
t3304 = t8.*t3255;
t3305 = t9.*t3255;
t3306 = t194.*t1461;
t3307 = t4.*t3257;
t3308 = t5.*t3257;
t3310 = t8.*t3257;
t3311 = t4.*t3258;
t3312 = t9.*t3257;
t3313 = t5.*t3258;
t3315 = t8.*t3258;
t3316 = t9.*t3258;
t3318 = -t3279;
t3324 = t4.*t7.*t8.*t194.*(-1.281152254279884e-6);
t3325 = -t3294;
t3338 = t9.*t3279;
t3339 = t5.*t3259;
t3342 = t5.*t3261;
t3345 = t9.*t3261;
t3346 = -t3319;
t3347 = -t3321;
t3348 = t5.*t3295;
t3350 = t9.*t3295;
t3362 = -t3330;
t3366 = t9.*t3286;
t3377 = t9.*t3327;
t3383 = t4.*t5.*t3279;
t3384 = t9.*t3334;
t3387 = t4.*t9.*t3259;
t3396 = t8.*t3321;
t3398 = -t3370;
t3399 = -t3372;
t3404 = -t3376;
t3405 = -t3379;
t3406 = t5.*t3363;
t3407 = -t3382;
t3408 = t4.*t5.*t3317;
t3410 = t4.*t9.*t3317;
t3411 = t4.*t5.*t3319;
t3412 = t9.*t3364;
t3413 = t4.*t3365;
t3414 = t4.*t9.*t3319;
t3415 = t5.*t8.*t3319;
t3421 = t8.*t9.*t3319;
t3422 = -t3389;
t3423 = t17.*t18.*t194.*9.195663283668398e-7;
t3424 = -t3394;
t3425 = t3.*t4.*t7.*t8.*t194.*1.83913265673368e-6;
t3427 = t17.*t23.*t194.*9.195663283668398e-7;
t3431 = t18.*t3321;
t3433 = t8.*t3375;
t3436 = -t3401;
t3441 = t8.*t3382;
t3451 = t8.*t3389;
t3457 = -t3419;
t3458 = t8.*t3394;
t3464 = t18.*t3365;
t3465 = t8.*t3400;
t3467 = -t3430;
t3471 = -t3434;
t3474 = -t3438;
t3476 = t4.*t9.*t3363;
t3480 = t4.*t5.*t3364;
t3485 = t8.*t3418;
t3487 = -t3450;
t3488 = -t3452;
t3490 = -t3456;
t3491 = -t3459;
t3493 = t8.*t3430;
t3494 = -t3463;
t3495 = t18.*t3394;
t3496 = -t3466;
t3497 = t8.*t3434;
t3498 = t23.*t3394;
t3499 = -t3470;
t3502 = -t3473;
t3503 = t8.*t3446;
t3504 = -t3477;
t3505 = t4.*t3449;
t3508 = t18.*t3376;
t3510 = t23.*t3376;
t3511 = -t3486;
t3512 = t17.*t3380;
t3513 = t18.*t3382;
t3518 = -t3492;
t3525 = t9.*t3473;
t3527 = t1472+2.61156643317655e-1;
t3528 = t1473+7.38843356682345e-1;
t3529 = -t3507;
t3531 = -t3509;
t3536 = -t3517;
t3542 = -t3519;
t3543 = -t3520;
t3545 = t5.*t196.*2.086042441322004e-7;
t3547 = -t3524;
t3550 = t1475-4.392651260556773e-1;
t3551 = t9.*t197.*2.086042441322004e-7;
t3552 = -t3534;
t3554 = t18.*t3449;
t3555 = t8.*t3519;
t3557 = -t3539;
t3558 = t8.*t3520;
t3559 = -t3541;
t3562 = t2.*t9.*t196.*1.769880715106441e-6;
t3563 = t2.*t5.*t197.*1.769880715106441e-6;
t3564 = t5.*t6.*t196.*1.769880715106441e-6;
t3567 = t6.*t9.*t197.*1.769880715106441e-6;
t3571 = -t3548;
t3577 = -t3553;
t3580 = t5.*t3544;
t3586 = t5.*t8.*t3472;
t3587 = -t3560;
t3589 = t2.*t5.*t196.*1.769880715106441e-6;
t3592 = t2.*t5.*t197.*8.849403575532204e-7;
t3593 = t5.*t6.*t196.*8.849403575532204e-7;
t3599 = -t3569;
t3603 = -t3575;
t3605 = -t3576;
t3606 = (t9.*t3444)./2.0;
t3608 = t196.*2.920111949661415e-10;
t3610 = -t3579;
t3611 = -t3582;
t3612 = -t3581;
t3614 = t9.*t196.*1.133811468776912e-7;
t3615 = t5.*t197.*1.133811468776912e-7;
t3619 = t2.*t5.*t196.*3.65040710056658e-6;
t3620 = t2.*t5.*t196.*7.30081420113316e-6;
t3625 = t5.*t6.*t196.*7.30081420113316e-6;
t3631 = -t3597;
t3633 = t2.*t9.*t197.*7.30081420113316e-6;
t3634 = t6.*t9.*t196.*7.30081420113316e-6;
t3635 = t5.*t6.*t197.*3.65040710056658e-6;
t3636 = t5.*t6.*t197.*7.30081420113316e-6;
t3642 = t5.*t3572;
t3644 = -t3601;
t3645 = t9.*t3572;
t3648 = t9.*t3573;
t3651 = t5.*t3575;
t3655 = -t3604;
t3656 = t2.*t197.*2.477538195427268e-9;
t3657 = t6.*t196.*2.477538195427268e-9;
t3658 = t8.*t9.*t3541;
t3661 = t8.*t3581;
t3666 = -t3613;
t3667 = t8.*t3585;
t3681 = -t3622;
t3687 = -t3629;
t3688 = t196.*1.004986427983203e-9;
t3690 = -t3639;
t3693 = t5.*t196.*6.367841787827598e-4;
t3694 = -t3641;
t3696 = -t3643;
t3699 = t9.*t196.*6.367841787827598e-4;
t3700 = t5.*t197.*6.367841787827598e-4;
t3702 = t5.*t3602;
t3704 = t9.*t197.*6.367841787827598e-4;
t3705 = -t3646;
t3706 = -t3647;
t3707 = -t3650;
t3708 = -t3649;
t3710 = t9.*t3602;
t3713 = -t3653;
t3715 = t9.*t3604;
t3720 = -t3654;
t3721 = t3.*t5.*t194.*3.367638735295547e-6;
t3723 = t2.*t196.*1.021992379861453e-8;
t3724 = t7.*t9.*t194.*3.367638735295547e-6;
t3725 = t6.*t197.*1.021992379861453e-8;
t3728 = t5.*t196.*1.170967356229242e-5;
t3732 = t9.*t196.*5.85483678114621e-6;
t3733 = t9.*t196.*1.170967356229242e-5;
t3734 = t5.*t197.*5.85483678114621e-6;
t3735 = t5.*t197.*1.170967356229242e-5;
t3745 = t5.*t3616;
t3746 = t5.*t3617;
t3749 = t9.*t3617;
t3752 = t9.*t3590;
t3757 = (t5.*t3515)./2.0;
t3758 = t5.*t3638;
t3766 = -t3680;
t3768 = -t3686;
t3769 = t9.*t3638;
t3770 = t5.*t3643;
t3773 = t9.*t3643;
t3776 = t2.*t5.*t196.*9.619703863182361e-7;
t3778 = -t3695;
t3780 = t2.*t9.*t196.*9.619703863182361e-7;
t3783 = t2.*t9.*t197.*4.809851931591181e-7;
t3784 = t2.*t9.*t197.*9.619703863182361e-7;
t3785 = t6.*t9.*t196.*4.809851931591181e-7;
t3786 = t6.*t9.*t196.*9.619703863182361e-7;
t3787 = t5.*t6.*t197.*9.619703863182361e-7;
t3792 = -t3714;
t3795 = -t3722;
t3800 = -t3737;
t3803 = t2.*t9.*t196.*1.984079208716435e-6;
t3804 = t2.*t9.*t196.*3.96815841743287e-6;
t3805 = t2.*t5.*t197.*3.96815841743287e-6;
t3806 = t5.*t6.*t196.*3.96815841743287e-6;
t3810 = -t3747;
t3811 = -t3748;
t3813 = t6.*t9.*t196.*3.96815841743287e-6;
t3814 = t5.*t3676;
t3816 = t4.*t9.*t194.*5.664363865215817e-6;
t3817 = t5.*t8.*t194.*5.664363865215817e-6;
t3819 = t6.*t9.*t197.*1.984079208716435e-6;
t3820 = t6.*t9.*t197.*3.96815841743287e-6;
t3821 = t9.*t3676;
t3823 = t5.*t3622;
t3826 = t3.*t9.*t194.*1.830388176740875e-6;
t3827 = t5.*t7.*t194.*1.830388176740875e-6;
t3831 = -t3751;
t3832 = t9.*t3629;
t3843 = -t3774;
t3849 = t5.*t3717;
t3850 = t9.*t3716;
t3851 = t9.*t3717;
t3853 = t5.*t3722;
t3855 = t4.*t5.*t7.*t194.*3.367638735295547e-6;
t3857 = t5.*t196.*3.182236832187144e-6;
t3858 = t5.*t196.*6.364473664374288e-6;
t3866 = t9.*t196.*6.364473664374288e-6;
t3867 = t197.*2.647396660368725e-7;
t3869 = t9.*t197.*3.182236832187144e-6;
t3870 = t9.*t197.*6.364473664374288e-6;
t3877 = -t3798;
t3885 = t5.*t3756;
t3890 = t9.*t3756;
t3891 = t5.*t3680;
t3912 = -t3847;
t3913 = -t3846;
t3917 = t3.*t5.*t8.*t194.*(-3.367638735295547e-6);
t3929 = t2.*t196.*2.246155783606385e-6;
t3930 = t196.*3.584310340215694e-6;
t3941 = t6.*t197.*2.246155783606385e-6;
t3946 = t4.*t7.*t9.*t194.*1.830388176740875e-6;
t3949 = t4.*t5.*t194.*3.078710474192051e-6;
t3952 = t8.*t9.*t194.*3.078710474192051e-6;
t3953 = -t3898;
t3966 = t8.*t194.*4.470006985551917e-6;
t3970 = t196.*8.369355329119605e-6;
t3980 = t2.*t197.*9.26546399593074e-6;
t3981 = t6.*t196.*9.26546399593074e-6;
t3982 = t3.*t8.*t9.*t194.*(-1.830388176740875e-6);
t3984 = t5.*t7.*t8.*t194.*(-1.830388176740875e-6);
t3990 = t7.*t194.*1.422428293644824e-6;
t4005 = t3.*t8.*t194.*2.657556793628188e-6;
t4006 = t4.*t7.*t194.*2.657556793628188e-6;
t4010 = -t4001;
t4011 = -t4002;
t4014 = t197.*7.425831767740348e-7;
t4015 = -t4007;
t4016 = t2.*t5.*t196.*1.857585372652597e-13;
t4017 = t2.*t9.*t196.*1.857585372652597e-13;
t4018 = t2.*t5.*t197.*1.857585372652597e-13;
t4019 = t5.*t6.*t196.*1.857585372652597e-13;
t4020 = t2.*t9.*t197.*1.857585372652597e-13;
t4021 = t6.*t9.*t196.*1.857585372652597e-13;
t4022 = t2.*t9.*t196.*7.662598700988556e-13;
t4023 = t5.*t6.*t196.*7.662598700988556e-13;
t4024 = t6.*t9.*t196.*7.662598700988556e-13;
t4025 = t5.*t6.*t197.*7.662598700988556e-13;
t4026 = t6.*t9.*t197.*7.662598700988556e-13;
t4027 = t3.*t194.*3.237047710821912e-7;
t4036 = t2.*t5.*t196.*7.662598700988556e-13;
t4046 = -t4029;
t4047 = -t4030;
t4048 = -t4031;
t4053 = -t4032;
t4054 = -t4033;
t4062 = t5.*t196.*1.228993465050726e-12;
t4063 = t9.*t196.*1.228993465050726e-12;
t4064 = t5.*t197.*1.228993465050726e-12;
t4065 = t9.*t197.*1.228993465050726e-12;
t4068 = -t4042;
t4069 = -t4043;
t4070 = -t4044;
t4071 = -t4045;
t4073 = -t4051;
t4074 = -t4052;
t4075 = -t4058;
t4089 = (t461.*t1460)./2.0;
t4099 = (t600.*t1427)./2.0;
t4103 = (t594.*t1429)./2.0;
t4116 = -t4105;
t4119 = t197+t2418;
t4124 = -t4117;
t4125 = t4.*t194.*5.749768960780552e-6;
t4132 = -t4123;
t4140 = t3.*t4.*t194.*3.4184146944075e-6;
t4142 = t7.*t8.*t194.*3.4184146944075e-6;
t4162 = t5.*t4144;
t4163 = t9.*t4144;
t4166 = -t4155;
t4169 = t5.*t4150;
t4171 = t9.*t4150;
t4173 = -t4160;
t4195 = -t4170;
t4201 = t8.*t4164;
t4202 = t8.*t4165;
t4210 = -t4181;
t4215 = -t4182;
t4217 = -t4185;
t4218 = -t4187;
t4219 = -t4189;
t4220 = t5.*t4174;
t4223 = -t4191;
t4224 = -t4192;
t4225 = -t4194;
t4226 = -t4193;
t4227 = t9.*t4174;
t4234 = -t4196;
t4241 = -t4200;
t4244 = -t4203;
t4245 = -t4204;
t4247 = -t4212;
t4248 = -t4213;
t4250 = t9.*t4182;
t4251 = t8.*t4184;
t4252 = t5.*t4187;
t4253 = t5.*t4188;
t4254 = t17.*t4153;
t4263 = -t4214;
t4264 = t9.*t4186;
t4267 = t8.*t4191;
t4269 = t8.*t4192;
t4270 = t8.*t4194;
t4273 = -t4216;
t4274 = -t4221;
t4276 = -t4230;
t4280 = -t4231;
t4281 = -t4236;
t4282 = -t4237;
t4285 = -t4240;
t4286 = -t4239;
t4291 = -t4242;
t4302 = t8.*t4205;
t4303 = t8.*t4207;
t4305 = t9.*t4204;
t4306 = t8.*t4209;
t4307 = t5.*t4212;
t4312 = t9.*t4211;
t4314 = t8.*t4214;
t4318 = -t4255;
t4322 = t8.*t4216;
t4324 = -t4265;
t4327 = -t4266;
t4329 = -t4268;
t4331 = -t4272;
t4332 = -t4271;
t4340 = t8.*t4229;
t4348 = t9.*t4231;
t4349 = t8.*t4232;
t4350 = t8.*t4233;
t4352 = t5.*t4236;
t4354 = -t4277;
t4356 = -t4278;
t4357 = -t4279;
t4358 = t9.*t4235;
t4359 = t8.*t4239;
t4360 = t8.*t4240;
t4362 = -t4288;
t4363 = -t4290;
t4364 = t5.*t4203;
t4366 = -t4294;
t4368 = t5.*t4246;
t4373 = t5.*t4256;
t4374 = -t4309;
t4376 = -t4311;
t4380 = t9.*t4256;
t4381 = t9.*t4257;
t4383 = t8.*t4261;
t4384 = t9.*t4258;
t4386 = t8.*t4262;
t4388 = -t4313;
t4389 = t8.*t22.*t4153;
t4393 = t8.*t4272;
t4398 = -t4319;
t4399 = -t4320;
t4400 = -t4321;
t4409 = -t4341;
t4414 = -t4342;
t4415 = -t4343;
t4416 = t3.*t4.*t7.*t4153;
t4418 = -t4345;
t4423 = -t4351;
t4424 = -t4353;
t4427 = t5.*t4283;
t4430 = -t4355;
t4433 = t9.*t4283;
t4434 = t8.*t4284;
t4437 = -t4361;
t4438 = t9.*t4287;
t4439 = t8.*t4290;
t4441 = t8.*t4294;
t4447 = -t4367;
t4451 = -t4375;
t4454 = t8.*t4317;
t4456 = t9.*t4319;
t4458 = t8.*t4320;
t4460 = t5.*t4325;
t4461 = -t4390;
t4463 = t5.*t4333;
t4465 = -t4394;
t4466 = -t4395;
t4467 = -t4396;
t4468 = -t4397;
t4470 = t8.*t4336;
t4471 = t9.*t4333;
t4472 = t9.*t4334;
t4474 = t8.*t4339;
t4475 = -t4402;
t4476 = -t4405;
t4477 = -t4406;
t4482 = -t4407;
t4487 = -t4410;
t4489 = -t4412;
t4490 = -t4413;
